simulink model "SIM_EXO_DAL_MN"  (R2021b)
(part 9 of 24)

t1621 = ct{452};
t1622 = ct{453};
t1623 = ct{454};
t1625 = ct{455};
t163 = ct{456};
t1631 = ct{457};
t1632 = ct{458};
t1633 = ct{459};
t1635 = ct{460};
t1636 = ct{461};
t1637 = ct{462};
t1638 = ct{463};
t1639 = ct{464};
t1641 = ct{465};
t1643 = ct{466};
t1644 = ct{467};
t1645 = ct{468};
t165 = ct{469};
t1650 = ct{470};
t1651 = ct{471};
t1652 = ct{472};
t1653 = ct{473};
t1657 = ct{474};
t1658 = ct{475};
t1659 = ct{476};
t166 = ct{477};
t1660 = ct{478};
t1661 = ct{479};
t1662 = ct{480};
t1663 = ct{481};
t1666 = ct{482};
t1669 = ct{483};
t1672 = ct{484};
t1676 = ct{485};
t168 = ct{486};
t1681 = ct{487};
t1682 = ct{488};
t1683 = ct{489};
t1687 = ct{490};
t1689 = ct{491};
t169 = ct{492};
t1692 = ct{493};
t1695 = ct{494};
t1696 = ct{495};
t1698 = ct{496};
t17 = ct{497};
t170 = ct{498};
t1702 = ct{499};
t1703 = ct{500};
t1704 = ct{501};
t1709 = ct{502};
t171 = ct{503};
t1711 = ct{504};
t1712 = ct{505};
t1713 = ct{506};
t1716 = ct{507};
t1720 = ct{508};
t1722 = ct{509};
t1726 = ct{510};
t1728 = ct{511};
t1729 = ct{512};
t173 = ct{513};
t1731 = ct{514};
t1733 = ct{515};
t1734 = ct{516};
t1735 = ct{517};
t1736 = ct{518};
t1737 = ct{519};
t1738 = ct{520};
t1740 = ct{521};
t1744 = ct{522};
t1745 = ct{523};
t1746 = ct{524};
t1749 = ct{525};
t175 = ct{526};
t1752 = ct{527};
t1755 = ct{528};
t1756 = ct{529};
t1757 = ct{530};
t1758 = ct{531};
t176 = ct{532};
t1760 = ct{533};
t1761 = ct{534};
t1764 = ct{535};
t1767 = ct{536};
t1769 = ct{537};
t177 = ct{538};
t1771 = ct{539};
t1772 = ct{540};
t1774 = ct{541};
t1776 = ct{542};
t1779 = ct{543};
t1784 = ct{544};
t1785 = ct{545};
t1786 = ct{546};
t1787 = ct{547};
t1788 = ct{548};
t1789 = ct{549};
t179 = ct{550};
t1793 = ct{551};
t1795 = ct{552};
t1797 = ct{553};
t1798 = ct{554};
t1799 = ct{555};
t18 = ct{556};
t180 = ct{557};
t1800 = ct{558};
t1801 = ct{559};
t1803 = ct{560};
t1804 = ct{561};
t1807 = ct{562};
t1808 = ct{563};
t1809 = ct{564};
t181 = ct{565};
t1810 = ct{566};
t1811 = ct{567};
t1812 = ct{568};
t1814 = ct{569};
t1816 = ct{570};
t1817 = ct{571};
t182 = ct{572};
t1820 = ct{573};
t1826 = ct{574};
t1827 = ct{575};
t1829 = ct{576};
t183 = ct{577};
t1830 = ct{578};
t1831 = ct{579};
t1832 = ct{580};
t1833 = ct{581};
t1834 = ct{582};
t1835 = ct{583};
t1836 = ct{584};
t1838 = ct{585};
t1847 = ct{586};
t1849 = ct{587};
t185 = ct{588};
t1850 = ct{589};
t1851 = ct{590};
t1855 = ct{591};
t1857 = ct{592};
t1858 = ct{593};
t1859 = ct{594};
t186 = ct{595};
t1866 = ct{596};
t1867 = ct{597};
t1871 = ct{598};
t1872 = ct{599};
t1873 = ct{600};
t1881 = ct{601};
t1882 = ct{602};
t1888 = ct{603};
t1889 = ct{604};
t1896 = ct{605};
t19 = ct{606};
t190 = ct{607};
t1903 = ct{608};
t1907 = ct{609};
t1908 = ct{610};
t191 = ct{611};
t1910 = ct{612};
t1911 = ct{613};
t1912 = ct{614};
t1913 = ct{615};
t1914 = ct{616};
t1915 = ct{617};
t1916 = ct{618};
t1920 = ct{619};
t1925 = ct{620};
t1926 = ct{621};
t193 = ct{622};
t1930 = ct{623};
t1935 = ct{624};
t1936 = ct{625};
t1937 = ct{626};
t1938 = ct{627};
t1939 = ct{628};
t194 = ct{629};
t1943 = ct{630};
t1944 = ct{631};
t1946 = ct{632};
t195 = ct{633};
t1950 = ct{634};
t1955 = ct{635};
t196 = ct{636};
t1961 = ct{637};
t1964 = ct{638};
t1965 = ct{639};
t1966 = ct{640};
t1967 = ct{641};
t1968 = ct{642};
t1969 = ct{643};
t197 = ct{644};
t1970 = ct{645};
t1972 = ct{646};
t1976 = ct{647};
t1977 = ct{648};
t1978 = ct{649};
t1979 = ct{650};
t198 = ct{651};
t1981 = ct{652};
t1984 = ct{653};
t1988 = ct{654};
t1992 = ct{655};
t1994 = ct{656};
t1995 = ct{657};
t1996 = ct{658};
t1997 = ct{659};
t1998 = ct{660};
t1999 = ct{661};
t2 = ct{662};
t20 = ct{663};
t2000 = ct{664};
t2001 = ct{665};
t2002 = ct{666};
t2003 = ct{667};
t2004 = ct{668};
t2005 = ct{669};
t2006 = ct{670};
t2014 = ct{671};
t2017 = ct{672};
t2019 = ct{673};
t2020 = ct{674};
t2023 = ct{675};
t2024 = ct{676};
t2028 = ct{677};
t2029 = ct{678};
t2033 = ct{679};
t2036 = ct{680};
t2037 = ct{681};
t2038 = ct{682};
t2042 = ct{683};
t2052 = ct{684};
t2053 = ct{685};
t2056 = ct{686};
t2058 = ct{687};
t2059 = ct{688};
t206 = ct{689};
t2060 = ct{690};
t2062 = ct{691};
t2065 = ct{692};
t2066 = ct{693};
t2067 = ct{694};
t2068 = ct{695};
t2069 = ct{696};
t207 = ct{697};
t2070 = ct{698};
t2072 = ct{699};
t2073 = ct{700};
t2074 = ct{701};
t2079 = ct{702};
t2081 = ct{703};
t2082 = ct{704};
t2083 = ct{705};
t2084 = ct{706};
t2085 = ct{707};
t2086 = ct{708};
t2087 = ct{709};
t2093 = ct{710};
t2094 = ct{711};
t2096 = ct{712};
t2097 = ct{713};
t2098 = ct{714};
t21 = ct{715};
t2100 = ct{716};
t2103 = ct{717};
t2104 = ct{718};
t2105 = ct{719};
t2106 = ct{720};
t2108 = ct{721};
t2109 = ct{722};
t2110 = ct{723};
t2111 = ct{724};
t2113 = ct{725};
t2114 = ct{726};
t2115 = ct{727};
t2116 = ct{728};
t2117 = ct{729};
t2118 = ct{730};
t2121 = ct{731};
t2122 = ct{732};
t2126 = ct{733};
t2128 = ct{734};
t2129 = ct{735};
t2130 = ct{736};
t2131 = ct{737};
t2132 = ct{738};
t2133 = ct{739};
t2136 = ct{740};
t2142 = ct{741};
t2144 = ct{742};
t2148 = ct{743};
t2149 = ct{744};
t215 = ct{745};
t2154 = ct{746};
t2156 = ct{747};
t2157 = ct{748};
t2158 = ct{749};
t216 = ct{750};
t2171 = ct{751};
t2172 = ct{752};
t2175 = ct{753};
t2176 = ct{754};
t2179 = ct{755};
t2180 = ct{756};
t2182 = ct{757};
t2189 = ct{758};
t219 = ct{759};
t2194 = ct{760};
t2196 = ct{761};
t22 = ct{762};
t220 = ct{763};
t2204 = ct{764};
t2208 = ct{765};
t221 = ct{766};
t2212 = ct{767};
t2214 = ct{768};
t2217 = ct{769};
t2218 = ct{770};
t2219 = ct{771};
t222 = ct{772};
t2220 = ct{773};
t2221 = ct{774};
t2223 = ct{775};
t2225 = ct{776};
t2227 = ct{777};
t2228 = ct{778};
t2229 = ct{779};
t223 = ct{780};
t2236 = ct{781};
t2239 = ct{782};
t224 = ct{783};
t2244 = ct{784};
t225 = ct{785};
t2251 = ct{786};
t2254 = ct{787};
t2256 = ct{788};
t2257 = ct{789};
t226 = ct{790};
t2264 = ct{791};
t2265 = ct{792};
t2266 = ct{793};
t2267 = ct{794};
t2269 = ct{795};
t227 = ct{796};
t2270 = ct{797};
t2274 = ct{798};
t2276 = ct{799};
t2277 = ct{800};
t2279 = ct{801};
t228 = ct{802};
t2280 = ct{803};
t2281 = ct{804};
t2282 = ct{805};
t2285 = ct{806};
t2291 = ct{807};
t2294 = ct{808};
t23 = ct{809};
t230 = ct{810};
t2302 = ct{811};
t2304 = ct{812};
t2305 = ct{813};
t2306 = ct{814};
t231 = ct{815};
t2316 = ct{816};
t2317 = ct{817};
t2318 = ct{818};
t2321 = ct{819};
t2322 = ct{820};
t2323 = ct{821};
t2324 = ct{822};
t233 = ct{823};
t2333 = ct{824};
t2336 = ct{825};
t2339 = ct{826};
t234 = ct{827};
t2340 = ct{828};
t2344 = ct{829};
t2348 = ct{830};
t235 = ct{831};
t2350 = ct{832};
t2357 = ct{833};
t2358 = ct{834};
t2359 = ct{835};
t236 = ct{836};
t2361 = ct{837};
t2362 = ct{838};
t2363 = ct{839};
t2364 = ct{840};
t2365 = ct{841};
t2366 = ct{842};
t2369 = ct{843};
t237 = ct{844};
t2371 = ct{845};
t2372 = ct{846};
t2373 = ct{847};
t2375 = ct{848};
t2376 = ct{849};
t2377 = ct{850};
t2378 = ct{851};
t2379 = ct{852};
t238 = ct{853};
t2384 = ct{854};
t2385 = ct{855};
t2387 = ct{856};
t2388 = ct{857};
t2389 = ct{858};
t239 = ct{859};
t2391 = ct{860};
t2394 = ct{861};
t24 = ct{862};
t240 = ct{863};
t2400 = ct{864};
t2401 = ct{865};
t2402 = ct{866};
t2403 = ct{867};
t2405 = ct{868};
t2406 = ct{869};
t2407 = ct{870};
t241 = ct{871};
t2410 = ct{872};
t2417 = ct{873};
t2418 = ct{874};
t2419 = ct{875};
t242 = ct{876};
t2421 = ct{877};
t2422 = ct{878};
t2428 = ct{879};
t2429 = ct{880};
t243 = ct{881};
t2430 = ct{882};
t2431 = ct{883};
t2434 = ct{884};
t2435 = ct{885};
t2437 = ct{886};
t2438 = ct{887};
t2439 = ct{888};
t244 = ct{889};
t2440 = ct{890};
t2441 = ct{891};
t2442 = ct{892};
t2443 = ct{893};
t2444 = ct{894};
t2447 = ct{895};
t2449 = ct{896};
t245 = ct{897};
t2450 = ct{898};
t2452 = ct{899};
t2453 = ct{900};
t2454 = ct{901};
t2455 = ct{902};
t2456 = ct{903};
t2457 = ct{904};
t2458 = ct{905};
t246 = ct{906};
t2460 = ct{907};
t2466 = ct{908};
t2467 = ct{909};
t2468 = ct{910};
t247 = ct{911};
t2470 = ct{912};
t2472 = ct{913};
t2474 = ct{914};
t2477 = ct{915};
t248 = ct{916};
t2481 = ct{917};
t2483 = ct{918};
t2484 = ct{919};
t2485 = ct{920};
t2486 = ct{921};
t2487 = ct{922};
t2489 = ct{923};
t249 = ct{924};
t2492 = ct{925};
t2495 = ct{926};
t2497 = ct{927};
t2498 = ct{928};
t2499 = ct{929};
t25 = ct{930};
t2500 = ct{931};
t2501 = ct{932};
t2502 = ct{933};
t2503 = ct{934};
t2504 = ct{935};
t2505 = ct{936};
t2506 = ct{937};
t2513 = ct{938};
t2518 = ct{939};
t2521 = ct{940};
t2527 = ct{941};
t253 = ct{942};
t2533 = ct{943};
t2535 = ct{944};
t2536 = ct{945};
t2537 = ct{946};
t2538 = ct{947};
t254 = ct{948};
t2540 = ct{949};
t2543 = ct{950};
t2544 = ct{951};
t2545 = ct{952};
t2546 = ct{953};
t2549 = ct{954};
t2551 = ct{955};
t2552 = ct{956};
t2553 = ct{957};
t2554 = ct{958};
t2555 = ct{959};
t2557 = ct{960};
t2558 = ct{961};
t2559 = ct{962};
t256 = ct{963};
t2560 = ct{964};
t2561 = ct{965};
t2562 = ct{966};
t2565 = ct{967};
t257 = ct{968};
t2572 = ct{969};
t2573 = ct{970};
t2574 = ct{971};
t2575 = ct{972};
t2576 = ct{973};
t2577 = ct{974};
t2578 = ct{975};
t2579 = ct{976};
t258 = ct{977};
t2583 = ct{978};
t2584 = ct{979};
t259 = ct{980};
t2590 = ct{981};
t2591 = ct{982};
t2592 = ct{983};
t2593 = ct{984};
t2595 = ct{985};
t2596 = ct{986};
t2597 = ct{987};
t26 = ct{988};
t260 = ct{989};
t2602 = ct{990};
t2603 = ct{991};
t2604 = ct{992};
t2605 = ct{993};
t2609 = ct{994};
t261 = ct{995};
t2610 = ct{996};
t2611 = ct{997};
t2615 = ct{998};
t2617 = ct{999};
t2627 = ct{1000};
t263 = ct{1001};
t264 = ct{1002};
t2652 = ct{1003};
t2655 = ct{1004};
t2656 = ct{1005};
t266 = ct{1006};
t2673 = ct{1007};
t2675 = ct{1008};
t2676 = ct{1009};
t2685 = ct{1010};
t2687 = ct{1011};
t269 = ct{1012};
t270 = ct{1013};
t2705 = ct{1014};
t2706 = ct{1015};
t2707 = ct{1016};
t2708 = ct{1017};
t2716 = ct{1018};
t2719 = ct{1019};
t272 = ct{1020};
t273 = ct{1021};
t274 = ct{1022};
t2749 = ct{1023};
t275 = ct{1024};
t2751 = ct{1025};
t2752 = ct{1026};
t276 = ct{1027};
t2764 = ct{1028};
t277 = ct{1029};
t278 = ct{1030};
t279 = ct{1031};
t280 = ct{1032};
t2804 = ct{1033};
t281 = ct{1034};
t284 = ct{1035};
t285 = ct{1036};
t2854 = ct{1037};
t286 = ct{1038};
t287 = ct{1039};
t288 = ct{1040};
t2886 = ct{1041};
t289 = ct{1042};
t29 = ct{1043};
t290 = ct{1044};
t291 = ct{1045};
t292 = ct{1046};
t293 = ct{1047};
t2939 = ct{1048};
t294 = ct{1049};
t296 = ct{1050};
t297 = ct{1051};
t299 = ct{1052};
t2997 = ct{1053};
t3 = ct{1054};
t30 = ct{1055};
t300 = ct{1056};
t302 = ct{1057};
t303 = ct{1058};
t304 = ct{1059};
t305 = ct{1060};
t3058 = ct{1061};
t306 = ct{1062};
t307 = ct{1063};
t308 = ct{1064};
t309 = ct{1065};
t31 = ct{1066};
t310 = ct{1067};
t311 = ct{1068};
t312 = ct{1069};
t313 = ct{1070};
t314 = ct{1071};
t3142 = ct{1072};
t315 = ct{1073};
t3158 = ct{1074};
t316 = ct{1075};
t318 = ct{1076};
t319 = ct{1077};
t3191 = ct{1078};
t32 = ct{1079};
t320 = ct{1080};
t3208 = ct{1081};
t321 = ct{1082};
t3211 = ct{1083};
t3212 = ct{1084};
t3218 = ct{1085};
t3219 = ct{1086};
t322 = ct{1087};
t3225 = ct{1088};
t3228 = ct{1089};
t3230 = ct{1090};
t3231 = ct{1091};
t324 = ct{1092};
t3243 = ct{1093};
t3244 = ct{1094};
t325 = ct{1095};
t3251 = ct{1096};
t3252 = ct{1097};
t3255 = ct{1098};
t3257 = ct{1099};
t3258 = ct{1100};
t3259 = ct{1101};
t3261 = ct{1102};
t3273 = ct{1103};
t3274 = ct{1104};
t3275 = ct{1105};
t3279 = ct{1106};
t328 = ct{1107};
t3282 = ct{1108};
t3286 = ct{1109};
t3288 = ct{1110};
t3289 = ct{1111};
t329 = ct{1112};
t3290 = ct{1113};
t3294 = ct{1114};
t3295 = ct{1115};
t33 = ct{1116};
t3309 = ct{1117};
t3314 = ct{1118};
t3317 = ct{1119};
t3319 = ct{1120};
t332 = ct{1121};
t3320 = ct{1122};
t3321 = ct{1123};
t3326 = ct{1124};
t3327 = ct{1125};
t3328 = ct{1126};
t3329 = ct{1127};
t333 = ct{1128};
t3330 = ct{1129};
t3331 = ct{1130};
t3333 = ct{1131};
t3334 = ct{1132};
t3335 = ct{1133};
t334 = ct{1134};
t3343 = ct{1135};
t336 = ct{1136};
t3363 = ct{1137};
t3364 = ct{1138};
t3365 = ct{1139};
t3367 = ct{1140};
t3368 = ct{1141};
t3369 = ct{1142};
t337 = ct{1143};
t3370 = ct{1144};
t3371 = ct{1145};
t3372 = ct{1146};
t3373 = ct{1147};
t3374 = ct{1148};
t3375 = ct{1149};
t3376 = ct{1150};
t3378 = ct{1151};
t3379 = ct{1152};
t3380 = ct{1153};
t3381 = ct{1154};
t3382 = ct{1155};
t3389 = ct{1156};
t3390 = ct{1157};
t3391 = ct{1158};
t3392 = ct{1159};
t3393 = ct{1160};
t3394 = ct{1161};
t3395 = ct{1162};
t3397 = ct{1163};
t34 = ct{1164};
t340 = ct{1165};
t3400 = ct{1166};
t3401 = ct{1167};
t3402 = ct{1168};
t3403 = ct{1169};
t3409 = ct{1170};
t341 = ct{1171};
t3416 = ct{1172};
t3417 = ct{1173};
t3418 = ct{1174};
t3419 = ct{1175};
t3420 = ct{1176};
t3426 = ct{1177};
t3430 = ct{1178};
t344 = ct{1179};
t345 = ct{1180};
t346 = ct{1181};
t347 = ct{1182};
t348 = ct{1183};
t349 = ct{1184};
t350 = ct{1185};
t352 = ct{1186};
t353 = ct{1187};
t354 = ct{1188};
t355 = ct{1189};
t356 = ct{1190};
t357 = ct{1191};
t358 = ct{1192};
t359 = ct{1193};
t360 = ct{1194};
t361 = ct{1195};
t362 = ct{1196};
t365 = ct{1197};
t366 = ct{1198};
t367 = ct{1199};
t368 = ct{1200};
t369 = ct{1201};
t371 = ct{1202};
t372 = ct{1203};
t373 = ct{1204};
t374 = ct{1205};
t375 = ct{1206};
t376 = ct{1207};
t377 = ct{1208};
t378 = ct{1209};
t379 = ct{1210};
t380 = ct{1211};
t382 = ct{1212};
t384 = ct{1213};
t386 = ct{1214};
t387 = ct{1215};
t388 = ct{1216};
t389 = ct{1217};
t391 = ct{1218};
t392 = ct{1219};
t395 = ct{1220};
t396 = ct{1221};
t398 = ct{1222};
t4 = ct{1223};
t400 = ct{1224};
t401 = ct{1225};
t402 = ct{1226};
t403 = ct{1227};
t404 = ct{1228};
t406 = ct{1229};
t409 = ct{1230};
t410 = ct{1231};
t411 = ct{1232};
t412 = ct{1233};
t413 = ct{1234};
t414 = ct{1235};
t415 = ct{1236};
t416 = ct{1237};
t417 = ct{1238};
t418 = ct{1239};
t419 = ct{1240};
t420 = ct{1241};
t421 = ct{1242};
t422 = ct{1243};
t423 = ct{1244};
t424 = ct{1245};
t425 = ct{1246};
t426 = ct{1247};
t427 = ct{1248};
t428 = ct{1249};
t429 = ct{1250};
t431 = ct{1251};
t432 = ct{1252};
t433 = ct{1253};
t434 = ct{1254};
t435 = ct{1255};
t436 = ct{1256};
t437 = ct{1257};
t438 = ct{1258};
t439 = ct{1259};
t44 = ct{1260};
t440 = ct{1261};
t441 = ct{1262};
t442 = ct{1263};
t443 = ct{1264};
t444 = ct{1265};
t445 = ct{1266};
t448 = ct{1267};
t449 = ct{1268};
t45 = ct{1269};
t450 = ct{1270};
t452 = ct{1271};
t453 = ct{1272};
t454 = ct{1273};
t457 = ct{1274};
t458 = ct{1275};
t459 = ct{1276};
t46 = ct{1277};
t460 = ct{1278};
t461 = ct{1279};
t462 = ct{1280};
t463 = ct{1281};
t464 = ct{1282};
t465 = ct{1283};
t466 = ct{1284};
t468 = ct{1285};
t469 = ct{1286};
t47 = ct{1287};
t470 = ct{1288};
t471 = ct{1289};
t472 = ct{1290};
t475 = ct{1291};
t4763 = ct{1292};
t477 = ct{1293};
t479 = ct{1294};
t480 = ct{1295};
t481 = ct{1296};
t482 = ct{1297};
t483 = ct{1298};
t484 = ct{1299};
t485 = ct{1300};
t486 = ct{1301};
t488 = ct{1302};
t489 = ct{1303};
t491 = ct{1304};
t492 = ct{1305};
t493 = ct{1306};
t494 = ct{1307};
t496 = ct{1308};
t497 = ct{1309};
t498 = ct{1310};
t499 = ct{1311};
t5 = ct{1312};
t50 = ct{1313};
t500 = ct{1314};
t501 = ct{1315};
t502 = ct{1316};
t503 = ct{1317};
t504 = ct{1318};
t505 = ct{1319};
t506 = ct{1320};
t507 = ct{1321};
t508 = ct{1322};
t509 = ct{1323};
t510 = ct{1324};
t511 = ct{1325};
t512 = ct{1326};
t513 = ct{1327};
t514 = ct{1328};
t516 = ct{1329};
t517 = ct{1330};
t518 = ct{1331};
t520 = ct{1332};
t521 = ct{1333};
t522 = ct{1334};
t523 = ct{1335};
t524 = ct{1336};
t525 = ct{1337};
t526 = ct{1338};
t527 = ct{1339};
t528 = ct{1340};
t529 = ct{1341};
t53 = ct{1342};
t530 = ct{1343};
t531 = ct{1344};
t532 = ct{1345};
t533 = ct{1346};
t534 = ct{1347};
t535 = ct{1348};
t536 = ct{1349};
t5361 = ct{1350};
t537 = ct{1351};
t538 = ct{1352};
t539 = ct{1353};
t540 = ct{1354};
t543 = ct{1355};
t544 = ct{1356};
t545 = ct{1357};
t546 = ct{1358};
t547 = ct{1359};
t548 = ct{1360};
t549 = ct{1361};
t551 = ct{1362};
t552 = ct{1363};
t553 = ct{1364};
t554 = ct{1365};
t555 = ct{1366};
t556 = ct{1367};
t557 = ct{1368};
t558 = ct{1369};
t559 = ct{1370};
t560 = ct{1371};
t561 = ct{1372};
t562 = ct{1373};
t563 = ct{1374};
t564 = ct{1375};
t567 = ct{1376};
t568 = ct{1377};
t569 = ct{1378};
t57 = ct{1379};
t570 = ct{1380};
t571 = ct{1381};
t572 = ct{1382};
t573 = ct{1383};
t574 = ct{1384};
t576 = ct{1385};
t577 = ct{1386};
t5777 = ct{1387};
t578 = ct{1388};
t579 = ct{1389};
t58 = ct{1390};
t580 = ct{1391};
t581 = ct{1392};
t582 = ct{1393};
t583 = ct{1394};
t584 = ct{1395};
t586 = ct{1396};
t587 = ct{1397};
t589 = ct{1398};
t59 = ct{1399};
t590 = ct{1400};
t591 = ct{1401};
t592 = ct{1402};
t593 = ct{1403};
t594 = ct{1404};
t595 = ct{1405};
t596 = ct{1406};
t597 = ct{1407};
t6 = ct{1408};
t60 = ct{1409};
t600 = ct{1410};
t602 = ct{1411};
t603 = ct{1412};
t604 = ct{1413};
t605 = ct{1414};
t609 = ct{1415};
t610 = ct{1416};
t611 = ct{1417};
t612 = ct{1418};
t613 = ct{1419};
t614 = ct{1420};
t615 = ct{1421};
t617 = ct{1422};
t618 = ct{1423};
t623 = ct{1424};
t625 = ct{1425};
t626 = ct{1426};
t629 = ct{1427};
t63 = ct{1428};
t633 = ct{1429};
t634 = ct{1430};
t638 = ct{1431};
t640 = ct{1432};
t643 = ct{1433};
t644 = ct{1434};
t655 = ct{1435};
t656 = ct{1436};
t660 = ct{1437};
t662 = ct{1438};
t663 = ct{1439};
t664 = ct{1440};
t665 = ct{1441};
t667 = ct{1442};
t668 = ct{1443};
t673 = ct{1444};
t674 = ct{1445};
t675 = ct{1446};
t676 = ct{1447};
t681 = ct{1448};
t682 = ct{1449};
t683 = ct{1450};
t685 = ct{1451};
t686 = ct{1452};
t687 = ct{1453};
t688 = ct{1454};
t689 = ct{1455};
t693 = ct{1456};
t694 = ct{1457};
t695 = ct{1458};
t696 = ct{1459};
t697 = ct{1460};
t698 = ct{1461};
t7 = ct{1462};
t700 = ct{1463};
t702 = ct{1464};
t703 = ct{1465};
t704 = ct{1466};
t705 = ct{1467};
t706 = ct{1468};
t71 = ct{1469};
t711 = ct{1470};
t713 = ct{1471};
t715 = ct{1472};
t716 = ct{1473};
t72 = ct{1474};
t724 = ct{1475};
t725 = ct{1476};
t727 = ct{1477};
t728 = ct{1478};
t73 = ct{1479};
t731 = ct{1480};
t733 = ct{1481};
t734 = ct{1482};
t735 = ct{1483};
t736 = ct{1484};
t74 = ct{1485};
t744 = ct{1486};
t746 = ct{1487};
t747 = ct{1488};
t748 = ct{1489};
t749 = ct{1490};
t75 = ct{1491};
t750 = ct{1492};
t751 = ct{1493};
t752 = ct{1494};
t755 = ct{1495};
t756 = ct{1496};
t757 = ct{1497};
t758 = ct{1498};
t759 = ct{1499};
t76 = ct{1500};
t762 = ct{1501};
t763 = ct{1502};
t764 = ct{1503};
t765 = ct{1504};
t766 = ct{1505};
t768 = ct{1506};
t769 = ct{1507};
t77 = ct{1508};
t772 = ct{1509};
t774 = ct{1510};
t775 = ct{1511};
t776 = ct{1512};
t780 = ct{1513};
t782 = ct{1514};
t785 = ct{1515};
t786 = ct{1516};
t788 = ct{1517};
t791 = ct{1518};
t793 = ct{1519};
t795 = ct{1520};
t8 = ct{1521};
t80 = ct{1522};
t804 = ct{1523};
t805 = ct{1524};
t806 = ct{1525};
t808 = ct{1526};
t81 = ct{1527};
t814 = ct{1528};
t815 = ct{1529};
t816 = ct{1530};
t818 = ct{1531};
t819 = ct{1532};
t82 = ct{1533};
t820 = ct{1534};
t821 = ct{1535};
t822 = ct{1536};
t825 = ct{1537};
t827 = ct{1538};
t83 = ct{1539};
t833 = ct{1540};
t834 = ct{1541};
t835 = ct{1542};
t836 = ct{1543};
t837 = ct{1544};
t838 = ct{1545};
t84 = ct{1546};
t840 = ct{1547};
t841 = ct{1548};
t842 = ct{1549};
t843 = ct{1550};
t846 = ct{1551};
t851 = ct{1552};
t855 = ct{1553};
t857 = ct{1554};
t86 = ct{1555};
t862 = ct{1556};
t864 = ct{1557};
t874 = ct{1558};
t880 = ct{1559};
t882 = ct{1560};
t884 = ct{1561};
t885 = ct{1562};
t888 = ct{1563};
t891 = ct{1564};
t892 = ct{1565};
t895 = ct{1566};
t897 = ct{1567};
t899 = ct{1568};
t9 = ct{1569};
t90 = ct{1570};
t900 = ct{1571};
t903 = ct{1572};
t904 = ct{1573};
t906 = ct{1574};
t91 = ct{1575};
t911 = ct{1576};
t921 = ct{1577};
t922 = ct{1578};
t923 = ct{1579};
t926 = ct{1580};
t927 = ct{1581};
t934 = ct{1582};
t935 = ct{1583};
t936 = ct{1584};
t937 = ct{1585};
t940 = ct{1586};
t941 = ct{1587};
t942 = ct{1588};
t946 = ct{1589};
t949 = ct{1590};
t95 = ct{1591};
t950 = ct{1592};
t956 = ct{1593};
t957 = ct{1594};
t958 = ct{1595};
t961 = ct{1596};
t962 = ct{1597};
t964 = ct{1598};
t965 = ct{1599};
t966 = ct{1600};
t968 = ct{1601};
t969 = ct{1602};
t97 = ct{1603};
t970 = ct{1604};
t971 = ct{1605};
t972 = ct{1606};
t977 = ct{1607};
t979 = ct{1608};
t982 = ct{1609};
t983 = ct{1610};
t984 = ct{1611};
t986 = ct{1612};
t987 = ct{1613};
t988 = ct{1614};
t989 = ct{1615};
t99 = ct{1616};
t993 = ct{1617};
t994 = ct{1618};
t995 = ct{1619};
t997 = ct{1620};
t999 = ct{1621};
t3432 = t3.*t5.*t8.*t9.*t34.*t191.*4.649924393989671e-23;
t3434 = t4.*t5.*t7.*t9.*t34.*t191.*9.299848787979342e-23;
t3435 = t5.*t7.*t8.*t9.*t34.*t191.*1.414846738462756e-22;
t3437 = t4.*t19.*t34.*t191.*7.821166634427942e-23;
t3438 = t4.*t24.*t34.*t191.*7.821166634427942e-23;
t3439 = t4.*t9.*t34.*t191.*2.079476307604284e-23;
t3440 = t4.*t9.*t34.*t191.*4.158952615208568e-23;
t3442 = t8.*t9.*t34.*t191.*4.158952615208568e-23;
t3443 = t101+t124+t139+t180;
t3444 = t108+t122+t141+t182;
t3445 = t3.*t4.*t5.*t8.*t34.*t191.*9.098517085411002e-23;
t3446 = t3.*t5.*t34.*t191.*(-2.472625392454631e-23);
t3447 = t4.*t5.*t7.*t34.*t191.*(-2.47393392290267e-21);
t3449 = t7.*t9.*t34.*t191.*(-2.472625392454631e-23);
t3450 = t3.*t4.*t19.*t34.*t191.*4.649924393989671e-23;
t3452 = t3.*t8.*t19.*t34.*t191.*1.414846738462756e-22;
t3453 = t4.*t7.*t19.*t34.*t191.*1.414846738462756e-22;
t3454 = t4.*t7.*t9.*t34.*t191.*(-2.47393392290267e-21);
t3455 = t5.*t7.*t8.*t34.*t191.*(-2.47393392290267e-21);
t3456 = t3.*t4.*t24.*t34.*t191.*4.649924393989671e-23;
t3459 = t7.*t8.*t24.*t34.*t191.*4.649924393989671e-23;
t3462 = t17.*t34.*t191.*3.230367166673482e-25;
t3463 = t18.*t19.*t34.*t191.*1.189885164369265e-22;
t3466 = t18.*t24.*t34.*t191.*1.189885164369265e-22;
t3468 = t9.*t18.*t34.*t191.*(-7.651846806710377e-23);
t3469 = t4.*t8.*t19.*t34.*t191.*1.564233326885588e-22;
t3470 = t5.*t9.*t18.*t34.*t191.*1.564233326885588e-22;
t3472 = t4.*t34.*t191.*3.002769355787804e-29;
t3473 = t8.*t34.*t191.*3.002769355787804e-29;
t3475 = t3.*t4.*t9.*t34.*t191.*1.236312696227316e-23;
t3477 = t3.*t5.*t8.*t34.*t191.*1.236312696227316e-23;
t3479 = t4.*t5.*t7.*t34.*t191.*1.236312696227316e-23;
t3481 = t5.*t8.*t34.*t191.*(-4.158952615208568e-23);
t3483 = t7.*t8.*t9.*t34.*t191.*1.236312696227316e-23;
t3486 = t4.*t17.*t34.*t191.*3.356793907564468e-24;
t3489 = t3.*t8.*t19.*t34.*t191.*(-7.074233692313782e-23);
t3492 = t3.*t9.*t34.*t191.*1.785238843466173e-29;
t3500 = t3.*t4.*t8.*t9.*t34.*t191.*4.945250784909262e-23;
t3501 = t4.*t8.*t9.*t34.*t191.*8.317905230417136e-23;
t3506 = t3.*t4.*t8.*t19.*t34.*t191.*9.299848787979342e-23;
t3507 = t4.*t7.*t8.*t19.*t34.*t191.*7.074233692313782e-23;
t3509 = t4.*t7.*t8.*t24.*t34.*t191.*7.074233692313782e-23;
t3514 = t102+t129+t150+t179;
t3515 = t117+t123+t153+t181;
t3516 = t3.*t8.*t34.*t191.*7.059909452387201e-23;
t3517 = t4.*t7.*t34.*t191.*7.059909452387201e-23;
t3519 = t3.*t9.*t34.*t191.*8.926194217330866e-30;
t3520 = t5.*t7.*t34.*t191.*8.926194217330866e-30;
t3521 = t7.*t18.*t19.*t34.*t191.*(-4.649924393989671e-23);
t3522 = t4.*t5.*t7.*t8.*t9.*t34.*t191.*(-9.299848787979342e-23);
t3523 = t130+t134+t152+t176;
t3524 = t8.*t9.*t34.*t191.*1.501384677893902e-29;
t3530 = t5.*t7.*t9.*t18.*t34.*t191.*(-7.074233692313782e-23);
t3532 = t4.*t17.*t34.*t191.*(-1.678396953782234e-24);
t3533 = t5.*t18.*t34.*t191.*(-4.158952615208568e-23);
t3534 = t3.*t4.*t5.*t34.*t191.*1.785238843466173e-29;
t3535 = t3.*t8.*t34.*t191.*3.5299547261936e-23;
t3538 = t4.*t7.*t9.*t34.*t191.*1.785238843466173e-29;
t3539 = t5.*t7.*t8.*t34.*t191.*1.785238843466173e-29;
t3541 = t4.*t34.*t191.*3.937746659416635e-29;
t3544 = t8.*t34.*t191.*3.937746659416635e-29;
t3546 = t8.*t9.*t34.*t191.*(-3.002769355787804e-29);
t3548 = t4.*t8.*t34.*t191.*5.632647031707275e-23;
t3549 = t4.*t5.*t7.*t8.*t34.*t191.*(-2.472625392454631e-23);
t3553 = t3.*t4.*t5.*t34.*t191.*8.926194217330866e-30;
t3556 = t4.*t7.*t9.*t34.*t191.*8.926194217330866e-30;
t3560 = t7.*t34.*t191.*1.323536528500358e-22;
t3568 = t3.*t9.*t18.*t34.*t191.*3.570477686932346e-29;
t3569 = t5.*t7.*t18.*t34.*t191.*1.785238843466173e-29;
t3572 = t2.*t4.*t190.*2.976937004352228e-6;
t3573 = t2.*t8.*t190.*2.976937004352228e-6;
t3574 = t9.*t18.*t34.*t191.*3.002769355787804e-29;
t3575 = t6.*t8.*t190.*2.976937004352228e-6;
t3576 = t9.*t23.*t34.*t191.*3.002769355787804e-29;
t3578 = t4.*t7.*t8.*t9.*t34.*t191.*3.570477686932346e-29;
t3579 = t5.*t8.*t34.*t191.*1.968873329708317e-29;
t3581 = t3.*t5.*t34.*t191.*1.170555820174774e-29;
t3582 = t3.*t5.*t34.*t191.*2.341111640349547e-29;
t3583 = t3.*t8.*t9.*t34.*t191.*(-8.926194217330866e-30);
t3584 = t5.*t7.*t8.*t34.*t191.*(-8.926194217330866e-30);
t3585 = t7.*t9.*t34.*t191.*1.170555820174774e-29;
t3590 = t6.*t8.*t190.*1.22799597575967e-5;
t3596 = t4.*t9.*t190.*3.508720606545093e-7;
t3597 = t5.*t8.*t190.*3.508720606545093e-7;
t3601 = t3.*t4.*t8.*t34.*t191.*3.34878210114812e-23;
t3602 = t4.*t190.*6.800564119502148e-6;
t3604 = t8.*t190.*6.800564119502148e-6;
t3607 = t7.*t18.*t34.*t191.*1.67439105057406e-23;
t3609 = t5.*t8.*t34.*t191.*(-3.937746659416635e-29);
t3613 = t7.*t23.*t34.*t191.*1.67439105057406e-23;
t3616 = t2.*t8.*t190.*1.22799597575967e-5;
t3617 = t4.*t6.*t190.*1.22799597575967e-5;
t3618 = t4.*t5.*t8.*t34.*t191.*(-3.002769355787804e-29);
t3622 = t2.*t8.*t190.*1.618032907912407e-6;
t3629 = t6.*t8.*t190.*1.618032907912407e-6;
t3630 = t4.*t190.*3.147703918772038e-6;
t3637 = t5.*t18.*t34.*t191.*3.937746659416635e-29;
t3638 = t4.*t190.*3.698217217635989e-4;
t3639 = t8.*t190.*3.147703918772038e-6;
t3641 = t5.*t23.*t34.*t191.*3.937746659416635e-29;
t3643 = t8.*t190.*3.698217217635989e-4;
t3646 = t4.*t5.*t34.*t191.*8.031026374039477e-30;
t3647 = t2.*t8.*t9.*t190.*1.488468502176114e-6;
t3649 = t4.*t6.*t9.*t190.*1.488468502176114e-6;
t3650 = t4.*t6.*t9.*t190.*2.976937004352228e-6;
t3652 = t4.*t9.*t34.*t191.*8.031026374039477e-30;
t3653 = t5.*t8.*t34.*t191.*8.031026374039477e-30;
t3654 = t8.*t9.*t34.*t191.*8.031026374039477e-30;
t3659 = t3.*t4.*t9.*t34.*t191.*1.170555820174774e-29;
t3660 = t3.*t4.*t9.*t34.*t191.*2.341111640349547e-29;
t3662 = t4.*t5.*t7.*t34.*t191.*1.170555820174774e-29;
t3663 = t4.*t5.*t7.*t34.*t191.*2.341111640349547e-29;
t3668 = t7.*t8.*t9.*t34.*t191.*2.341111640349547e-29;
t3676 = t2.*t4.*t190.*1.618032907912407e-6;
t3680 = t8.*t190.*3.696261130697717e-6;
t3682 = t3.*t5.*t18.*t34.*t191.*4.682223280699094e-29;
t3686 = t4.*t5.*t190.*1.907069379620846e-7;
t3691 = t4.*t190.*6.903101118415674e-6;
t3695 = t8.*t9.*t190.*1.907069379620846e-7;
t3697 = t8.*t190.*6.903101118415674e-6;
t3701 = t2.*t4.*t9.*t190.*(-2.976937004352228e-6);
t3709 = t5.*t6.*t8.*t190.*(-2.976937004352228e-6);
t3714 = t8.*t9.*t190.*3.400282059751074e-6;
t3716 = t2.*t8.*t190.*6.674437170347525e-6;
t3717 = t4.*t6.*t190.*6.674437170347525e-6;
t3722 = t6.*t8.*t190.*6.674437170347525e-6;
t3726 = t4.*t5.*t7.*t8.*t34.*t191.*4.682223280699094e-29;
t3729 = t3.*t4.*t5.*t34.*t191.*4.774692471202153e-30;
t3730 = t4.*t8.*t9.*t34.*t191.*(-3.937746659416635e-29);
t3736 = t3.*t4.*t9.*t34.*t191.*4.774692471202153e-30;
t3737 = t4.*t5.*t7.*t34.*t191.*4.774692471202153e-30;
t3738 = t3.*t5.*t8.*t34.*t191.*(-1.170555820174774e-29);
t3743 = t2.*t4.*t9.*t190.*6.139979878798348e-6;
t3744 = t2.*t4.*t9.*t190.*1.22799597575967e-5;
t3747 = t4.*t7.*t9.*t34.*t191.*4.774692471202153e-30;
t3748 = t5.*t7.*t8.*t34.*t191.*4.774692471202153e-30;
t3750 = t7.*t8.*t9.*t34.*t191.*4.774692471202153e-30;
t3751 = t6.*t8.*t9.*t190.*6.139979878798348e-6;
t3756 = t4.*t190.*3.696261130697717e-6;
t3774 = t7.*t9.*t18.*t34.*t191.*2.341111640349547e-29;
t3789 = t4.*t9.*t190.*(-6.800564119502148e-6);
t3798 = t8.*t190.*2.768890910755245e-7;
t3815 = t4.*t6.*t9.*t190.*(-1.22799597575967e-5);
t3822 = t2.*t5.*t8.*t190.*8.090164539562037e-7;
t3824 = t4.*t5.*t6.*t190.*8.090164539562037e-7;
t3825 = t4.*t5.*t6.*t190.*1.618032907912407e-6;
t3834 = t4.*t9.*t190.*(-3.698217217635989e-4);
t3835 = t5.*t8.*t190.*(-3.698217217635989e-4);
t3839 = t8.*t9.*t190.*(-3.698217217635989e-4);
t3846 = t2.*t4.*t5.*t190.*3.337218585173762e-6;
t3847 = t2.*t4.*t5.*t190.*6.674437170347525e-6;
t3852 = t5.*t6.*t8.*t190.*3.337218585173762e-6;
t3889 = t2.*t4.*t190.*2.349236299369594e-6;
t3892 = t2.*t5.*t8.*t190.*(-1.618032907912407e-6);
t3898 = t6.*t8.*t190.*2.349236299369594e-6;
t3899 = t6.*t8.*t9.*t190.*(-1.618032907912407e-6);
t3915 = t5.*t6.*t8.*t190.*(-6.674437170347525e-6);
t3950 = t5.*t8.*t190.*(-3.696261130697717e-6);
t3951 = t5.*t8.*t190.*1.848130565348858e-6;
t3958 = t2.*t8.*t190.*9.690674399615435e-6;
t3959 = t4.*t6.*t190.*9.690674399615435e-6;
t4001 = t3.*t18.*t34.*t191.*8.273795699471084e-23;
t4002 = t18.*t34.*t191.*6.958256670626673e-23;
t4004 = t23.*t34.*t191.*6.958256670626673e-23;
t4007 = t4.*t7.*t8.*t34.*t191.*8.273795699471084e-23;
t4028 = t2.*t4.*t5.*t190.*3.124456121473909e-13;
t4029 = t2.*t4.*t9.*t190.*3.124456121473909e-13;
t4030 = t2.*t5.*t8.*t190.*3.124456121473909e-13;
t4031 = t4.*t5.*t6.*t190.*3.124456121473909e-13;
t4032 = t2.*t8.*t9.*t190.*3.124456121473909e-13;
t4033 = t4.*t6.*t9.*t190.*3.124456121473909e-13;
t4039 = t2.*t4.*t5.*t190.*1.288848080425708e-12;
t4040 = t2.*t4.*t9.*t190.*1.288848080425708e-12;
t4041 = t4.*t5.*t6.*t190.*1.288848080425708e-12;
t4042 = t4.*t6.*t9.*t190.*1.288848080425708e-12;
t4043 = t5.*t6.*t8.*t190.*1.288848080425708e-12;
t4044 = t6.*t8.*t9.*t190.*1.288848080425708e-12;
t4045 = t4.*t5.*t190.*7.137559230037459e-13;
t4051 = t4.*t9.*t190.*7.137559230037459e-13;
t4052 = t5.*t8.*t190.*7.137559230037459e-13;
t4058 = t8.*t9.*t190.*7.137559230037459e-13;
t4105 = t4.*t190.*3.561623743745041e-7;
t4113 = t2.*t8.*t190.*3.021822113324163e-6;
t4114 = t4.*t6.*t190.*3.021822113324163e-6;
t4117 = t2.*t4.*t190.*1.246511225866906e-5;
t4118 = t6.*t8.*t190.*1.246511225866906e-5;
t4123 = (t498.*t1471)./2.0;
t4143 = t2.*t8.*t34.*t191.*2.473154649626116e-18;
t4144 = t4.*t34.*t191.*5.649715377798866e-18;
t4145 = t8.*t34.*t191.*5.649715377798866e-18;
t4150 = t3.*t34.*t191.*9.728063971071188e-18;
t4152 = t6.*t8.*t34.*t191.*1.020184153286453e-17;
t4153 = t9.*t34.*t191.*3.910360575273795e-23;
t4155 = t4.*t6.*t7.*t34.*t191.*6.065308926991484e-18;
t4160 = t2.*t4.*t7.*t34.*t191.*1.470366592725919e-18;
t4164 = t3.*t9.*t34.*t191.*4.531926220025415e-23;
t4165 = t5.*t7.*t34.*t191.*4.531926220025415e-23;
t4170 = t4.*t7.*t34.*t191.*9.728063971071188e-18;
t4174 = t7.*t8.*t34.*t191.*9.728063971071188e-18;
t4177 = t7.*t34.*t191.*6.343941833557992e-26;
t4178 = t3.*t7.*t34.*t191.*1.261825515365316e-22;
t4179 = t5.*t9.*t34.*t191.*7.993777824483687e-23;
t4180 = t4.*t9.*t34.*t191.*(-5.649715377798866e-18);
t4181 = t4.*t8.*t34.*t191.*1.628350277673685e-22;
t4182 = t2.*t3.*t4.*t34.*t191.*3.84506501891928e-22;
t4183 = t2.*t3.*t5.*t34.*t191.*1.92253250945964e-22;
t4184 = t2.*t3.*t5.*t34.*t191.*3.84506501891928e-22;
t4185 = t19.*t34.*t191.*6.080728160647903e-23;
t4186 = t2.*t3.*t8.*t34.*t191.*3.84506501891928e-22;
t4187 = t2.*t4.*t7.*t34.*t191.*3.84506501891928e-22;
t4188 = t3.*t4.*t6.*t34.*t191.*3.84506501891928e-22;
t4189 = t2.*t5.*t7.*t34.*t191.*3.84506501891928e-22;
t4190 = t24.*t34.*t191.*6.080728160647903e-23;
t4191 = t2.*t7.*t9.*t34.*t191.*3.84506501891928e-22;
t4192 = t3.*t6.*t9.*t34.*t191.*3.84506501891928e-22;
t4193 = t5.*t6.*t7.*t34.*t191.*1.92253250945964e-22;
t4194 = t5.*t6.*t7.*t34.*t191.*3.84506501891928e-22;
t4196 = t3.*t7.*t34.*t191.*1.458099973297124e-22;
t4197 = t2.*t3.*t34.*t191.*5.382450561195517e-25;
t4200 = t6.*t7.*t34.*t191.*5.382450561195517e-25;
t4203 = t2.*t3.*t4.*t34.*t191.*1.586101540900623e-21;
t4204 = t3.*t4.*t6.*t34.*t191.*1.586101540900623e-21;
t4205 = t2.*t3.*t9.*t34.*t191.*1.586101540900623e-21;
t4206 = t2.*t5.*t7.*t34.*t191.*7.930507704503114e-22;
t4207 = t2.*t5.*t7.*t34.*t191.*1.586101540900623e-21;
t4208 = t3.*t5.*t6.*t34.*t191.*7.930507704503114e-22;
t4209 = t3.*t5.*t6.*t34.*t191.*1.586101540900623e-21;
t4211 = t3.*t6.*t8.*t34.*t191.*1.586101540900623e-21;
t4212 = t4.*t6.*t7.*t34.*t191.*1.586101540900623e-21;
t4213 = t5.*t6.*t7.*t34.*t191.*1.586101540900623e-21;
t4214 = t6.*t7.*t9.*t34.*t191.*1.586101540900623e-21;
t4216 = t3.*t5.*t34.*t191.*2.463204881229188e-23;
t4221 = t18.*t34.*t191.*7.111824474586663e-23;
t4228 = t23.*t34.*t191.*7.111824474586663e-23;
t4229 = t7.*t9.*t34.*t191.*2.463204881229188e-23;
t4230 = t5.*t34.*t191.*2.125369829239315e-23;
t4231 = t3.*t4.*t34.*t191.*1.313343246602064e-21;
t4232 = t3.*t5.*t34.*t191.*6.566716233010318e-22;
t4233 = t3.*t5.*t34.*t191.*1.313343246602064e-21;
t4235 = t3.*t8.*t34.*t191.*1.313343246602064e-21;
t4236 = t4.*t7.*t34.*t191.*1.313343246602064e-21;
t4237 = t5.*t7.*t34.*t191.*1.313343246602064e-21;
t4239 = t7.*t9.*t34.*t191.*6.566716233010318e-22;
t4240 = t7.*t9.*t34.*t191.*1.313343246602064e-21;
t4242 = t3.*t4.*t5.*t34.*t191.*4.531926220025415e-23;
t4243 = t7.*t8.*t34.*t191.*5.099405807101157e-25;
t4246 = t2.*t3.*t4.*t34.*t191.*2.089880210625419e-22;
t4249 = t2.*t3.*t4.*t9.*t34.*t191.*1.92253250945964e-22;
t4255 = t9.*t18.*t34.*t191.*7.82072115054759e-23;
t4256 = t2.*t3.*t8.*t34.*t191.*2.089880210625419e-22;
t4257 = t2.*t4.*t7.*t34.*t191.*2.089880210625419e-22;
t4258 = t3.*t4.*t6.*t34.*t191.*2.089880210625419e-22;
t4259 = t2.*t3.*t9.*t34.*t191.*1.044940105312709e-22;
t4260 = t2.*t3.*t9.*t34.*t191.*2.089880210625419e-22;
t4261 = t2.*t5.*t7.*t34.*t191.*2.089880210625419e-22;
t4262 = t3.*t5.*t6.*t34.*t191.*2.089880210625419e-22;
t4265 = t2.*t7.*t9.*t34.*t191.*2.089880210625419e-22;
t4266 = t2.*t7.*t8.*t9.*t34.*t191.*1.92253250945964e-22;
t4268 = t3.*t6.*t8.*t9.*t34.*t191.*1.92253250945964e-22;
t4271 = t6.*t7.*t9.*t34.*t191.*1.044940105312709e-22;
t4272 = t6.*t7.*t9.*t34.*t191.*2.089880210625419e-22;
t4275 = t7.*t8.*t9.*t34.*t191.*(-9.728063971071188e-18);
t4277 = t4.*t7.*t9.*t34.*t191.*2.324829770052718e-23;
t4278 = t3.*t5.*t7.*t34.*t191.*7.82072115054759e-23;
t4279 = t4.*t5.*t8.*t34.*t191.*1.564144230109518e-22;
t4283 = t3.*t4.*t34.*t191.*7.142096628897415e-20;
t4284 = t3.*t5.*t34.*t191.*7.142096628897415e-20;
t4287 = t3.*t8.*t34.*t191.*7.142096628897415e-20;
t4288 = t4.*t7.*t34.*t191.*7.142096628897415e-20;
t4289 = t3.*t9.*t34.*t191.*7.142096628897415e-20;
t4290 = t5.*t7.*t34.*t191.*7.142096628897415e-20;
t4292 = t2.*t7.*t34.*t191.*2.220277963292577e-24;
t4293 = t3.*t6.*t34.*t191.*2.220277963292577e-24;
t4294 = t7.*t9.*t34.*t191.*7.142096628897415e-20;
t4295 = t3.*t8.*t34.*t191.*7.138318981153782e-22;
t4296 = t4.*t7.*t34.*t191.*7.138318981153782e-22;
t4297 = t3.*t9.*t34.*t191.*7.138318981153782e-22;
t4298 = t5.*t7.*t34.*t191.*7.138318981153782e-22;
t4299 = t3.*t4.*t34.*t191.*6.078930528964336e-22;
t4300 = t4.*t5.*t7.*t34.*t191.*1.263597807995354e-23;
t4301 = t2.*t3.*t8.*t9.*t34.*t191.*7.930507704503114e-22;
t4304 = t3.*t4.*t6.*t9.*t34.*t191.*7.930507704503114e-22;
t4308 = t3.*t4.*t34.*t191.*1.442682849549919e-24;
t4309 = t7.*t9.*t34.*t191.*7.138318981153782e-22;
t4310 = t3.*t8.*t34.*t191.*6.078930528964336e-22;
t4311 = t4.*t7.*t34.*t191.*6.078930528964336e-22;
t4313 = t6.*t7.*t8.*t9.*t34.*t191.*7.930507704503114e-22;
t4315 = t2.*t3.*t4.*t9.*t34.*t191.*(-3.84506501891928e-22);
t4316 = t2.*t4.*t5.*t7.*t34.*t191.*(-3.84506501891928e-22);
t4317 = t9.*t17.*t34.*t191.*(-3.910360575273795e-23);
t4319 = t2.*t3.*t4.*t34.*t191.*8.620822290548326e-22;
t4320 = t2.*t3.*t5.*t34.*t191.*8.620822290548326e-22;
t4321 = t3.*t4.*t9.*t34.*t191.*2.463204881229188e-23;
t4323 = t2.*t3.*t8.*t9.*t34.*t191.*(-3.84506501891928e-22);
t4325 = t3.*t4.*t6.*t34.*t191.*8.620822290548326e-22;
t4326 = t2.*t7.*t8.*t9.*t34.*t191.*(-3.84506501891928e-22);
t4328 = t3.*t6.*t8.*t9.*t34.*t191.*(-3.84506501891928e-22);
t4330 = t5.*t6.*t7.*t8.*t34.*t191.*(-3.84506501891928e-22);
t4333 = t3.*t6.*t8.*t34.*t191.*8.620822290548326e-22;
t4334 = t4.*t6.*t7.*t34.*t191.*8.620822290548326e-22;
t4335 = t2.*t7.*t9.*t34.*t191.*4.310411145274163e-22;
t4336 = t2.*t7.*t9.*t34.*t191.*8.620822290548326e-22;
t4337 = t3.*t6.*t9.*t34.*t191.*4.310411145274163e-22;
t4338 = t3.*t6.*t9.*t34.*t191.*8.620822290548326e-22;
t4339 = t5.*t6.*t7.*t34.*t191.*8.620822290548326e-22;
t4341 = t6.*t7.*t9.*t34.*t191.*8.620822290548326e-22;
t4342 = t7.*t18.*t34.*t191.*4.426946542131316e-23;
t4343 = t3.*t4.*t34.*t191.*1.333145467812469e-21;
t4344 = t7.*t23.*t34.*t191.*4.426946542131316e-23;
t4345 = t3.*t4.*t34.*t191.*4.663711344199015e-25;
t4346 = t3.*t8.*t34.*t191.*1.333145467812469e-21;
t4347 = t3.*t4.*t9.*t34.*t191.*6.566716233010318e-22;
t4351 = t4.*t5.*t7.*t34.*t191.*6.566716233010318e-22;
t4353 = t4.*t5.*t7.*t9.*t34.*t191.*4.752547061531711e-23;
t4355 = t7.*t8.*t34.*t191.*1.333145467812469e-21;
t4361 = t3.*t4.*t5.*t34.*t191.*2.126195753400915e-23;
t4365 = t3.*t4.*t34.*t191.*7.138318981153782e-22;
t4367 = t2.*t3.*t4.*t5.*t34.*t191.*1.044940105312709e-22;
t4369 = t3.*t9.*t34.*t191.*3.569159490576891e-22;
t4370 = t5.*t7.*t34.*t191.*3.569159490576891e-22;
t4371 = t3.*t4.*t6.*t9.*t34.*t191.*(-1.586101540900623e-21);
t4372 = t4.*t5.*t6.*t7.*t34.*t191.*(-1.586101540900623e-21);
t4375 = t3.*t4.*t34.*t191.*3.576348967607797e-23;
t4377 = t3.*t6.*t8.*t9.*t34.*t191.*(-1.586101540900623e-21);
t4379 = t3.*t5.*t8.*t9.*t34.*t191.*1.344552364866272e-22;
t4382 = t2.*t5.*t7.*t8.*t34.*t191.*1.044940105312709e-22;
t4385 = t3.*t5.*t6.*t8.*t34.*t191.*1.044940105312709e-22;
t4387 = t6.*t7.*t8.*t9.*t34.*t191.*(-1.586101540900623e-21);
t4390 = t3.*t8.*t19.*t34.*t191.*2.045555332665541e-22;
t4391 = t7.*t8.*t34.*t191.*3.576348967607797e-23;
t4392 = t7.*t34.*t191.*3.464776426798696e-24;
t4394 = t3.*t7.*t19.*t34.*t191.*1.598755564896737e-22;
t4395 = t4.*t8.*t19.*t34.*t191.*1.598755564896737e-22;
t4396 = t5.*t9.*t17.*t34.*t191.*1.598755564896737e-22;
t4397 = t5.*t9.*t18.*t34.*t191.*1.598755564896737e-22;
t4401 = t3.*t5.*t8.*t34.*t191.*(-2.463204881229188e-23);
t4402 = t3.*t7.*t18.*t34.*t191.*8.141751388368425e-23;
t4403 = t4.*t8.*t17.*t34.*t191.*8.141751388368425e-23;
t4404 = t4.*t7.*t19.*t34.*t191.*7.230360259287513e-23;
t4405 = t3.*t7.*t9.*t34.*t191.*4.25073965847863e-23;
t4406 = t4.*t8.*t9.*t34.*t191.*8.501479316957259e-23;
t4407 = t17.*t34.*t191.*8.254151403776931e-26;
t4408 = t3.*t4.*t5.*t8.*t34.*t191.*4.649659540105436e-23;
t4410 = t22.*t34.*t191.*8.254151403776931e-26;
t4411 = t3.*t8.*t9.*t34.*t191.*6.577221276854549e-23;
t4412 = t3.*t4.*t5.*t9.*t34.*t191.*1.32251930673679e-22;
t4413 = t3.*t7.*t8.*t34.*t191.*8.577193772324431e-25;
t4417 = t3.*t5.*t7.*t8.*t34.*t191.*3.910360575273795e-23;
t4419 = t17.*t19.*t34.*t191.*1.216145632129581e-22;
t4420 = t18.*t19.*t34.*t191.*1.216145632129581e-22;
t4421 = t3.*t4.*t9.*t34.*t191.*(-1.313343246602064e-21);
t4422 = t4.*t5.*t7.*t34.*t191.*(-1.313343246602064e-21);
t4425 = t3.*t5.*t7.*t9.*t34.*t191.*2.432291264259161e-22;
t4426 = t4.*t5.*t8.*t9.*t34.*t191.*2.432291264259161e-22;
t4428 = t17.*t24.*t34.*t191.*1.216145632129581e-22;
t4429 = t18.*t24.*t34.*t191.*1.216145632129581e-22;
t4431 = t4.*t7.*t8.*t34.*t191.*7.733880651525396e-23;
t4432 = t3.*t8.*t9.*t34.*t191.*(-1.313343246602064e-21);
t4435 = t7.*t8.*t9.*t34.*t191.*(-1.313343246602064e-21);
t4436 = t7.*t8.*t9.*t34.*t191.*(-6.566716233010318e-22);
t4440 = t5.*t18.*t34.*t191.*4.25073965847863e-23;
t4442 = t2.*t3.*t4.*t5.*t34.*t191.*(-1.586101540900623e-21);
t4443 = t3.*t34.*t191.*5.751467996178103e-23;
t4444 = t4.*t17.*t34.*t191.*8.577193772324431e-25;
t4445 = t2.*t34.*t191.*4.965121091065431e-29;
t4446 = t4.*t22.*t34.*t191.*8.577193772324431e-25;
t4448 = t6.*t34.*t191.*2.048128230484517e-28;
t4449 = t7.*t34.*t191.*1.298466651472986e-21;
t4450 = t7.*t34.*t191.*1.298466651472986e-21;
t4452 = t3.*t4.*t9.*t34.*t191.*1.155635706310448e-23;
t4453 = t6.*t7.*t34.*t191.*2.01292161617043e-21;
t4455 = t2.*t4.*t7.*t9.*t34.*t191.*(-2.089880210625419e-22);
t4457 = t2.*t3.*t5.*t8.*t34.*t191.*4.310411145274163e-22;
t4459 = t3.*t4.*t5.*t6.*t34.*t191.*4.310411145274163e-22;
t4462 = t5.*t7.*t18.*t34.*t191.*4.252391506801831e-23;
t4464 = t6.*t7.*t8.*t9.*t34.*t191.*(-2.089880210625419e-22);
t4469 = t5.*t7.*t23.*t34.*t191.*4.252391506801831e-23;
t4473 = t5.*t6.*t7.*t8.*t34.*t191.*4.310411145274163e-22;
t4478 = t3.*t4.*t19.*t34.*t191.*4.346488293565505e-23;
t4479 = t2.*t3.*t8.*t34.*t191.*3.034315574254804e-22;
t4480 = t2.*t4.*t7.*t34.*t191.*3.034315574254804e-22;
t4481 = t3.*t4.*t6.*t34.*t191.*3.034315574254804e-22;
t4483 = t2.*t7.*t34.*t191.*4.879772380631159e-22;
t4484 = t3.*t6.*t34.*t191.*4.879772380631159e-22;
t4485 = t3.*t4.*t24.*t34.*t191.*4.346488293565505e-23;
t4486 = t8.*t17.*t34.*t191.*1.231254336368264e-25;
t4488 = t8.*t22.*t34.*t191.*1.231254336368264e-25;
t4491 = t6.*t7.*t8.*t34.*t191.*3.034315574254804e-22;
t4492 = t3.*t9.*t34.*t191.*9.123193089563036e-30;
t4493 = t3.*t4.*t7.*t9.*t34.*t191.*(-3.910360575273795e-23);
t4495 = t17.*t18.*t34.*t191.*3.555912237293331e-23;
t4498 = t3.*t4.*t7.*t8.*t34.*t191.*7.111824474586663e-23;
t4501 = t17.*t23.*t34.*t191.*3.555912237293331e-23;
t4502 = t3.*t8.*t34.*t191.*6.694747686175631e-26;
t4504 = t3.*t8.*t9.*t34.*t191.*(-7.142096628897415e-20);
t4506 = t4.*t7.*t8.*t9.*t34.*t191.*4.252391506801831e-23;
t4508 = t7.*t8.*t9.*t34.*t191.*(-7.142096628897415e-20);
t4509 = t3.*t4.*t7.*t34.*t191.*1.231254336368264e-25;
t4513 = t3.*t4.*t8.*t9.*t34.*t191.*2.527195615990709e-23;
t4516 = t3.*t4.*t8.*t19.*t34.*t191.*4.752547061531711e-23;
t4517 = t2.*t3.*t34.*t191.*2.01292161617043e-21;
t4519 = t4.*t7.*t8.*t24.*t34.*t191.*6.612596533683948e-23;
t4520 = t5.*t7.*t9.*t23.*t34.*t191.*6.612596533683948e-23;
t4522 = t3.*t7.*t8.*t19.*t34.*t191.*7.993777824483687e-23;
t4524 = t2.*t3.*t4.*t9.*t34.*t191.*(-8.620822290548326e-22);
t4525 = t2.*t3.*t5.*t8.*t34.*t191.*(-8.620822290548326e-22);
t4530 = t3.*t7.*t8.*t24.*t34.*t191.*7.993777824483687e-23;
t4532 = t4.*t6.*t7.*t9.*t34.*t191.*(-8.620822290548326e-22);
t4533 = t3.*t5.*t8.*t34.*t191.*3.57486922061625e-23;
t4540 = t4.*t7.*t34.*t191.*3.607859943485489e-23;
t4542 = t4.*t7.*t34.*t191.*6.914158210327463e-23;
t4543 = t8.*t19.*t22.*t34.*t191.*1.216145632129581e-22;
t4547 = t3.*t4.*t5.*t8.*t9.*t34.*t191.*7.230360259287513e-23;
t4548 = t3.*t4.*t5.*t34.*t191.*3.569159490576891e-22;
t4549 = t4.*t5.*t7.*t8.*t9.*t34.*t191.*8.69297658713101e-23;
t4551 = t4.*t5.*t8.*t17.*t34.*t191.*7.82072115054759e-23;
t4554 = t4.*t7.*t9.*t34.*t191.*(-7.138318981153782e-22);
t4555 = t4.*t7.*t9.*t34.*t191.*3.569159490576891e-22;
t4557 = t4.*t7.*t8.*t19.*t34.*t191.*6.612596533683948e-23;
t4558 = t5.*t7.*t9.*t18.*t34.*t191.*6.612596533683948e-23;
t4559 = t3.*t4.*t7.*t19.*t34.*t191.*1.216145632129581e-22;
t4561 = t4.*t7.*t34.*t191.*7.324723241820617e-22;
t4562 = t34.*t191.*1.614743896654871e-25;
t4563 = t2.*t3.*t4.*t34.*t191.*1.251664818208198e-21;
t4566 = t5.*t8.*t9.*t17.*t34.*t191.*(-7.993777824483687e-23);
t4567 = t3.*t8.*t34.*t191.*1.020706698179709e-22;
t4568 = t4.*t5.*t8.*t34.*t191.*3.069039723904487e-29;
t4569 = t2.*t7.*t8.*t34.*t191.*1.251664818208198e-21;
t4570 = t3.*t6.*t8.*t34.*t191.*1.251664818208198e-21;
t4571 = t4.*t6.*t7.*t34.*t191.*1.251664818208198e-21;
t4572 = t3.*t7.*t8.*t9.*t34.*t191.*2.125369829239315e-23;
t4574 = t5.*t7.*t8.*t34.*t191.*9.123193089563036e-30;
t4575 = t7.*t9.*t18.*t34.*t191.*2.311271412620895e-23;
t4577 = t3.*t5.*t7.*t8.*t9.*t34.*t191.*(-2.432291264259161e-22);
t4579 = t3.*t5.*t34.*t191.*1.196389694146674e-29;
t4581 = t7.*t9.*t23.*t34.*t191.*2.311271412620895e-23;
t4582 = t3.*t8.*t34.*t191.*1.036418850630278e-21;
t4583 = t4.*t7.*t34.*t191.*1.036418850630278e-21;
t4584 = t3.*t4.*t5.*t7.*t9.*t34.*t191.*(-7.993777824483687e-23);
t4588 = t9.*t18.*t34.*t191.*3.069039723904487e-29;
t4589 = t7.*t18.*t19.*t34.*t191.*4.346488293565505e-23;
t4590 = t9.*t23.*t34.*t191.*3.069039723904487e-29;
t4591 = t7.*t19.*t23.*t34.*t191.*4.346488293565505e-23;
t4595 = t5.*t7.*t34.*t191.*8.343705270104849e-30;
t4596 = t4.*t5.*t7.*t8.*t34.*t191.*2.311271412620895e-23;
t4600 = t8.*t17.*t34.*t191.*6.068415617284221e-23;
t4601 = t8.*t22.*t34.*t191.*6.068415617284221e-23;
t4605 = t4.*t8.*t34.*t191.*5.756958141897304e-23;
t4606 = t3.*t7.*t18.*t19.*t34.*t191.*7.993777824483687e-23;
t4607 = t4.*t8.*t17.*t19.*t34.*t191.*7.993777824483687e-23;
t4611 = t3.*t4.*t5.*t34.*t191.*2.581060362977273e-29;
t4614 = t4.*t8.*t9.*t17.*t34.*t191.*4.25073965847863e-23;
t4616 = t3.*t4.*t7.*t34.*t191.*6.068415617284221e-23;
t4617 = t5.*t8.*t22.*t34.*t191.*(-2.125369829239315e-23);
t4621 = t3.*t5.*t7.*t9.*t18.*t34.*t191.*1.216145632129581e-22;
t4622 = t4.*t5.*t8.*t9.*t17.*t34.*t191.*1.216145632129581e-22;
t4625 = t3.*t4.*t7.*t9.*t34.*t191.*1.534519861952243e-29;
t4626 = t3.*t5.*t7.*t8.*t34.*t191.*1.534519861952243e-29;
t4628 = t7.*t9.*t34.*t191.*1.094169869929701e-29;
t4629 = t3.*t34.*t191.*4.303986245035329e-23;
t4630 = t3.*t4.*t8.*t34.*t191.*1.711344441975548e-23;
t4632 = t7.*t8.*t9.*t34.*t191.*1.196389694146674e-29;
t4633 = t4.*t5.*t17.*t34.*t191.*1.534519861952243e-29;
t4634 = t3.*t7.*t34.*t191.*1.933613622435097e-22;
t4636 = t4.*t5.*t22.*t34.*t191.*1.534519861952243e-29;
t4637 = t2.*t3.*t5.*t34.*t191.*4.035603346078089e-29;
t4638 = t2.*t190.*4.797002992829487e-5;
t4639 = t2.*t3.*t9.*t34.*t191.*4.035603346078089e-29;
t4640 = t2.*t5.*t7.*t34.*t191.*4.035603346078089e-29;
t4641 = t2.*t7.*t9.*t34.*t191.*4.035603346078089e-29;
t4642 = t5.*t6.*t7.*t34.*t191.*4.035603346078089e-29;
t4643 = t3.*t9.*t18.*t34.*t191.*1.824638617912607e-29;
t4644 = t17.*t18.*t19.*t34.*t191.*(-6.080728160647903e-23);
t4645 = t3.*t8.*t9.*t34.*t191.*8.343705270104849e-30;
t4646 = t6.*t7.*t9.*t34.*t191.*4.035603346078089e-29;
t4647 = t3.*t4.*t8.*t34.*t191.*1.150475340336206e-23;
t4649 = t2.*t5.*t7.*t34.*t191.*1.664699206432988e-28;
t4650 = t3.*t5.*t6.*t34.*t191.*1.664699206432988e-28;
t4651 = t2.*t7.*t9.*t34.*t191.*1.664699206432988e-28;
t4652 = t3.*t6.*t9.*t34.*t191.*1.664699206432988e-28;
t4653 = t5.*t6.*t7.*t34.*t191.*1.664699206432988e-28;
t4656 = t5.*t7.*t18.*t34.*t191.*1.66874105402097e-29;
t4657 = t3.*t5.*t34.*t191.*1.378424649377201e-28;
t4658 = t6.*t7.*t9.*t34.*t191.*1.664699206432988e-28;
t4660 = t4.*t8.*t9.*t34.*t191.*4.024651742608185e-29;
t4661 = t3.*t9.*t34.*t191.*1.378424649377201e-28;
t4662 = t5.*t7.*t34.*t191.*1.378424649377201e-28;
t4663 = t7.*t9.*t34.*t191.*1.378424649377201e-28;
t4666 = t5.*t18.*t34.*t191.*4.024651742608185e-29;
t4667 = t5.*t23.*t34.*t191.*4.024651742608185e-29;
t4669 = t4.*t7.*t8.*t9.*t34.*t191.*3.337482108041939e-29;
t4672 = t6.*t190.*1.978778980640035e-4;
t4673 = t5.*t17.*t18.*t34.*t191.*(-2.125369829239315e-23);
t4674 = t3.*t4.*t7.*t8.*t9.*t34.*t191.*3.069039723904487e-29;
t4675 = t9.*t17.*t23.*t34.*t191.*1.534519861952243e-29;
t4688 = t3.*t5.*t6.*t8.*t34.*t191.*4.035603346078089e-29;
t4691 = t3.*t6.*t8.*t9.*t34.*t191.*4.035603346078089e-29;
t4692 = t3.*t5.*t18.*t34.*t191.*2.392779388293348e-29;
t4693 = t3.*t4.*t9.*t34.*t191.*3.384729434006076e-29;
t4694 = t7.*t18.*t34.*t191.*1.565126759819563e-23;
C_dq = ft_5({dq1,dq2,dq3,dq4,dq5,dq6,t1003,t1004,t1006,t1008,t101,t1012,t1013,t1015,t1016,t102,t1023,t1024,t1025,t1026,t1027,t1028,t1030,t1032,t1033,t1034,t1038,t1039,t104,t1040,t1041,t1042,t1043,t1044,t1045,t1047,t1048,t1049,t1050,t1051,t1054,t1055,t1056,t1057,t1058,t1059,t106,t1061,t1062,t1063,t1064,t1065,t1066,t1068,t1069,t107,t1070,t1071,t1073,t1078,t1080,t1081,t1083,t1084,t1085,t109,t1091,t1092,t1093,t1094,t1095,t1097,t1098,t1099,t110,t1100,t1101,t1102,t1105,t1106,t1108,t1109,t111,t1111,t1113,t1115,t1116,t1119,t112,t1123,t1125,t1126,t1127,t1128,t1129,t113,t1130,t1131,t1132,t1133,t1134,t1138,t1139,t114,t1140,t1141,t1144,t115,t1150,t1151,t1152,t1153,t1155,t1158,t1159,t116,t1161,t1162,t1163,t1166,t1167,t1169,t1170,t1171,t1173,t1174,t1175,t1176,t1177,t1178,t1179,t118,t1180,t1181,t1182,t1183,t1185,t1186,t1187,t1188,t1189,t1190,t1191,t1192,t1193,t1195,t1196,t1197,t1198,t1199,t120,t1203,t1204,t1205,t1206,t1207,t1208,t121,t1210,t1214,t1215,t1216,t1219,t1221,t1222,t1223,t1224,t1225,t1226,t1229,t1230,t1232,t1233,t1236,t124,t1240,t1242,t1244,t1245,t125,t1250,t1251,t1253,t1254,t1256,t1257,t1258,t1259,t126,t1260,t1261,t1262,t1263,t1264,t1266,t1272,t1273,t1274,t1276,t1278,t1279,t128,t1280,t1282,t1284,t1285,t1286,t1287,t1288,t129,t1290,t1293,t1294,t1295,t1296,t1297,t1298,t1299,t130,t1300,t1301,t1302,t1304,t1306,t1307,t1308,t1309,t131,t1312,t1313,t1315,t1316,t1319,t132,t1320,t1321,t1322,t1323,t1324,t1325,t1326,t1328,t1329,t133,t1330,t1331,t1332,t1333,t1335,t1337,t1338,t1339,t134,t1340,t1341,t1342,t1343,t1344,t1345,t1346,t1347,t1348,t135,t1351,t1352,t1353,t1354,t1355,t1356,t1358,t136,t1360,t1362,t1364,t1365,t1366,t1367,t1368,t1369,t1370,t1371,t1372,t1373,t1374,t1375,t1377,t1378,t1379,t1380,t1382,t1383,t1384,t1385,t1386,t1387,t1388,t1389,t139,t1391,t1392,t1393,t1394,t1397,t1398,t1399,t140,t1401,t1402,t1403,t1404,t1405,t1406,t1407,t1408,t1409,t141,t1410,t1411,t1413,t1414,t1415,t1416,t1417,t1418,t1419,t142,t1421,t1423,t1424,t1426,t1427,t1428,t1429,t143,t1431,t1433,t1434,t1435,t1436,t144,t1440,t1443,t1444,t1445,t1447,t1448,t1449,t145,t1451,t1453,t1454,t1456,t1457,t1460,t1461,t1463,t1464,t1469,t147,t1470,t1471,t1472,t1473,t1475,t1476,t1478,t1479,t148,t1481,t1482,t1483,t1485,t1486,t1487,t1488,t1489,t1494,t1496,t1497,t15,t150,t1501,t1503,t1505,t151,t1513,t1514,t1515,t1517,t1518,t1519,t152,t1520,t1521,t1522,t1523,t1527,t1528,t1529,t153,t1531,t1532,t1533,t1535,t154,t1541,t1542,t1545,t1548,t1549,t155,t1550,t1555,t1556,t1558,t156,t1560,t1561,t1562,t1566,t1567,t1568,t1569,t157,t1570,t1571,t158,t1580,t1587,t1589,t1591,t1593,t1595,t1596,t1597,t1598,t1599,t16,t1605,t1606,t161,t1610,t1611,t1612,t1619,t162,t1620,t1621,t1622,t1623,t1625,t163,t1631,t1632,t1633,t1635,t1636,t1637,t1638,t1639,t1641,t1643,t1644,t1645,t165,t1650,t1651,t1652,t1653,t1657,t1658,t1659,t166,t1660,t1661,t1662,t1663,t1666,t1669,t1672,t1676,t168,t1681,t1682,t1683,t1687,t1689,t169,t1692,t1695,t1696,t1698,t17,t170,t1702,t1703,t1704,t1709,t171,t1711,t1712,t1713,t1716,t1720,t1722,t1726,t1728,t1729,t173,t1731,t1733,t1734,t1735,t1736,t1737,t1738,t1740,t1744,t1745,t1746,t1749,t175,t1752,t1755,t1756,t1757,t1758,t1760,t1761,t1764,t1767,t1769,t177,t1771,t1772,t1774,t1776,t1779,t1784,t1785,t1786,t1787,t1788,t1789,t179,t1793,t1795,t1797,t1798,t1799,t18,t180,t1800,t1801,t1803,t1804,t1807,t1808,t1809,t181,t1810,t1811,t1812,t1814,t1816,t1817,t182,t1820,t1826,t1827,t1829,t183,t1830,t1831,t1832,t1833,t1834,t1835,t1836,t1838,t1847,t1849,t185,t1850,t1851,t1855,t1857,t1858,t1859,t186,t1866,t1867,t1871,t1872,t1873,t1881,t1882,t1888,t1889,t1896,t19,t190,t1903,t1907,t1908,t191,t1910,t1911,t1912,t1913,t1914,t1915,t1916,t1920,t1925,t1926,t193,t1930,t1935,t1936,t1937,t1938,t1939,t194,t1943,t1944,t1946,t195,t1950,t1955,t196,t1961,t1964,t1965,t1966,t1967,t1968,t1969,t197,t1970,t1972,t1976,t1977,t1978,t1979,t198,t1981,t1984,t1988,t1992,t1994,t1995,t1996,t1997,t1998,t1999,t2,t20,t2000,t2001,t2002,t2003,t2004,t2005,t2006,t2014,t2017,t2019,t2020,t2023,t2024,t2028,t2029,t2033,t2036,t2037,t2038,t2042,t2052,t2053,t2056,t2058,t2059,t206,t2060,t2062,t2065,t2066,t2067,t2068,t2069,t207,t2070,t2072,t2073,t2074,t2079,t2081,t2082,t2083,t2084,t2085,t2086,t2087,t2093,t2094,t2096,t2097,t2098,t21,t2100,t2103,t2104,t2105,t2106,t2108,t2109,t2110,t2111,t2113,t2114,t2115,t2116,t2117,t2118,t2121,t2122,t2126,t2128,t2129,t2130,t2131,t2132,t2133,t2136,t2142,t2144,t2148,t2149,t215,t2154,t2156,t2157,t2158,t216,t2171,t2172,t2175,t2176,t2179,t2180,t2182,t2189,t219,t2194,t2196,t22,t220,t2204,t2208,t221,t2212,t2214,t2217,t2218,t2219,t222,t2220,t2221,t2223,t2225,t2227,t2228,t2229,t223,t2236,t2239,t224,t2244,t225,t2251,t2254,t2256,t2257,t226,t2264,t2265,t2266,t2267,t2269,t227,t2270,t2274,t2276,t2277,t2279,t228,t2280,t2281,t2282,t2285,t2291,t2294,t23,t230,t2302,t2304,t2305,t2306,t231,t2316,t2317,t2318,t2321,t2322,t2323,t2324,t233,t2333,t2336,t2339,t234,t2340,t2344,t2348,t235,t2350,t2357,t2358,t2359,t236,t2361,t2362,t2363,t2364,t2365,t2366,t2369,t237,t2371,t2372,t2373,t2375,t2376,t2377,t2378,t2379,t238,t2384,t2385,t2387,t2388,t2389,t239,t2391,t2394,t24,t240,t2400,t2401,t2402,t2403,t2405,t2406,t2407,t241,t2410,t2417,t2418,t2419,t242,t2421,t2422,t2428,t2429,t243,t2430,t2431,t2434,t2435,t2437,t2438,t2439,t244,t2440,t2441,t2442,t2443,t2444,t2447,t2449,t245,t2450,t2452,t2453,t2454,t2455,t2456,t2457,t2458,t246,t2460,t2466,t2467,t2468,t247,t2470,t2472,t2474,t2477,t248,t2481,t2483,t2484,t2485,t2486,t2487,t2489,t249,t2492,t2495,t2497,t2498,t2499,t25,t2500,t2501,t2502,t2503,t2504,t2505,t2506,t2513,t2518,t2521,t2527,t253,t2533,t2535,t2536,t2537,t2538,t254,t2540,t2543,t2544,t2545,t2546,t2549,t2551,t2552,t2553,t2554,t2555,t2557,t2558,t2559,t256,t2560,t2561,t2562,t2565,t257,t2572,t2573,t2574,t2575,t2576,t2577,t2578,t2579,t258,t2583,t2584,t259,t2590,t2591,t2592,t2593,t2595,t2596,t2597,t26,t260,t2602,t2603,t2604,t2605,t2609,t261,t2610,t2611,t2615,t2617,t2627,t263,t264,t2652,t2655,t2656,t266,t2673,t2675,t2676,t2685,t2687,t269,t270,t2705,t2706,t2707,t2708,t2716,t2719,t272,t273,t274,t2749,t275,t2751,t2752,t276,t2764,t277,t278,t279,t280,t2804,t281,t284,t285,t2854,t286,t287,t288,t2886,t289,t29,t290,t291,t292,t293,t2939,t294,t296,t297,t299,t2997,t3,t30,t300,t302,t303,t304,t305,t3058,t306,t307,t308,t309,t31,t310,t311,t312,t313,t314,t3142,t315,t3158,t316,t318,t319,t3191,t32,t320,t3208,t321,t3211,t3212,t3218,t3219,t322,t3225,t3228,t3230,t3231,t324,t3243,t3244,t325,t3251,t3252,t3255,t3257,t3258,t3259,t3261,t3273,t3274,t3275,t3279,t328,t3282,t3286,t3288,t3289,t329,t3290,t3294,t3295,t33,t3309,t3314,t3317,t3319,t332,t3320,t3321,t3326,t3327,t3328,t3329,t333,t3330,t3331,t3333,t3334,t3335,t334,t3343,t336,t3363,t3364,t3365,t3367,t3368,t3369,t337,t3370,t3371,t3372,t3373,t3374,t3375,t3376,t3378,t3379,t3380,t3381,t3382,t3389,t3390,t3391,t3392,t3393,t3394,t3395,t3397,t34,t340,t3400,t3401,t3402,t3403,t3409,t341,t3416,t3417,t3418,t3419,t3420,t3426,t3430,t3432,t3434,t3435,t3437,t3438,t3439,t344,t3440,t3442,t3443,t3444,t3445,t3446,t3447,t3449,t345,t3450,t3452,t3453,t3454,t3455,t3456,t3459,t346,t3462,t3463,t3466,t3468,t3469,t347,t3470,t3472,t3473,t3475,t3477,t3479,t348,t3481,t3483,t3486,t3489,t349,t3492,t350,t3500,t3501,t3506,t3507,t3509,t3514,t3515,t3516,t3517,t3519,t352,t3520,t3521,t3522,t3523,t3524,t353,t3530,t3532,t3533,t3534,t3535,t3538,t3539,t354,t3541,t3544,t3546,t3548,t3549,t355,t3553,t3556,t356,t3560,t3568,t3569,t357,t3572,t3573,t3574,t3575,t3576,t3578,t3579,t358,t3581,t3582,t3583,t3584,t3585,t359,t3590,t3596,t3597,t360,t3601,t3602,t3604,t3607,t3609,t361,t3613,t3616,t3617,t3618,t362,t3622,t3629,t3630,t3637,t3638,t3639,t3641,t3643,t3646,t3647,t3649,t365,t3650,t3652,t3653,t3654,t3659,t366,t3660,t3662,t3663,t3668,t367,t3676,t368,t3680,t3682,t3686,t369,t3691,t3695,t3697,t3701,t3709,t371,t3714,t3716,t3717,t372,t3722,t3726,t3729,t373,t3730,t3736,t3737,t3738,t374,t3743,t3744,t3747,t3748,t375,t3750,t3751,t3756,t376,t377,t3774,t378,t3789,t379,t3798,t380,t3815,t382,t3822,t3824,t3825,t3834,t3835,t3839,t384,t3846,t3847,t3852,t386,t387,t388,t3889,t389,t3892,t3898,t3899,t391,t3915,t392,t395,t3950,t3951,t3958,t3959,t396,t398,t4,t400,t4001,t4002,t4004,t4007,t401,t402,t4028,t4029,t403,t4030,t4031,t4032,t4033,t4039,t404,t4040,t4041,t4042,t4043,t4044,t4045,t4051,t4052,t4058,t406,t409,t410,t4105,t411,t4113,t4114,t4117,t4118,t412,t4123,t413,t414,t4143,t4144,t4145,t415,t4150,t4152,t4153,t4155,t416,t4160,t4164,t4165,t417,t4170,t4174,t4177,t4178,t4179,t418,t4180,t4181,t4182,t4183,t4184,t4185,t4186,t4187,t4188,t4189,t419,t4190,t4191,t4192,t4193,t4194,t4196,t4197,t420,t4200,t4203,t4204,t4205,t4206,t4207,t4208,t4209,t421,t4211,t4212,t4213,t4214,t4216,t422,t4221,t4228,t4229,t423,t4230,t4231,t4232,t4233,t4235,t4236,t4237,t4239,t424,t4240,t4242,t4243,t4246,t4249,t425,t4255,t4256,t4257,t4258,t4259,t426,t4260,t4261,t4262,t4265,t4266,t4268,t427,t4271,t4272,t4275,t4277,t4278,t4279,t428,t4283,t4284,t4287,t4288,t4289,t429,t4290,t4292,t4293,t4294,t4295,t4296,t4297,t4298,t4299,t4300,t4301,t4304,t4308,t4309,t431,t4310,t4311,t4313,t4315,t4316,t4317,t4319,t432,t4320,t4321,t4323,t4325,t4326,t4328,t433,t4330,t4333,t4334,t4335,t4336,t4337,t4338,t4339,t434,t4341,t4342,t4343,t4344,t4345,t4346,t4347,t435,t4351,t4353,t4355,t436,t4361,t4365,t4367,t4369,t437,t4370,t4371,t4372,t4375,t4377,t4379,t438,t4382,t4385,t4387,t439,t4390,t4391,t4392,t4394,t4395,t4396,t4397,t44,t440,t4401,t4402,t4403,t4404,t4405,t4406,t4407,t4408,t441,t4410,t4411,t4412,t4413,t4417,t4419,t442,t4420,t4421,t4422,t4425,t4426,t4428,t4429,t443,t4431,t4432,t4435,t4436,t444,t4440,t4442,t4443,t4444,t4445,t4446,t4448,t4449,t445,t4450,t4452,t4453,t4455,t4457,t4459,t4462,t4464,t4469,t4473,t4478,t4479,t448,t4480,t4481,t4483,t4484,t4485,t4486,t4488,t449,t4491,t4492,t4493,t4495,t4498,t45,t450,t4501,t4502,t4504,t4506,t4508,t4509,t4513,t4516,t4517,t4519,t452,t4520,t4522,t4524,t4525,t453,t4530,t4532,t4533,t454,t4540,t4542,t4543,t4547,t4548,t4549,t4551,t4554,t4555,t4557,t4558,t4559,t4561,t4562,t4563,t4566,t4567,t4568,t4569,t457,t4570,t4571,t4572,t4574,t4575,t4577,t4579,t458,t4581,t4582,t4583,t4584,t4588,t4589,t459,t4590,t4591,t4595,t4596,t46,t460,t4600,t4601,t4605,t4606,t4607,t461,t4611,t4614,t4616,t4617,t462,t4621,t4622,t4625,t4626,t4628,t4629,t463,t4630,t4632,t4633,t4634,t4636,t4637,t4638,t4639,t464,t4640,t4641,t4642,t4643,t4644,t4645,t4646,t4647,t4649,t465,t4650,t4651,t4652,t4653,t4656,t4657,t4658,t466,t4660,t4661,t4662,t4663,t4666,t4667,t4669,t4672,t4673,t4674,t4675,t468,t4688,t469,t4691,t4692,t4693,t4694,t47,t470,t471,t472,t475,t4763,t477,t479,t480,t481,t482,t483,t484,t485,t486,t488,t489,t491,t492,t493,t494,t496,t497,t498,t499,t5,t50,t500,t501,t502,t503,t504,t505,t506,t507,t508,t509,t510,t511,t512,t513,t514,t516,t517,t518,t520,t521,t522,t523,t524,t525,t526,t527,t528,t529,t53,t530,t531,t532,t533,t534,t535,t536,t5361,t537,t538,t539,t540,t543,t544,t545,t546,t547,t548,t549,t551,t552,t553,t554,t555,t556,t557,t558,t559,t560,t561,t562,t563,t564,t567,t568,t569,t57,t570,t571,t572,t573,t574,t576,t577,t5777,t578,t579,t58,t580,t581,t582,t583,t584,t586,t587,t589,t59,t590,t591,t592,t593,t594,t595,t596,t597,t6,t60,t600,t602,t603,t604,t605,t609,t610,t611,t612,t613,t614,t615,t617,t618,t623,t625,t626,t629,t63,t633,t634,t638,t640,t643,t644,t655,t656,t660,t662,t663,t664,t665,t667,t668,t673,t674,t675,t676,t681,t682,t683,t685,t686,t687,t688,t689,t693,t694,t695,t696,t697,t698,t7,t700,t702,t703,t704,t705,t706,t71,t711,t713,t715,t716,t72,t724,t725,t727,t728,t73,t731,t733,t734,t735,t736,t74,t744,t746,t747,t748,t749,t75,t750,t751,t752,t755,t756,t757,t758,t759,t76,t762,t763,t764,t765,t766,t768,t769,t77,t772,t774,t775,t776,t780,t782,t785,t786,t788,t791,t793,t795,t8,t80,t804,t805,t806,t808,t81,t814,t815,t816,t818,t819,t82,t820,t821,t822,t825,t827,t83,t833,t834,t835,t836,t837,t838,t84,t840,t841,t842,t843,t846,t851,t855,t857,t86,t862,t864,t874,t880,t882,t884,t885,t888,t891,t892,t895,t897,t899,t9,t90,t900,t903,t904,t906,t91,t911,t921,t922,t923,t926,t927,t934,t935,t936,t937,t940,t941,t942,t946,t949,t95,t950,t956,t957,t958,t961,t962,t964,t965,t966,t968,t969,t97,t970,t971,t972,t977,t979,t982,t983,t984,t986,t987,t988,t989,t99,t993,t994,t995,t997,t999});
end
function C_dq = ft_5(ct)
dq1 = ct{1};
dq2 = ct{2};
dq3 = ct{3};
dq4 = ct{4};
dq5 = ct{5};
dq6 = ct{6};
t1003 = ct{7};
t1004 = ct{8};
t1006 = ct{9};
t1008 = ct{10};
t101 = ct{11};
t1012 = ct{12};
t1013 = ct{13};
t1015 = ct{14};
t1016 = ct{15};
t102 = ct{16};
t1023 = ct{17};
t1024 = ct{18};
t1025 = ct{19};
t1026 = ct{20};
t1027 = ct{21};
t1028 = ct{22};
t1030 = ct{23};
t1032 = ct{24};
t1033 = ct{25};
t1034 = ct{26};
t1038 = ct{27};
t1039 = ct{28};
t104 = ct{29};
t1040 = ct{30};
t1041 = ct{31};
t1042 = ct{32};
t1043 = ct{33};
t1044 = ct{34};
t1045 = ct{35};
t1047 = ct{36};
t1048 = ct{37};
t1049 = ct{38};
t1050 = ct{39};
t1051 = ct{40};
t1054 = ct{41};
t1055 = ct{42};
t1056 = ct{43};
t1057 = ct{44};
t1058 = ct{45};
t1059 = ct{46};
t106 = ct{47};
t1061 = ct{48};
t1062 = ct{49};
t1063 = ct{50};
t1064 = ct{51};
t1065 = ct{52};
t1066 = ct{53};
t1068 = ct{54};
t1069 = ct{55};
t107 = ct{56};
t1070 = ct{57};
t1071 = ct{58};
t1073 = ct{59};
t1078 = ct{60};
t1080 = ct{61};
t1081 = ct{62};
t1083 = ct{63};
t1084 = ct{64};
t1085 = ct{65};
t109 = ct{66};
t1091 = ct{67};
t1092 = ct{68};
t1093 = ct{69};
t1094 = ct{70};
t1095 = ct{71};
t1097 = ct{72};
t1098 = ct{73};
t1099 = ct{74};
t110 = ct{75};
t1100 = ct{76};
t1101 = ct{77};
t1102 = ct{78};
t1105 = ct{79};
t1106 = ct{80};
t1108 = ct{81};
t1109 = ct{82};
t111 = ct{83};
t1111 = ct{84};
t1113 = ct{85};
t1115 = ct{86};
t1116 = ct{87};
t1119 = ct{88};
t112 = ct{89};
t1123 = ct{90};
t1125 = ct{91};
t1126 = ct{92};
t1127 = ct{93};
t1128 = ct{94};
t1129 = ct{95};
t113 = ct{96};
t1130 = ct{97};
t1131 = ct{98};
t1132 = ct{99};
t1133 = ct{100};
t1134 = ct{101};
t1138 = ct{102};
t1139 = ct{103};
t114 = ct{104};
t1140 = ct{105};
t1141 = ct{106};
t1144 = ct{107};
t115 = ct{108};
t1150 = ct{109};
t1151 = ct{110};
t1152 = ct{111};
t1153 = ct{112};
t1155 = ct{113};
t1158 = ct{114};
t1159 = ct{115};
t116 = ct{116};
t1161 = ct{117};
t1162 = ct{118};
t1163 = ct{119};
t1166 = ct{120};
t1167 = ct{121};
t1169 = ct{122};
t1170 = ct{123};
t1171 = ct{124};
t1173 = ct{125};
t1174 = ct{126};
t1175 = ct{127};
t1176 = ct{128};
t1177 = ct{129};
t1178 = ct{130};
t1179 = ct{131};
t118 = ct{132};
t1180 = ct{133};
t1181 = ct{134};
t1182 = ct{135};
t1183 = ct{136};
t1185 = ct{137};
t1186 = ct{138};
t1187 = ct{139};
t1188 = ct{140};
t1189 = ct{141};
t1190 = ct{142};
t1191 = ct{143};
t1192 = ct{144};
t1193 = ct{145};
t1195 = ct{146};
t1196 = ct{147};
t1197 = ct{148};
t1198 = ct{149};
t1199 = ct{150};
t120 = ct{151};
t1203 = ct{152};
t1204 = ct{153};
t1205 = ct{154};
t1206 = ct{155};
t1207 = ct{156};
t1208 = ct{157};
t121 = ct{158};
t1210 = ct{159};
t1214 = ct{160};
t1215 = ct{161};
t1216 = ct{162};
t1219 = ct{163};
t1221 = ct{164};
t1222 = ct{165};
t1223 = ct{166};
t1224 = ct{167};
t1225 = ct{168};
t1226 = ct{169};
t1229 = ct{170};
t1230 = ct{171};
t1232 = ct{172};
t1233 = ct{173};
t1236 = ct{174};
t124 = ct{175};
t1240 = ct{176};
t1242 = ct{177};
t1244 = ct{178};
t1245 = ct{179};
t125 = ct{180};
t1250 = ct{181};
t1251 = ct{182};
t1253 = ct{183};
t1254 = ct{184};
t1256 = ct{185};
t1257 = ct{186};
t1258 = ct{187};
t1259 = ct{188};
t126 = ct{189};
t1260 = ct{190};
t1261 = ct{191};
t1262 = ct{192};
t1263 = ct{193};
t1264 = ct{194};
t1266 = ct{195};
t1272 = ct{196};
t1273 = ct{197};
t1274 = ct{198};
t1276 = ct{199};
t1278 = ct{200};
t1279 = ct{201};
t128 = ct{202};
t1280 = ct{203};
t1282 = ct{204};
t1284 = ct{205};
t1285 = ct{206};
t1286 = ct{207};
t1287 = ct{208};
t1288 = ct{209};
t129 = ct{210};
t1290 = ct{211};
t1293 = ct{212};
t1294 = ct{213};
t1295 = ct{214};
t1296 = ct{215};
t1297 = ct{216};
t1298 = ct{217};
t1299 = ct{218};
t130 = ct{219};
t1300 = ct{220};
t1301 = ct{221};
t1302 = ct{222};
t1304 = ct{223};
t1306 = ct{224};
t1307 = ct{225};
t1308 = ct{226};
t1309 = ct{227};
t131 = ct{228};
t1312 = ct{229};
t1313 = ct{230};
t1315 = ct{231};
t1316 = ct{232};
t1319 = ct{233};
t132 = ct{234};
t1320 = ct{235};
t1321 = ct{236};
t1322 = ct{237};
t1323 = ct{238};
t1324 = ct{239};
t1325 = ct{240};
t1326 = ct{241};
t1328 = ct{242};
t1329 = ct{243};
t133 = ct{244};
t1330 = ct{245};
t1331 = ct{246};
t1332 = ct{247};
t1333 = ct{248};
t1335 = ct{249};
t1337 = ct{250};
t1338 = ct{251};
t1339 = ct{252};
t134 = ct{253};
t1340 = ct{254};
t1341 = ct{255};
t1342 = ct{256};
t1343 = ct{257};
t1344 = ct{258};
t1345 = ct{259};
t1346 = ct{260};
t1347 = ct{261};
t1348 = ct{262};
t135 = ct{263};
t1351 = ct{264};
t1352 = ct{265};
t1353 = ct{266};
t1354 = ct{267};
t1355 = ct{268};
t1356 = ct{269};
t1358 = ct{270};
t136 = ct{271};
t1360 = ct{272};
t1362 = ct{273};
t1364 = ct{274};
t1365 = ct{275};
t1366 = ct{276};
t1367 = ct{277};
t1368 = ct{278};
t1369 = ct{279};
t1370 = ct{280};
t1371 = ct{281};
t1372 = ct{282};
t1373 = ct{283};
t1374 = ct{284};
t1375 = ct{285};
t1377 = ct{286};
t1378 = ct{287};
t1379 = ct{288};
t1380 = ct{289};
t1382 = ct{290};
t1383 = ct{291};
t1384 = ct{292};
t1385 = ct{293};
t1386 = ct{294};
t1387 = ct{295};
t1388 = ct{296};
t1389 = ct{297};
t139 = ct{298};
t1391 = ct{299};
t1392 = ct{300};
t1393 = ct{301};
t1394 = ct{302};
t1397 = ct{303};
t1398 = ct{304};
t1399 = ct{305};
t140 = ct{306};
t1401 = ct{307};
t1402 = ct{308};
t1403 = ct{309};
t1404 = ct{310};
t1405 = ct{311};
t1406 = ct{312};
t1407 = ct{313};
t1408 = ct{314};
t1409 = ct{315};
t141 = ct{316};
t1410 = ct{317};
t1411 = ct{318};
t1413 = ct{319};
t1414 = ct{320};
t1415 = ct{321};
t1416 = ct{322};
t1417 = ct{323};
t1418 = ct{324};
t1419 = ct{325};
t142 = ct{326};
t1421 = ct{327};
t1423 = ct{328};
t1424 = ct{329};
t1426 = ct{330};
t1427 = ct{331};
t1428 = ct{332};
t1429 = ct{333};
t143 = ct{334};
t1431 = ct{335};
t1433 = ct{336};
t1434 = ct{337};
t1435 = ct{338};
t1436 = ct{339};
t144 = ct{340};
t1440 = ct{341};
t1443 = ct{342};
t1444 = ct{343};
t1445 = ct{344};
t1447 = ct{345};
t1448 = ct{346};
t1449 = ct{347};
t145 = ct{348};
t1451 = ct{349};
t1453 = ct{350};
t1454 = ct{351};
t1456 = ct{352};
t1457 = ct{353};
t1460 = ct{354};
t1461 = ct{355};
t1463 = ct{356};
t1464 = ct{357};
t1469 = ct{358};
t147 = ct{359};
t1470 = ct{360};
t1471 = ct{361};
t1472 = ct{362};
t1473 = ct{363};
t1475 = ct{364};
t1476 = ct{365};
t1478 = ct{366};
t1479 = ct{367};
t148 = ct{368};
t1481 = ct{369};
t1482 = ct{370};
t1483 = ct{371};
t1485 = ct{372};
t1486 = ct{373};
t1487 = ct{374};
t1488 = ct{375};
t1489 = ct{376};
t1494 = ct{377};
t1496 = ct{378};
t1497 = ct{379};
t15 = ct{380};
t150 = ct{381};
t1501 = ct{382};
t1503 = ct{383};
t1505 = ct{384};
t151 = ct{385};
t1513 = ct{386};
t1514 = ct{387};
t1515 = ct{388};
t1517 = ct{389};
t1518 = ct{390};
t1519 = ct{391};
t152 = ct{392};
t1520 = ct{393};
t1521 = ct{394};
t1522 = ct{395};
t1523 = ct{396};
t1527 = ct{397};
t1528 = ct{398};
t1529 = ct{399};
t153 = ct{400};
t1531 = ct{401};
t1532 = ct{402};
t1533 = ct{403};
t1535 = ct{404};
t154 = ct{405};
t1541 = ct{406};
t1542 = ct{407};
t1545 = ct{408};
t1548 = ct{409};
t1549 = ct{410};
t155 = ct{411};
t1550 = ct{412};
t1555 = ct{413};
t1556 = ct{414};
t1558 = ct{415};
t156 = ct{416};
t1560 = ct{417};
t1561 = ct{418};
t1562 = ct{419};
t1566 = ct{420};
t1567 = ct{421};
t1568 = ct{422};
t1569 = ct{423};
t157 = ct{424};
t1570 = ct{425};
t1571 = ct{426};
t158 = ct{427};
t1580 = ct{428};
t1587 = ct{429};
t1589 = ct{430};
t1591 = ct{431};
t1593 = ct{432};
t1595 = ct{433};
t1596 = ct{434};
t1597 = ct{435};
t1598 = ct{436};
t1599 = ct{437};
t16 = ct{438};
t1605 = ct{439};
t1606 = ct{440};
t161 = ct{441};
t1610 = ct{442};
t1611 = ct{443};
t1612 = ct{444};
t1619 = ct{445};
t162 = ct{446};
t1620 = ct{447};
t1621 = ct{448};
t1622 = ct{449};
t1623 = ct{450};
t1625 = ct{451};
t163 = ct{452};
t1631 = ct{453};
t1632 = ct{454};
t1633 = ct{455};
t1635 = ct{456};
t1636 = ct{457};
t1637 = ct{458};
t1638 = ct{459};
t1639 = ct{460};
t1641 = ct{461};
t1643 = ct{462};
t1644 = ct{463};
t1645 = ct{464};
t165 = ct{465};
t1650 = ct{466};
t1651 = ct{467};
t1652 = ct{468};
t1653 = ct{469};
t1657 = ct{470};
t1658 = ct{471};
t1659 = ct{472};
t166 = ct{473};
t1660 = ct{474};
t1661 = ct{475};
t1662 = ct{476};
t1663 = ct{477};
t1666 = ct{478};
t1669 = ct{479};
t1672 = ct{480};
t1676 = ct{481};
t168 = ct{482};
t1681 = ct{483};
t1682 = ct{484};
t1683 = ct{485};
t1687 = ct{486};
t1689 = ct{487};
t169 = ct{488};
t1692 = ct{489};
t1695 = ct{490};
t1696 = ct{491};
t1698 = ct{492};
t17 = ct{493};
t170 = ct{494};
t1702 = ct{495};
t1703 = ct{496};
t1704 = ct{497};
t1709 = ct{498};
t171 = ct{499};
t1711 = ct{500};
t1712 = ct{501};
t1713 = ct{502};
t1716 = ct{503};
t1720 = ct{504};
t1722 = ct{505};
t1726 = ct{506};
t1728 = ct{507};
t1729 = ct{508};
t173 = ct{509};
t1731 = ct{510};
t1733 = ct{511};
t1734 = ct{512};
t1735 = ct{513};
t1736 = ct{514};
t1737 = ct{515};
t1738 = ct{516};
t1740 = ct{517};
t1744 = ct{518};
t1745 = ct{519};
t1746 = ct{520};
t1749 = ct{521};
t175 = ct{522};
t1752 = ct{523};
t1755 = ct{524};
t1756 = ct{525};
t1757 = ct{526};
t1758 = ct{527};
t1760 = ct{528};
t1761 = ct{529};
t1764 = ct{530};
t1767 = ct{531};
t1769 = ct{532};
t177 = ct{533};
t1771 = ct{534};
t1772 = ct{535};
t1774 = ct{536};
t1776 = ct{537};
t1779 = ct{538};
t1784 = ct{539};
t1785 = ct{540};
t1786 = ct{541};
t1787 = ct{542};
t1788 = ct{543};
t1789 = ct{544};
t179 = ct{545};
t1793 = ct{546};
t1795 = ct{547};
t1797 = ct{548};
t1798 = ct{549};
t1799 = ct{550};
t18 = ct{551};
t180 = ct{552};
t1800 = ct{553};
t1801 = ct{554};
t1803 = ct{555};
t1804 = ct{556};
t1807 = ct{557};
t1808 = ct{558};
t1809 = ct{559};
t181 = ct{560};
t1810 = ct{561};
t1811 = ct{562};
t1812 = ct{563};
t1814 = ct{564};
t1816 = ct{565};
t1817 = ct{566};
t182 = ct{567};
t1820 = ct{568};
t1826 = ct{569};
t1827 = ct{570};
t1829 = ct{571};
t183 = ct{572};
t1830 = ct{573};
t1831 = ct{574};
t1832 = ct{575};
t1833 = ct{576};
t1834 = ct{577};
t1835 = ct{578};
t1836 = ct{579};
t1838 = ct{580};
t1847 = ct{581};
t1849 = ct{582};
t185 = ct{583};
t1850 = ct{584};
t1851 = ct{585};
t1855 = ct{586};
t1857 = ct{587};
t1858 = ct{588};
t1859 = ct{589};
t186 = ct{590};
t1866 = ct{591};
t1867 = ct{592};
t1871 = ct{593};
t1872 = ct{594};
t1873 = ct{595};
t1881 = ct{596};
t1882 = ct{597};
t1888 = ct{598};
t1889 = ct{599};
t1896 = ct{600};
t19 = ct{601};
t190 = ct{602};
t1903 = ct{603};
t1907 = ct{604};
t1908 = ct{605};
t191 = ct{606};
t1910 = ct{607};
t1911 = ct{608};
t1912 = ct{609};
t1913 = ct{610};
t1914 = ct{611};
t1915 = ct{612};
t1916 = ct{613};
t1920 = ct{614};
t1925 = ct{615};
t1926 = ct{616};
t193 = ct{617};
t1930 = ct{618};
t1935 = ct{619};
t1936 = ct{620};
t1937 = ct{621};
t1938 = ct{622};
t1939 = ct{623};
t194 = ct{624};
t1943 = ct{625};
t1944 = ct{626};
t1946 = ct{627};
t195 = ct{628};
t1950 = ct{629};
t1955 = ct{630};
t196 = ct{631};
t1961 = ct{632};
t1964 = ct{633};
t1965 = ct{634};
t1966 = ct{635};
t1967 = ct{636};
t1968 = ct{637};
t1969 = ct{638};
t197 = ct{639};
t1970 = ct{640};
t1972 = ct{641};
t1976 = ct{642};
t1977 = ct{643};
t1978 = ct{644};
t1979 = ct{645};
t198 = ct{646};
t1981 = ct{647};
t1984 = ct{648};
t1988 = ct{649};
t1992 = ct{650};
t1994 = ct{651};
t1995 = ct{652};
t1996 = ct{653};
t1997 = ct{654};
t1998 = ct{655};
t1999 = ct{656};
t2 = ct{657};
t20 = ct{658};
t2000 = ct{659};
t2001 = ct{660};
t2002 = ct{661};
t2003 = ct{662};
t2004 = ct{663};
t2005 = ct{664};
t2006 = ct{665};
t2014 = ct{666};
t2017 = ct{667};
t2019 = ct{668};
t2020 = ct{669};
t2023 = ct{670};
t2024 = ct{671};
t2028 = ct{672};
t2029 = ct{673};
t2033 = ct{674};
t2036 = ct{675};
t2037 = ct{676};
t2038 = ct{677};
t2042 = ct{678};
t2052 = ct{679};
t2053 = ct{680};
t2056 = ct{681};
t2058 = ct{682};
t2059 = ct{683};
t206 = ct{684};
t2060 = ct{685};
t2062 = ct{686};
t2065 = ct{687};
t2066 = ct{688};
t2067 = ct{689};
t2068 = ct{690};
t2069 = ct{691};
t207 = ct{692};
t2070 = ct{693};
t2072 = ct{694};
t2073 = ct{695};
t2074 = ct{696};
t2079 = ct{697};
t2081 = ct{698};
t2082 = ct{699};
t2083 = ct{700};
t2084 = ct{701};
t2085 = ct{702};
t2086 = ct{703};
t2087 = ct{704};
t2093 = ct{705};
t2094 = ct{706};
t2096 = ct{707};
t2097 = ct{708};
t2098 = ct{709};
t21 = ct{710};
t2100 = ct{711};
t2103 = ct{712};
t2104 = ct{713};
t2105 = ct{714};
t2106 = ct{715};
t2108 = ct{716};
t2109 = ct{717};
t2110 = ct{718};
t2111 = ct{719};
t2113 = ct{720};
t2114 = ct{721};
t2115 = ct{722};
t2116 = ct{723};
t2117 = ct{724};
t2118 = ct{725};
t2121 = ct{726};
t2122 = ct{727};
t2126 = ct{728};
t2128 = ct{729};
t2129 = ct{730};
t2130 = ct{731};
t2131 = ct{732};
t2132 = ct{733};
t2133 = ct{734};
t2136 = ct{735};
t2142 = ct{736};
t2144 = ct{737};
t2148 = ct{738};
t2149 = ct{739};
t215 = ct{740};
t2154 = ct{741};
t2156 = ct{742};
t2157 = ct{743};
t2158 = ct{744};
t216 = ct{745};
t2171 = ct{746};
t2172 = ct{747};
t2175 = ct{748};
t2176 = ct{749};
t2179 = ct{750};
t2180 = ct{751};
t2182 = ct{752};
t2189 = ct{753};
t219 = ct{754};
t2194 = ct{755};
t2196 = ct{756};
t22 = ct{757};
t220 = ct{758};
t2204 = ct{759};
t2208 = ct{760};
t221 = ct{761};
t2212 = ct{762};
t2214 = ct{763};
t2217 = ct{764};
t2218 = ct{765};
t2219 = ct{766};
t222 = ct{767};
t2220 = ct{768};
t2221 = ct{769};
t2223 = ct{770};
t2225 = ct{771};
t2227 = ct{772};
t2228 = ct{773};
t2229 = ct{774};
t223 = ct{775};
t2236 = ct{776};
t2239 = ct{777};
t224 = ct{778};
t2244 = ct{779};
t225 = ct{780};
t2251 = ct{781};
t2254 = ct{782};
t2256 = ct{783};
t2257 = ct{784};
t226 = ct{785};
t2264 = ct{786};
t2265 = ct{787};
t2266 = ct{788};
t2267 = ct{789};
t2269 = ct{790};
t227 = ct{791};
t2270 = ct{792};
t2274 = ct{793};
t2276 = ct{794};
t2277 = ct{795};
t2279 = ct{796};
t228 = ct{797};
t2280 = ct{798};
t2281 = ct{799};
t2282 = ct{800};
t2285 = ct{801};
t2291 = ct{802};
t2294 = ct{803};
t23 = ct{804};
t230 = ct{805};
t2302 = ct{806};
t2304 = ct{807};
t2305 = ct{808};
t2306 = ct{809};
t231 = ct{810};
t2316 = ct{811};
t2317 = ct{812};
t2318 = ct{813};
t2321 = ct{814};
t2322 = ct{815};
t2323 = ct{816};
t2324 = ct{817};
t233 = ct{818};
t2333 = ct{819};
t2336 = ct{820};
t2339 = ct{821};
t234 = ct{822};
t2340 = ct{823};
t2344 = ct{824};
t2348 = ct{825};
t235 = ct{826};
t2350 = ct{827};
t2357 = ct{828};
t2358 = ct{829};
t2359 = ct{830};
t236 = ct{831};
t2361 = ct{832};
t2362 = ct{833};
t2363 = ct{834};
t2364 = ct{835};
t2365 = ct{836};
t2366 = ct{837};
t2369 = ct{838};
t237 = ct{839};
t2371 = ct{840};
t2372 = ct{841};
t2373 = ct{842};
t2375 = ct{843};
t2376 = ct{844};
t2377 = ct{845};
t2378 = ct{846};
t2379 = ct{847};
t238 = ct{848};
t2384 = ct{849};
t2385 = ct{850};
t2387 = ct{851};
t2388 = ct{852};
t2389 = ct{853};
t239 = ct{854};
t2391 = ct{855};
t2394 = ct{856};
t24 = ct{857};
t240 = ct{858};
t2400 = ct{859};
t2401 = ct{860};
t2402 = ct{861};
t2403 = ct{862};
t2405 = ct{863};
t2406 = ct{864};
t2407 = ct{865};
t241 = ct{866};
t2410 = ct{867};
t2417 = ct{868};
t2418 = ct{869};
t2419 = ct{870};
t242 = ct{871};
t2421 = ct{872};
t2422 = ct{873};
t2428 = ct{874};
t2429 = ct{875};
t243 = ct{876};
t2430 = ct{877};
t2431 = ct{878};
t2434 = ct{879};
t2435 = ct{880};
t2437 = ct{881};
t2438 = ct{882};
t2439 = ct{883};
t244 = ct{884};
t2440 = ct{885};
t2441 = ct{886};
t2442 = ct{887};
t2443 = ct{888};
t2444 = ct{889};
t2447 = ct{890};
t2449 = ct{891};
t245 = ct{892};
t2450 = ct{893};
t2452 = ct{894};
t2453 = ct{895};
t2454 = ct{896};
t2455 = ct{897};
t2456 = ct{898};
t2457 = ct{899};
t2458 = ct{900};
t246 = ct{901};
t2460 = ct{902};
t2466 = ct{903};
t2467 = ct{904};
t2468 = ct{905};
t247 = ct{906};
t2470 = ct{907};
t2472 = ct{908};
t2474 = ct{909};
t2477 = ct{910};
t248 = ct{911};
t2481 = ct{912};
t2483 = ct{913};
t2484 = ct{914};
t2485 = ct{915};
t2486 = ct{916};
t2487 = ct{917};
t2489 = ct{918};
t249 = ct{919};
t2492 = ct{920};
t2495 = ct{921};
t2497 = ct{922};
t2498 = ct{923};
t2499 = ct{924};
t25 = ct{925};
t2500 = ct{926};
t2501 = ct{927};
t2502 = ct{928};
t2503 = ct{929};
t2504 = ct{930};
t2505 = ct{931};
t2506 = ct{932};
t2513 = ct{933};
t2518 = ct{934};
t2521 = ct{935};
t2527 = ct{936};
t253 = ct{937};
t2533 = ct{938};
t2535 = ct{939};
t2536 = ct{940};
t2537 = ct{941};
t2538 = ct{942};
t254 = ct{943};
t2540 = ct{944};
t2543 = ct{945};
t2544 = ct{946};
t2545 = ct{947};
t2546 = ct{948};
t2549 = ct{949};
t2551 = ct{950};
t2552 = ct{951};
t2553 = ct{952};
t2554 = ct{953};
t2555 = ct{954};
t2557 = ct{955};
t2558 = ct{956};
t2559 = ct{957};
t256 = ct{958};
t2560 = ct{959};
t2561 = ct{960};
t2562 = ct{961};
t2565 = ct{962};
t257 = ct{963};
t2572 = ct{964};
t2573 = ct{965};
t2574 = ct{966};
t2575 = ct{967};
t2576 = ct{968};
t2577 = ct{969};
t2578 = ct{970};
t2579 = ct{971};
t258 = ct{972};
t2583 = ct{973};
t2584 = ct{974};
t259 = ct{975};
t2590 = ct{976};
t2591 = ct{977};
t2592 = ct{978};
t2593 = ct{979};
t2595 = ct{980};
t2596 = ct{981};
t2597 = ct{982};
t26 = ct{983};
t260 = ct{984};
t2602 = ct{985};
t2603 = ct{986};
t2604 = ct{987};
t2605 = ct{988};
t2609 = ct{989};
t261 = ct{990};
t2610 = ct{991};
t2611 = ct{992};
t2615 = ct{993};
t2617 = ct{994};
t2627 = ct{995};
t263 = ct{996};
t264 = ct{997};
t2652 = ct{998};
t2655 = ct{999};
t2656 = ct{1000};
t266 = ct{1001};
t2673 = ct{1002};
t2675 = ct{1003};
t2676 = ct{1004};
t2685 = ct{1005};
t2687 = ct{1006};
t269 = ct{1007};
t270 = ct{1008};
t2705 = ct{1009};
t2706 = ct{1010};
t2707 = ct{1011};
t2708 = ct{1012};
t2716 = ct{1013};
t2719 = ct{1014};
t272 = ct{1015};
t273 = ct{1016};
t274 = ct{1017};
t2749 = ct{1018};
t275 = ct{1019};
t2751 = ct{1020};
t2752 = ct{1021};
t276 = ct{1022};
t2764 = ct{1023};
t277 = ct{1024};
t278 = ct{1025};
t279 = ct{1026};
t280 = ct{1027};
t2804 = ct{1028};
t281 = ct{1029};
t284 = ct{1030};
t285 = ct{1031};
t2854 = ct{1032};
t286 = ct{1033};
t287 = ct{1034};
t288 = ct{1035};
t2886 = ct{1036};
t289 = ct{1037};
t29 = ct{1038};
t290 = ct{1039};
t291 = ct{1040};
t292 = ct{1041};
t293 = ct{1042};
t2939 = ct{1043};
t294 = ct{1044};
t296 = ct{1045};
t297 = ct{1046};
t299 = ct{1047};
t2997 = ct{1048};
t3 = ct{1049};
t30 = ct{1050};
t300 = ct{1051};
t302 = ct{1052};
t303 = ct{1053};
t304 = ct{1054};
t305 = ct{1055};
t3058 = ct{1056};
t306 = ct{1057};
t307 = ct{1058};
t308 = ct{1059};
t309 = ct{1060};
t31 = ct{1061};
t310 = ct{1062};
t311 = ct{1063};
t312 = ct{1064};
t313 = ct{1065};
t314 = ct{1066};
t3142 = ct{1067};
t315 = ct{1068};
t3158 = ct{1069};
t316 = ct{1070};
t318 = ct{1071};
t319 = ct{1072};
t3191 = ct{1073};
t32 = ct{1074};
t320 = ct{1075};
t3208 = ct{1076};
t321 = ct{1077};
t3211 = ct{1078};
t3212 = ct{1079};
t3218 = ct{1080};
t3219 = ct{1081};
t322 = ct{1082};
t3225 = ct{1083};
t3228 = ct{1084};
t3230 = ct{1085};
t3231 = ct{1086};
t324 = ct{1087};
t3243 = ct{1088};
t3244 = ct{1089};
t325 = ct{1090};
t3251 = ct{1091};
t3252 = ct{1092};
t3255 = ct{1093};
t3257 = ct{1094};
t3258 = ct{1095};
t3259 = ct{1096};
t3261 = ct{1097};
t3273 = ct{1098};
t3274 = ct{1099};
t3275 = ct{1100};
t3279 = ct{1101};
t328 = ct{1102};
t3282 = ct{1103};
t3286 = ct{1104};
t3288 = ct{1105};
t3289 = ct{1106};
t329 = ct{1107};
t3290 = ct{1108};
t3294 = ct{1109};
t3295 = ct{1110};
t33 = ct{1111};
t3309 = ct{1112};
t3314 = ct{1113};
t3317 = ct{1114};
t3319 = ct{1115};
t332 = ct{1116};
t3320 = ct{1117};
t3321 = ct{1118};
t3326 = ct{1119};
t3327 = ct{1120};
t3328 = ct{1121};
t3329 = ct{1122};
t333 = ct{1123};
t3330 = ct{1124};
t3331 = ct{1125};
t3333 = ct{1126};
t3334 = ct{1127};
t3335 = ct{1128};
t334 = ct{1129};
t3343 = ct{1130};
t336 = ct{1131};
t3363 = ct{1132};
t3364 = ct{1133};
t3365 = ct{1134};
t3367 = ct{1135};
t3368 = ct{1136};
t3369 = ct{1137};
t337 = ct{1138};
t3370 = ct{1139};
t3371 = ct{1140};
t3372 = ct{1141};
t3373 = ct{1142};
t3374 = ct{1143};
t3375 = ct{1144};
t3376 = ct{1145};
t3378 = ct{1146};
t3379 = ct{1147};
t3380 = ct{1148};
t3381 = ct{1149};
t3382 = ct{1150};
t3389 = ct{1151};
t3390 = ct{1152};
t3391 = ct{1153};
t3392 = ct{1154};
t3393 = ct{1155};
t3394 = ct{1156};
t3395 = ct{1157};
t3397 = ct{1158};
t34 = ct{1159};
t340 = ct{1160};
t3400 = ct{1161};
t3401 = ct{1162};
t3402 = ct{1163};
t3403 = ct{1164};
t3409 = ct{1165};
t341 = ct{1166};
t3416 = ct{1167};
t3417 = ct{1168};
t3418 = ct{1169};
t3419 = ct{1170};
t3420 = ct{1171};
t3426 = ct{1172};
t3430 = ct{1173};
t3432 = ct{1174};
t3434 = ct{1175};
t3435 = ct{1176};
t3437 = ct{1177};
t3438 = ct{1178};
t3439 = ct{1179};
t344 = ct{1180};
t3440 = ct{1181};
t3442 = ct{1182};
t3443 = ct{1183};
t3444 = ct{1184};
t3445 = ct{1185};
t3446 = ct{1186};
t3447 = ct{1187};
t3449 = ct{1188};
t345 = ct{1189};
t3450 = ct{1190};
t3452 = ct{1191};
t3453 = ct{1192};
t3454 = ct{1193};
t3455 = ct{1194};
t3456 = ct{1195};
t3459 = ct{1196};
t346 = ct{1197};
t3462 = ct{1198};
t3463 = ct{1199};
t3466 = ct{1200};
t3468 = ct{1201};
t3469 = ct{1202};
t347 = ct{1203};
t3470 = ct{1204};
t3472 = ct{1205};
t3473 = ct{1206};
t3475 = ct{1207};
t3477 = ct{1208};
t3479 = ct{1209};
t348 = ct{1210};
t3481 = ct{1211};
t3483 = ct{1212};
t3486 = ct{1213};
t3489 = ct{1214};
t349 = ct{1215};
t3492 = ct{1216};
t350 = ct{1217};
t3500 = ct{1218};
t3501 = ct{1219};
t3506 = ct{1220};
t3507 = ct{1221};
t3509 = ct{1222};
t3514 = ct{1223};
t3515 = ct{1224};
t3516 = ct{1225};
t3517 = ct{1226};
t3519 = ct{1227};
t352 = ct{1228};
t3520 = ct{1229};
t3521 = ct{1230};
t3522 = ct{1231};
t3523 = ct{1232};
t3524 = ct{1233};
t353 = ct{1234};
t3530 = ct{1235};
t3532 = ct{1236};
t3533 = ct{1237};
t3534 = ct{1238};
t3535 = ct{1239};
t3538 = ct{1240};
t3539 = ct{1241};
t354 = ct{1242};
t3541 = ct{1243};
t3544 = ct{1244};
t3546 = ct{1245};
t3548 = ct{1246};
t3549 = ct{1247};
t355 = ct{1248};
t3553 = ct{1249};
t3556 = ct{1250};
t356 = ct{1251};
t3560 = ct{1252};
t3568 = ct{1253};
t3569 = ct{1254};
t357 = ct{1255};
t3572 = ct{1256};
t3573 = ct{1257};
t3574 = ct{1258};
t3575 = ct{1259};
t3576 = ct{1260};
t3578 = ct{1261};
t3579 = ct{1262};
t358 = ct{1263};
t3581 = ct{1264};
t3582 = ct{1265};
t3583 = ct{1266};
t3584 = ct{1267};
t3585 = ct{1268};
t359 = ct{1269};
t3590 = ct{1270};
t3596 = ct{1271};
t3597 = ct{1272};
t360 = ct{1273};
t3601 = ct{1274};
t3602 = ct{1275};
t3604 = ct{1276};
t3607 = ct{1277};
t3609 = ct{1278};
t361 = ct{1279};
t3613 = ct{1280};
t3616 = ct{1281};
t3617 = ct{1282};
t3618 = ct{1283};
t362 = ct{1284};
t3622 = ct{1285};
t3629 = ct{1286};
t3630 = ct{1287};
t3637 = ct{1288};
t3638 = ct{1289};
t3639 = ct{1290};
t3641 = ct{1291};
t3643 = ct{1292};
t3646 = ct{1293};
t3647 = ct{1294};
t3649 = ct{1295};
t365 = ct{1296};
t3650 = ct{1297};
t3652 = ct{1298};
t3653 = ct{1299};
t3654 = ct{1300};
t3659 = ct{1301};
t366 = ct{1302};
t3660 = ct{1303};
t3662 = ct{1304};
t3663 = ct{1305};
t3668 = ct{1306};
t367 = ct{1307};
t3676 = ct{1308};
t368 = ct{1309};
t3680 = ct{1310};
t3682 = ct{1311};
t3686 = ct{1312};
t369 = ct{1313};
t3691 = ct{1314};
t3695 = ct{1315};
t3697 = ct{1316};
t3701 = ct{1317};
t3709 = ct{1318};
t371 = ct{1319};
t3714 = ct{1320};
t3716 = ct{1321};
t3717 = ct{1322};
t372 = ct{1323};
t3722 = ct{1324};
t3726 = ct{1325};
t3729 = ct{1326};
t373 = ct{1327};
t3730 = ct{1328};
t3736 = ct{1329};
t3737 = ct{1330};
t3738 = ct{1331};
t374 = ct{1332};
t3743 = ct{1333};
t3744 = ct{1334};
t3747 = ct{1335};
t3748 = ct{1336};
t375 = ct{1337};
t3750 = ct{1338};
t3751 = ct{1339};
t3756 = ct{1340};
t376 = ct{1341};
t377 = ct{1342};
t3774 = ct{1343};
t378 = ct{1344};
t3789 = ct{1345};
t379 = ct{1346};
t3798 = ct{1347};
t380 = ct{1348};
t3815 = ct{1349};
t382 = ct{1350};
t3822 = ct{1351};
t3824 = ct{1352};
t3825 = ct{1353};
t3834 = ct{1354};
t3835 = ct{1355};
t3839 = ct{1356};
t384 = ct{1357};
t3846 = ct{1358};
t3847 = ct{1359};
t3852 = ct{1360};
t386 = ct{1361};
t387 = ct{1362};
t388 = ct{1363};
t3889 = ct{1364};
t389 = ct{1365};
t3892 = ct{1366};
t3898 = ct{1367};
t3899 = ct{1368};
t391 = ct{1369};
t3915 = ct{1370};
t392 = ct{1371};
t395 = ct{1372};
t3950 = ct{1373};
t3951 = ct{1374};
t3958 = ct{1375};
t3959 = ct{1376};
t396 = ct{1377};
t398 = ct{1378};
t4 = ct{1379};
t400 = ct{1380};
t4001 = ct{1381};
t4002 = ct{1382};
t4004 = ct{1383};
t4007 = ct{1384};
t401 = ct{1385};
t402 = ct{1386};
t4028 = ct{1387};
t4029 = ct{1388};
t403 = ct{1389};
t4030 = ct{1390};
t4031 = ct{1391};
t4032 = ct{1392};
t4033 = ct{1393};
t4039 = ct{1394};
t404 = ct{1395};
t4040 = ct{1396};
t4041 = ct{1397};
t4042 = ct{1398};
t4043 = ct{1399};
t4044 = ct{1400};
t4045 = ct{1401};
t4051 = ct{1402};
t4052 = ct{1403};
t4058 = ct{1404};
t406 = ct{1405};
t409 = ct{1406};
t410 = ct{1407};
t4105 = ct{1408};
t411 = ct{1409};
t4113 = ct{1410};
t4114 = ct{1411};
t4117 = ct{1412};
t4118 = ct{1413};
t412 = ct{1414};
t4123 = ct{1415};
t413 = ct{1416};
t414 = ct{1417};
t4143 = ct{1418};
t4144 = ct{1419};
t4145 = ct{1420};
t415 = ct{1421};
t4150 = ct{1422};
t4152 = ct{1423};
t4153 = ct{1424};
t4155 = ct{1425};
t416 = ct{1426};
t4160 = ct{1427};
t4164 = ct{1428};
t4165 = ct{1429};
t417 = ct{1430};
t4170 = ct{1431};
t4174 = ct{1432};
t4177 = ct{1433};
t4178 = ct{1434};
t4179 = ct{1435};
t418 = ct{1436};
t4180 = ct{1437};
t4181 = ct{1438};
t4182 = ct{1439};
t4183 = ct{1440};
t4184 = ct{1441};
t4185 = ct{1442};
t4186 = ct{1443};
t4187 = ct{1444};
t4188 = ct{1445};
t4189 = ct{1446};
t419 = ct{1447};
t4190 = ct{1448};
t4191 = ct{1449};
t4192 = ct{1450};
t4193 = ct{1451};
t4194 = ct{1452};
t4196 = ct{1453};
t4197 = ct{1454};
t420 = ct{1455};
t4200 = ct{1456};
t4203 = ct{1457};
t4204 = ct{1458};
t4205 = ct{1459};
t4206 = ct{1460};
t4207 = ct{1461};
t4208 = ct{1462};
t4209 = ct{1463};
t421 = ct{1464};
t4211 = ct{1465};
t4212 = ct{1466};
t4213 = ct{1467};
t4214 = ct{1468};
t4216 = ct{1469};
t422 = ct{1470};
t4221 = ct{1471};
t4228 = ct{1472};
t4229 = ct{1473};
t423 = ct{1474};
t4230 = ct{1475};
t4231 = ct{1476};
t4232 = ct{1477};
t4233 = ct{1478};
t4235 = ct{1479};
t4236 = ct{1480};
t4237 = ct{1481};
t4239 = ct{1482};
t424 = ct{1483};
t4240 = ct{1484};
t4242 = ct{1485};
t4243 = ct{1486};
t4246 = ct{1487};
t4249 = ct{1488};
t425 = ct{1489};
t4255 = ct{1490};
t4256 = ct{1491};
t4257 = ct{1492};
t4258 = ct{1493};
t4259 = ct{1494};
t426 = ct{1495};
t4260 = ct{1496};
t4261 = ct{1497};
t4262 = ct{1498};
t4265 = ct{1499};
t4266 = ct{1500};
t4268 = ct{1501};
t427 = ct{1502};
t4271 = ct{1503};
t4272 = ct{1504};
t4275 = ct{1505};
t4277 = ct{1506};
t4278 = ct{1507};
t4279 = ct{1508};
t428 = ct{1509};
t4283 = ct{1510};
t4284 = ct{1511};
t4287 = ct{1512};
t4288 = ct{1513};
t4289 = ct{1514};
t429 = ct{1515};
t4290 = ct{1516};
t4292 = ct{1517};
t4293 = ct{1518};
t4294 = ct{1519};
t4295 = ct{1520};
t4296 = ct{1521};
t4297 = ct{1522};
t4298 = ct{1523};
t4299 = ct{1524};
t4300 = ct{1525};
t4301 = ct{1526};
t4304 = ct{1527};
t4308 = ct{1528};
t4309 = ct{1529};
t431 = ct{1530};
t4310 = ct{1531};
t4311 = ct{1532};
t4313 = ct{1533};
t4315 = ct{1534};
t4316 = ct{1535};
t4317 = ct{1536};
t4319 = ct{1537};
t432 = ct{1538};
t4320 = ct{1539};
t4321 = ct{1540};
t4323 = ct{1541};
t4325 = ct{1542};
t4326 = ct{1543};
t4328 = ct{1544};
t433 = ct{1545};
t4330 = ct{1546};
t4333 = ct{1547};
t4334 = ct{1548};
t4335 = ct{1549};
t4336 = ct{1550};
t4337 = ct{1551};
t4338 = ct{1552};
t4339 = ct{1553};
t434 = ct{1554};
t4341 = ct{1555};
t4342 = ct{1556};
t4343 = ct{1557};
t4344 = ct{1558};
t4345 = ct{1559};
t4346 = ct{1560};
t4347 = ct{1561};
t435 = ct{1562};
t4351 = ct{1563};
t4353 = ct{1564};
t4355 = ct{1565};
t436 = ct{1566};
t4361 = ct{1567};
t4365 = ct{1568};
t4367 = ct{1569};
t4369 = ct{1570};
t437 = ct{1571};
t4370 = ct{1572};
t4371 = ct{1573};
t4372 = ct{1574};
t4375 = ct{1575};
t4377 = ct{1576};
t4379 = ct{1577};
t438 = ct{1578};
t4382 = ct{1579};
t4385 = ct{1580};
t4387 = ct{1581};
t439 = ct{1582};
t4390 = ct{1583};
t4391 = ct{1584};
t4392 = ct{1585};
t4394 = ct{1586};
t4395 = ct{1587};
t4396 = ct{1588};
t4397 = ct{1589};
t44 = ct{1590};
t440 = ct{1591};
t4401 = ct{1592};
t4402 = ct{1593};
t4403 = ct{1594};
t4404 = ct{1595};
t4405 = ct{1596};
t4406 = ct{1597};
t4407 = ct{1598};
t4408 = ct{1599};
t441 = ct{1600};
t4410 = ct{1601};
t4411 = ct{1602};
t4412 = ct{1603};
t4413 = ct{1604};
t4417 = ct{1605};
t4419 = ct{1606};
t442 = ct{1607};
t4420 = ct{1608};
t4421 = ct{1609};
t4422 = ct{1610};
t4425 = ct{1611};
t4426 = ct{1612};
t4428 = ct{1613};
t4429 = ct{1614};
t443 = ct{1615};
t4431 = ct{1616};
t4432 = ct{1617};
t4435 = ct{1618};
t4436 = ct{1619};
t444 = ct{1620};
t4440 = ct{1621};
t4442 = ct{1622};
t4443 = ct{1623};
t4444 = ct{1624};
t4445 = ct{1625};
t4446 = ct{1626};
t4448 = ct{1627};
t4449 = ct{1628};
t445 = ct{1629};
t4450 = ct{1630};
t4452 = ct{1631};
t4453 = ct{1632};
t4455 = ct{1633};
t4457 = ct{1634};
t4459 = ct{1635};
t4462 = ct{1636};
t4464 = ct{1637};
t4469 = ct{1638};
t4473 = ct{1639};
t4478 = ct{1640};
t4479 = ct{1641};
t448 = ct{1642};
t4480 = ct{1643};
t4481 = ct{1644};
t4483 = ct{1645};
t4484 = ct{1646};
t4485 = ct{1647};
t4486 = ct{1648};
t4488 = ct{1649};
t449 = ct{1650};
t4491 = ct{1651};
t4492 = ct{1652};
t4493 = ct{1653};
t4495 = ct{1654};
t4498 = ct{1655};
t45 = ct{1656};
t450 = ct{1657};
t4501 = ct{1658};
t4502 = ct{1659};
t4504 = ct{1660};
t4506 = ct{1661};
t4508 = ct{1662};
t4509 = ct{1663};
t4513 = ct{1664};
t4516 = ct{1665};
t4517 = ct{1666};
t4519 = ct{1667};
t452 = ct{1668};
t4520 = ct{1669};
t4522 = ct{1670};
t4524 = ct{1671};
t4525 = ct{1672};
t453 = ct{1673};
t4530 = ct{1674};
t4532 = ct{1675};
t4533 = ct{1676};
t454 = ct{1677};
t4540 = ct{1678};
t4542 = ct{1679};
t4543 = ct{1680};
t4547 = ct{1681};
t4548 = ct{1682};
t4549 = ct{1683};
t4551 = ct{1684};
t4554 = ct{1685};
t4555 = ct{1686};
t4557 = ct{1687};
t4558 = ct{1688};
t4559 = ct{1689};
t4561 = ct{1690};
t4562 = ct{1691};
t4563 = ct{1692};
t4566 = ct{1693};
t4567 = ct{1694};
t4568 = ct{1695};
t4569 = ct{1696};
t457 = ct{1697};
t4570 = ct{1698};
t4571 = ct{1699};
t4572 = ct{1700};
t4574 = ct{1701};
t4575 = ct{1702};
t4577 = ct{1703};
t4579 = ct{1704};
t458 = ct{1705};
t4581 = ct{1706};
t4582 = ct{1707};
t4583 = ct{1708};
t4584 = ct{1709};
t4588 = ct{1710};
t4589 = ct{1711};
t459 = ct{1712};
t4590 = ct{1713};
t4591 = ct{1714};
t4595 = ct{1715};
t4596 = ct{1716};
t46 = ct{1717};
t460 = ct{1718};
t4600 = ct{1719};
t4601 = ct{1720};
t4605 = ct{1721};
t4606 = ct{1722};
t4607 = ct{1723};
t461 = ct{1724};
t4611 = ct{1725};
t4614 = ct{1726};
t4616 = ct{1727};
t4617 = ct{1728};
t462 = ct{1729};
t4621 = ct{1730};
t4622 = ct{1731};
t4625 = ct{1732};
t4626 = ct{1733};
t4628 = ct{1734};
t4629 = ct{1735};
t463 = ct{1736};
t4630 = ct{1737};
t4632 = ct{1738};
t4633 = ct{1739};
t4634 = ct{1740};
t4636 = ct{1741};
t4637 = ct{1742};
t4638 = ct{1743};
t4639 = ct{1744};
t464 = ct{1745};
t4640 = ct{1746};
t4641 = ct{1747};
t4642 = ct{1748};
t4643 = ct{1749};
t4644 = ct{1750};
t4645 = ct{1751};
t4646 = ct{1752};
t4647 = ct{1753};
t4649 = ct{1754};
t465 = ct{1755};
t4650 = ct{1756};
t4651 = ct{1757};
t4652 = ct{1758};
t4653 = ct{1759};
t4656 = ct{1760};
t4657 = ct{1761};
t4658 = ct{1762};
t466 = ct{1763};
t4660 = ct{1764};
t4661 = ct{1765};
t4662 = ct{1766};
t4663 = ct{1767};
t4666 = ct{1768};
t4667 = ct{1769};
t4669 = ct{1770};
t4672 = ct{1771};
t4673 = ct{1772};
t4674 = ct{1773};
t4675 = ct{1774};
t468 = ct{1775};
t4688 = ct{1776};
t469 = ct{1777};
t4691 = ct{1778};
t4692 = ct{1779};
t4693 = ct{1780};
t4694 = ct{1781};
t47 = ct{1782};
t470 = ct{1783};
t471 = ct{1784};
t472 = ct{1785};
t475 = ct{1786};
t4763 = ct{1787};
t477 = ct{1788};
t479 = ct{1789};
t480 = ct{1790};
t481 = ct{1791};
t482 = ct{1792};
t483 = ct{1793};
t484 = ct{1794};
t485 = ct{1795};
t486 = ct{1796};
t488 = ct{1797};
t489 = ct{1798};
t491 = ct{1799};
t492 = ct{1800};
t493 = ct{1801};
t494 = ct{1802};
t496 = ct{1803};
t497 = ct{1804};
t498 = ct{1805};
t499 = ct{1806};
t5 = ct{1807};
t50 = ct{1808};
t500 = ct{1809};
t501 = ct{1810};
t502 = ct{1811};
t503 = ct{1812};
t504 = ct{1813};
t505 = ct{1814};
t506 = ct{1815};
t507 = ct{1816};
t508 = ct{1817};
t509 = ct{1818};
t510 = ct{1819};
t511 = ct{1820};
t512 = ct{1821};
t513 = ct{1822};
t514 = ct{1823};
t516 = ct{1824};
t517 = ct{1825};
t518 = ct{1826};
t520 = ct{1827};
t521 = ct{1828};
t522 = ct{1829};
t523 = ct{1830};
t524 = ct{1831};
t525 = ct{1832};
t526 = ct{1833};
t527 = ct{1834};
t528 = ct{1835};
t529 = ct{1836};
t53 = ct{1837};
t530 = ct{1838};
t531 = ct{1839};
t532 = ct{1840};
t533 = ct{1841};
t534 = ct{1842};
t535 = ct{1843};
t536 = ct{1844};
t5361 = ct{1845};
t537 = ct{1846};
t538 = ct{1847};
t539 = ct{1848};
t540 = ct{1849};
t543 = ct{1850};
t544 = ct{1851};
t545 = ct{1852};
t546 = ct{1853};
t547 = ct{1854};
t548 = ct{1855};
t549 = ct{1856};
t551 = ct{1857};
t552 = ct{1858};
t553 = ct{1859};
t554 = ct{1860};
t555 = ct{1861};
t556 = ct{1862};
t557 = ct{1863};
t558 = ct{1864};
t559 = ct{1865};
t560 = ct{1866};
t561 = ct{1867};
t562 = ct{1868};
t563 = ct{1869};
t564 = ct{1870};
t567 = ct{1871};
t568 = ct{1872};
t569 = ct{1873};
t57 = ct{1874};
t570 = ct{1875};
t571 = ct{1876};
t572 = ct{1877};
t573 = ct{1878};
t574 = ct{1879};
t576 = ct{1880};
t577 = ct{1881};
t5777 = ct{1882};
t578 = ct{1883};
t579 = ct{1884};
t58 = ct{1885};
t580 = ct{1886};
t581 = ct{1887};
t582 = ct{1888};
t583 = ct{1889};
t584 = ct{1890};
t586 = ct{1891};
t587 = ct{1892};
t589 = ct{1893};
t59 = ct{1894};
t590 = ct{1895};
t591 = ct{1896};
t592 = ct{1897};
t593 = ct{1898};
t594 = ct{1899};
t595 = ct{1900};
t596 = ct{1901};
t597 = ct{1902};
t6 = ct{1903};
t60 = ct{1904};
t600 = ct{1905};
t602 = ct{1906};
t603 = ct{1907};
t604 = ct{1908};
t605 = ct{1909};
t609 = ct{1910};
t610 = ct{1911};
t611 = ct{1912};
t612 = ct{1913};
t613 = ct{1914};
t614 = ct{1915};
t615 = ct{1916};
t617 = ct{1917};
t618 = ct{1918};
t623 = ct{1919};
t625 = ct{1920};
t626 = ct{1921};
t629 = ct{1922};
t63 = ct{1923};
t633 = ct{1924};
t634 = ct{1925};
t638 = ct{1926};
t640 = ct{1927};
t643 = ct{1928};
t644 = ct{1929};
t655 = ct{1930};
t656 = ct{1931};
t660 = ct{1932};
t662 = ct{1933};
t663 = ct{1934};
t664 = ct{1935};
t665 = ct{1936};
t667 = ct{1937};
t668 = ct{1938};
t673 = ct{1939};
t674 = ct{1940};
t675 = ct{1941};
t676 = ct{1942};
t681 = ct{1943};
t682 = ct{1944};
t683 = ct{1945};
t685 = ct{1946};
t686 = ct{1947};
t687 = ct{1948};
t688 = ct{1949};
t689 = ct{1950};
t693 = ct{1951};
t694 = ct{1952};
t695 = ct{1953};
t696 = ct{1954};
t697 = ct{1955};
t698 = ct{1956};
t7 = ct{1957};
t700 = ct{1958};
t702 = ct{1959};
t703 = ct{1960};
t704 = ct{1961};
t705 = ct{1962};
t706 = ct{1963};
t71 = ct{1964};
t711 = ct{1965};
t713 = ct{1966};
t715 = ct{1967};
t716 = ct{1968};
t72 = ct{1969};
t724 = ct{1970};
t725 = ct{1971};
t727 = ct{1972};
t728 = ct{1973};
t73 = ct{1974};
t731 = ct{1975};
t733 = ct{1976};
t734 = ct{1977};
t735 = ct{1978};
t736 = ct{1979};
t74 = ct{1980};
t744 = ct{1981};
t746 = ct{1982};
t747 = ct{1983};
t748 = ct{1984};
t749 = ct{1985};
t75 = ct{1986};
t750 = ct{1987};
t751 = ct{1988};
t752 = ct{1989};
t755 = ct{1990};
t756 = ct{1991};
t757 = ct{1992};
t758 = ct{1993};
t759 = ct{1994};
t76 = ct{1995};
t762 = ct{1996};
t763 = ct{1997};
t764 = ct{1998};
t765 = ct{1999};
t766 = ct{2000};
t768 = ct{2001};
t769 = ct{2002};
t77 = ct{2003};
t772 = ct{2004};
t774 = ct{2005};
t775 = ct{2006};
t776 = ct{2007};
t780 = ct{2008};
t782 = ct{2009};
t785 = ct{2010};
t786 = ct{2011};
t788 = ct{2012};
t791 = ct{2013};
t793 = ct{2014};
t795 = ct{2015};
t8 = ct{2016};
t80 = ct{2017};
t804 = ct{2018};
t805 = ct{2019};
t806 = ct{2020};
t808 = ct{2021};
t81 = ct{2022};
t814 = ct{2023};
t815 = ct{2024};
t816 = ct{2025};
t818 = ct{2026};
t819 = ct{2027};
t82 = ct{2028};
t820 = ct{2029};
t821 = ct{2030};
t822 = ct{2031};
t825 = ct{2032};
t827 = ct{2033};
t83 = ct{2034};
t833 = ct{2035};
t834 = ct{2036};
t835 = ct{2037};
t836 = ct{2038};
t837 = ct{2039};
t838 = ct{2040};
t84 = ct{2041};
t840 = ct{2042};
t841 = ct{2043};
t842 = ct{2044};
t843 = ct{2045};
t846 = ct{2046};
t851 = ct{2047};
t855 = ct{2048};
t857 = ct{2049};
t86 = ct{2050};
t862 = ct{2051};
t864 = ct{2052};
t874 = ct{2053};
t880 = ct{2054};
t882 = ct{2055};
t884 = ct{2056};
t885 = ct{2057};
t888 = ct{2058};
t891 = ct{2059};
t892 = ct{2060};
t895 = ct{2061};
t897 = ct{2062};
t899 = ct{2063};
t9 = ct{2064};
t90 = ct{2065};
t900 = ct{2066};
t903 = ct{2067};
t904 = ct{2068};
t906 = ct{2069};
t91 = ct{2070};
t911 = ct{2071};
t921 = ct{2072};
t922 = ct{2073};
t923 = ct{2074};
t926 = ct{2075};
t927 = ct{2076};
t934 = ct{2077};
t935 = ct{2078};
t936 = ct{2079};
t937 = ct{2080};
t940 = ct{2081};
t941 = ct{2082};
t942 = ct{2083};
t946 = ct{2084};
t949 = ct{2085};
t95 = ct{2086};
t950 = ct{2087};
t956 = ct{2088};
t957 = ct{2089};
t958 = ct{2090};
t961 = ct{2091};
t962 = ct{2092};
t964 = ct{2093};
t965 = ct{2094};
t966 = ct{2095};
t968 = ct{2096};
t969 = ct{2097};
t97 = ct{2098};
t970 = ct{2099};
t971 = ct{2100};
t972 = ct{2101};
t977 = ct{2102};
t979 = ct{2103};
t982 = ct{2104};
t983 = ct{2105};
t984 = ct{2106};
t986 = ct{2107};
t987 = ct{2108};
t988 = ct{2109};
t989 = ct{2110};
t99 = ct{2111};
t993 = ct{2112};
t994 = ct{2113};
t995 = ct{2114};
t997 = ct{2115};
t999 = ct{2116};
t4695 = t7.*t23.*t34.*t191.*1.565126759819563e-23;
t4696 = t3.*t5.*t8.*t34.*t191.*1.094169869929701e-29;
t4697 = t9.*t17.*t18.*t34.*t191.*1.534519861952243e-29;
t4707 = t3.*t7.*t18.*t34.*t191.*2.878479070948652e-23;
t4708 = t4.*t8.*t17.*t34.*t191.*2.878479070948652e-23;
t4709 = t2.*t3.*t8.*t9.*t34.*t191.*(-4.035603346078089e-29);
t4711 = t2.*t7.*t8.*t9.*t34.*t191.*(-4.035603346078089e-29);
t4713 = t2.*t3.*t5.*t8.*t34.*t191.*1.664699206432988e-28;
t4716 = t2.*t3.*t8.*t9.*t34.*t191.*1.664699206432988e-28;
t4722 = t3.*t5.*t8.*t34.*t191.*(-1.378424649377201e-28);
t4723 = t6.*t7.*t8.*t9.*t34.*t191.*(-1.664699206432988e-28);
t4724 = t3.*t7.*t8.*t9.*t34.*t191.*2.012325871304092e-29;
t4725 = t3.*t8.*t9.*t34.*t191.*(-1.378424649377201e-28);
t4726 = t7.*t8.*t9.*t34.*t191.*(-1.378424649377201e-28);
t4727 = t7.*t9.*t18.*t34.*t191.*2.188339739859402e-29;
t4728 = t4.*t9.*t17.*t34.*t191.*2.012325871304092e-29;
t4731 = t4.*t9.*t22.*t34.*t191.*2.012325871304092e-29;
t4732 = t4.*t5.*t7.*t8.*t34.*t191.*4.376679479718804e-29;
t4733 = t3.*t4.*t5.*t7.*t34.*t191.*2.012325871304092e-29;
t4734 = t3.*t6.*t8.*t9.*t34.*t191.*(-1.664699206432988e-28);
t4737 = t3.*t4.*t5.*t7.*t8.*t34.*t191.*4.024651742608185e-29;
t4740 = t3.*t8.*t34.*t191.*4.600256857167288e-23;
t4741 = t4.*t7.*t34.*t191.*4.600256857167288e-23;
t4742 = t80+t118+t135+t155+t168;
t4745 = t5.*t17.*t18.*t34.*t191.*2.012325871304092e-29;
t4747 = t5.*t17.*t23.*t34.*t191.*2.012325871304092e-29;
t4748 = t4.*t8.*t9.*t17.*t34.*t191.*(-2.012325871304092e-29);
t4749 = t2.*t3.*t4.*t34.*t191.*3.903039427556764e-22;
t4752 = t2.*t7.*t8.*t34.*t191.*3.903039427556764e-22;
t4753 = t3.*t6.*t8.*t34.*t191.*3.903039427556764e-22;
t4754 = t4.*t6.*t7.*t34.*t191.*3.903039427556764e-22;
t4755 = t18.*t34.*t191.*7.111823653759751e-23;
t4756 = t23.*t34.*t191.*7.111823653759751e-23;
t4758 = t2.*t3.*t8.*t34.*t191.*1.610016168721029e-21;
t4759 = t2.*t4.*t7.*t34.*t191.*1.610016168721029e-21;
t4760 = t3.*t4.*t6.*t34.*t191.*1.610016168721029e-21;
t4761 = t6.*t7.*t8.*t34.*t191.*1.610016168721029e-21;
t4766 = t3.*t4.*t34.*t191.*1.333145329970004e-21;
t4769 = t7.*t8.*t34.*t191.*1.333145329970004e-21;
t4770 = t3.*t18.*t34.*t191.*4.228198149851719e-23;
t4777 = t7.*t8.*t34.*t191.*6.665726649850018e-22;
t4778 = t3.*t18.*t34.*t191.*4.22819770354027e-23;
t4782 = t4.*t7.*t8.*t34.*t191.*7.733879758902498e-23;
t4783 = t3.*t4.*t7.*t8.*t34.*t191.*7.111823653759751e-23;
t4785 = t17.*t18.*t34.*t191.*3.555911826879876e-23;
t4786 = t17.*t23.*t34.*t191.*3.555911826879876e-23;
t4788 = t4.*t9.*t34.*t190.*t191.*4.549258542705501e-23;
t4789 = t5.*t8.*t34.*t190.*t191.*4.549258542705501e-23;
t4790 = t8.*t34.*t190.*t191.*9.978586703210931e-25;
t4794 = t4.*t19.*t34.*t190.*t191.*1.414846738462756e-22;
t4795 = t8.*t19.*t34.*t190.*t191.*9.299848787979342e-23;
t4796 = t8.*t24.*t34.*t190.*t191.*9.299848787979342e-23;
t4797 = t3.*t9.*t34.*t191.*2.31597234870096e-23;
t4798 = t5.*t17.*t34.*t190.*t191.*9.098517085411002e-23;
t4799 = t5.*t22.*t34.*t190.*t191.*9.098517085411002e-23;
t4800 = t4.*t5.*t9.*t34.*t190.*t191.*9.299848787979342e-23;
t4801 = t5.*t8.*t9.*t34.*t190.*t191.*2.829693476925513e-22;
t4803 = t2.*t3.*t5.*t34.*t191.*1.964962320751208e-22;
t4804 = t2.*t4.*t7.*t34.*t191.*1.964962320751208e-22;
t4805 = t4.*t5.*t34.*t191.*3.895462404363107e-23;
t4807 = t2.*t7.*t9.*t34.*t191.*1.964962320751208e-22;
t4808 = t3.*t6.*t9.*t34.*t191.*1.964962320751208e-22;
t4811 = t2.*t8.*t34.*t191.*3.305064005090484e-22;
t4813 = t4.*t5.*t34.*t190.*t191.*2.472625392454631e-23;
t4814 = t8.*t9.*t34.*t190.*t191.*2.472625392454631e-23;
t4815 = t3.*t5.*t34.*t191.*1.258783598220194e-23;
t4818 = t7.*t34.*t191.*3.241975520997159e-26;
t4820 = t5.*t9.*t22.*t34.*t190.*t191.*2.829693476925513e-22;
t4824 = t2.*t3.*t5.*t34.*t191.*9.824811603756039e-23;
t4825 = t6.*t8.*t34.*t191.*1.363349406435421e-21;
t4827 = t4.*t34.*t190.*t191.*7.059909452387201e-23;
t4828 = t9.*t17.*t34.*t190.*t191.*4.945250784909262e-23;
t4830 = t2.*t7.*t9.*t34.*t191.*9.824811603756039e-23;
t4832 = t3.*t6.*t9.*t34.*t191.*9.824811603756039e-23;
t4833 = t9.*t22.*t34.*t190.*t191.*4.945250784909262e-23;
t4834 = t5.*t7.*t8.*t34.*t191.*2.31597234870096e-23;
t4835 = t4.*t9.*t17.*t34.*t190.*t191.*9.098517085411002e-23;
t4837 = t8.*t34.*t191.*4.105845905084658e-20;
t4839 = t17.*t19.*t34.*t190.*t191.*1.859969757595868e-22;
t4841 = t19.*t22.*t34.*t190.*t191.*1.859969757595868e-22;
t4842 = t3.*t5.*t34.*t191.*2.114674168334142e-23;
t4845 = t8.*t17.*t34.*t190.*t191.*1.995717340642186e-24;
t4846 = t8.*t34.*t191.*7.550142865910989e-22;
t4849 = t7.*t34.*t191.*2.623052646664375e-22;
t4852 = t5.*t9.*t17.*t34.*t190.*t191.*2.829693476925513e-22;
t4861 = t5.*t6.*t7.*t8.*t34.*t191.*1.964962320751208e-22;
t4862 = t2.*t8.*t34.*t191.*1.79637738896555e-22;
t4864 = t2.*t3.*t9.*t34.*t191.*4.052766012304177e-22;
t4865 = t2.*t3.*t9.*t34.*t191.*8.105532024608353e-22;
t4866 = t3.*t5.*t6.*t34.*t191.*4.052766012304177e-22;
t4867 = t3.*t5.*t6.*t34.*t191.*8.105532024608353e-22;
t4871 = t4.*t6.*t7.*t34.*t191.*8.105532024608353e-22;
t4872 = t4.*t9.*t34.*t190.*t191.*1.785238843466173e-29;
t4873 = t5.*t8.*t34.*t190.*t191.*1.785238843466173e-29;
t4876 = t5.*t8.*t17.*t34.*t190.*t191.*(-9.098517085411002e-23);
t4877 = t8.*t34.*t191.*3.49465336532355e-22;
t4878 = t6.*t7.*t9.*t34.*t191.*4.052766012304177e-22;
t4879 = t6.*t7.*t9.*t34.*t191.*8.105532024608353e-22;
t4882 = t2.*t4.*t9.*t34.*t191.*1.652532002545242e-22;
t4883 = t2.*t4.*t9.*t34.*t191.*3.305064005090484e-22;
t4884 = t2.*t5.*t8.*t34.*t191.*1.652532002545242e-22;
t4886 = t4.*t5.*t6.*t34.*t191.*1.652532002545242e-22;
t4887 = t4.*t5.*t6.*t34.*t191.*3.305064005090484e-22;
t4895 = t2.*t3.*t34.*t191.*2.750619948951613e-25;
t4897 = t7.*t9.*t34.*t191.*6.711642016684175e-22;
t4899 = t5.*t8.*t9.*t17.*t34.*t190.*t191.*5.659386953851025e-22;
t4900 = t6.*t7.*t34.*t191.*2.750619948951613e-25;
t4908 = t7.*t8.*t9.*t34.*t191.*1.258783598220194e-23;
t4909 = t4.*t6.*t9.*t34.*t191.*6.816747032177104e-22;
t4910 = t4.*t6.*t9.*t34.*t191.*1.363349406435421e-21;
t4911 = t5.*t6.*t8.*t34.*t191.*6.816747032177104e-22;
t4913 = t4.*t5.*t17.*t34.*t190.*t191.*4.945250784909262e-23;
t4915 = t2.*t4.*t5.*t7.*t34.*t191.*9.824811603756039e-23;
t4916 = t4.*t9.*t34.*t191.*7.513901495500154e-22;
t4919 = t4.*t34.*t191.*7.627193995348953e-22;
t4920 = t2.*t7.*t8.*t9.*t34.*t191.*(-1.964962320751208e-22);
t4923 = t5.*t6.*t7.*t8.*t34.*t191.*9.824811603756039e-23;
t4924 = t4.*t5.*t34.*t191.*4.105845905084658e-20;
t4925 = t8.*t34.*t191.*4.10367421232762e-22;
t4927 = t4.*t9.*t34.*t191.*4.105845905084658e-20;
t4928 = t4.*t17.*t19.*t34.*t190.*t191.*2.829693476925513e-22;
t4930 = t5.*t8.*t34.*t191.*1.128897292845565e-21;
t4933 = t4.*t9.*t34.*t191.*2.117272334812676e-23;
t4934 = t3.*t9.*t34.*t191.*1.149373463017392e-23;
t4937 = t4.*t34.*t191.*7.663981802980751e-22;
t4938 = t3.*t5.*t34.*t191.*7.06972457001642e-20;
t4941 = t2.*t4.*t7.*t34.*t191.*1.068001671898062e-22;
t4942 = t2.*t3.*t9.*t34.*t191.*1.068001671898062e-22;
t4943 = t2.*t5.*t7.*t34.*t191.*1.068001671898062e-22;
t4944 = t3.*t5.*t6.*t34.*t191.*1.068001671898062e-22;
t4945 = t4.*t7.*t34.*t191.*7.06972457001642e-20;
t4946 = t3.*t9.*t34.*t191.*7.06972457001642e-20;
t4948 = t8.*t17.*t24.*t34.*t190.*t191.*1.859969757595868e-22;
t4951 = t2.*t5.*t8.*t34.*t191.*(-3.305064005090484e-22);
t4955 = t4.*t9.*t34.*t191.*3.775071432955494e-22;
t4956 = t4.*t9.*t34.*t191.*7.550142865910989e-22;
t4957 = t5.*t8.*t34.*t191.*3.775071432955494e-22;
t4962 = t7.*t8.*t9.*t34.*t191.*2.114674168334142e-23;
t4964 = t6.*t8.*t34.*t191.*7.4101138229338e-22;
t4969 = t2.*t7.*t34.*t191.*1.134639471113644e-24;
t4970 = t3.*t6.*t34.*t191.*1.134639471113644e-24;
t4973 = t3.*t5.*t34.*t191.*6.50017459985076e-22;
t4974 = t3.*t5.*t34.*t191.*1.300034919970152e-21;
t4976 = t4.*t5.*t9.*t17.*t34.*t190.*t191.*1.859969757595868e-22;
t4980 = t4.*t7.*t34.*t191.*1.300034919970152e-21;
t4981 = t2.*t4.*t5.*t34.*t191.*6.816747032177104e-22;
t4982 = t2.*t4.*t5.*t34.*t191.*1.363349406435421e-21;
t4983 = t7.*t8.*t34.*t191.*2.146558632488979e-23;
t4986 = t7.*t9.*t34.*t191.*6.50017459985076e-22;
t4987 = t2.*t4.*t5.*t34.*t191.*8.981886944827752e-23;
t4988 = t2.*t4.*t5.*t34.*t191.*1.79637738896555e-22;
t4991 = t5.*t6.*t8.*t34.*t191.*(-1.363349406435421e-21);
t4993 = t6.*t7.*t34.*t191.*2.138348551163959e-24;
t4996 = t2.*t8.*t9.*t34.*t191.*8.981886944827752e-23;
t4998 = t4.*t6.*t9.*t34.*t191.*8.981886944827752e-23;
t4999 = t4.*t6.*t9.*t34.*t191.*1.79637738896555e-22;
t5000 = t2.*t5.*t7.*t8.*t34.*t191.*4.052766012304177e-22;
t5001 = t2.*t5.*t7.*t8.*t34.*t191.*8.105532024608353e-22;
t5004 = t4.*t5.*t6.*t7.*t34.*t191.*4.052766012304177e-22;
t5006 = t8.*t9.*t17.*t34.*t190.*t191.*(-4.945250784909262e-23);
t5008 = t2.*t7.*t8.*t9.*t34.*t191.*(-9.824811603756039e-23);
t5019 = t8.*t17.*t19.*t34.*t190.*t191.*(-1.859969757595868e-22);
t5021 = t2.*t3.*t9.*t34.*t191.*5.340008359490312e-23;
t5022 = t2.*t5.*t7.*t34.*t191.*5.340008359490312e-23;
t5023 = t3.*t5.*t6.*t34.*t191.*5.340008359490312e-23;
t5026 = t2.*t7.*t34.*t191.*5.183835334822626e-25;
t5027 = t3.*t6.*t34.*t191.*5.183835334822626e-25;
t5029 = t5.*t7.*t34.*t191.*3.647929947206127e-22;
t5034 = t3.*t34.*t191.*2.939200727657104e-23;
t5035 = t3.*t5.*t8.*t34.*t191.*6.711642016684175e-22;
t5036 = t4.*t5.*t7.*t34.*t191.*6.711642016684175e-22;
t5038 = t4.*t7.*t34.*t191.*6.017331709873085e-22;
t5045 = t5.*t18.*t22.*t34.*t190.*t191.*(-9.098517085411002e-23);
t5046 = t3.*t34.*t191.*6.380337905361116e-25;
t5051 = t4.*t34.*t191.*3.074086441795793e-23;
t5052 = t2.*t3.*t5.*t34.*t191.*2.202770420197048e-22;
t5053 = t2.*t3.*t5.*t34.*t191.*4.405540840394095e-22;
t5060 = t2.*t3.*t34.*t191.*2.138348551163959e-24;
t5062 = t4.*t6.*t7.*t34.*t191.*4.405540840394095e-22;
t5063 = t3.*t6.*t9.*t34.*t191.*2.202770420197048e-22;
t5064 = t3.*t6.*t9.*t34.*t191.*4.405540840394095e-22;
t5065 = t5.*t6.*t7.*t34.*t191.*2.202770420197048e-22;
t5066 = t5.*t6.*t7.*t34.*t191.*4.405540840394095e-22;
t5069 = t7.*t8.*t34.*t191.*1.31963648196326e-21;
t5071 = t2.*t8.*t34.*t191.*2.608176229845321e-22;
t5072 = t4.*t6.*t34.*t191.*2.608176229845321e-22;
t5073 = t2.*t8.*t9.*t34.*t191.*(-1.79637738896555e-22);
t5078 = t5.*t9.*t17.*t18.*t34.*t190.*t191.*1.414846738462756e-22;
t5080 = t5.*t7.*t8.*t34.*t191.*1.149373463017392e-23;
t5082 = t5.*t9.*t18.*t22.*t34.*t190.*t191.*1.414846738462756e-22;
t5083 = t6.*t7.*t8.*t9.*t34.*t191.*(-8.105532024608353e-22);
t5084 = t6.*t7.*t8.*t9.*t34.*t191.*(-4.052766012304177e-22);
t5085 = t246+t253+t725;
t5091 = t5.*t7.*t8.*t34.*t191.*7.06972457001642e-20;
t5093 = t7.*t8.*t9.*t34.*t191.*7.06972457001642e-20;
t5095 = t4.*t17.*t34.*t190.*t191.*1.41198189047744e-22;
t5096 = t6.*t7.*t8.*t9.*t34.*t191.*1.068001671898062e-22;
t5097 = t2.*t4.*t9.*t34.*t191.*3.7050569114669e-22;
t5098 = t2.*t4.*t9.*t34.*t191.*7.4101138229338e-22;
t5099 = t4.*t5.*t6.*t34.*t191.*3.7050569114669e-22;
t5100 = t4.*t5.*t6.*t34.*t191.*7.4101138229338e-22;
t5102 = t7.*t34.*t191.*2.657349319345957e-22;
t5107 = t6.*t8.*t9.*t34.*t191.*3.7050569114669e-22;
t5111 = t4.*t7.*t34.*t191.*7.065985201808775e-22;
t5112 = t3.*t9.*t34.*t191.*3.532992600904388e-22;
t5113 = t3.*t9.*t34.*t191.*7.065985201808775e-22;
t5114 = t5.*t7.*t34.*t191.*3.532992600904388e-22;
t5116 = t8.*t9.*t34.*t191.*6.135813310146999e-22;
t5119 = t7.*t8.*t34.*t191.*1.827639047097822e-23;
t5120 = t17.*t18.*t19.*t34.*t190.*t191.*9.299848787979342e-23;
t5122 = t4.*t5.*t7.*t34.*t191.*6.50017459985076e-22;
t5127 = t18.*t19.*t22.*t34.*t190.*t191.*9.299848787979342e-23;
t5130 = t7.*t8.*t9.*t34.*t191.*1.300034919970152e-21;
t5139 = t4.*t5.*t34.*t191.*4.10367421232762e-22;
t5142 = t22.*t34.*t190.*t191.*2.249538916123785e-22;
t5147 = t2.*t8.*t34.*t191.*1.30408811492266e-22;
t5149 = t4.*t6.*t34.*t191.*1.30408811492266e-22;
t5150 = t8.*t9.*t34.*t191.*2.05183710616381e-22;
t5151 = t4.*t5.*t34.*t191.*4.083976203983189e-22;
t5154 = t4.*t5.*t34.*t190.*t191.*2.341111640349547e-29;
t5158 = t8.*t9.*t34.*t190.*t191.*2.341111640349547e-29;
t5165 = t2.*t4.*t7.*t9.*t34.*t191.*5.340008359490312e-23;
t5171 = t3.*t8.*t9.*t34.*t191.*3.647929947206127e-22;
t5172 = t4.*t7.*t9.*t34.*t191.*3.647929947206127e-22;
t5176 = t6.*t7.*t8.*t9.*t34.*t191.*5.340008359490312e-23;
t5179 = t4.*t9.*t17.*t34.*t190.*t191.*3.570477686932346e-29;
t5180 = t5.*t8.*t17.*t34.*t190.*t191.*3.570477686932346e-29;
t5181 = t9.*t18.*t22.*t34.*t190.*t191.*(-4.945250784909262e-23);
t5183 = t6.*t8.*t9.*t34.*t191.*(-7.4101138229338e-22);
t5184 = t2.*t3.*t8.*t34.*t191.*7.753205398793312e-23;
t5185 = t2.*t3.*t8.*t34.*t191.*1.550641079758662e-22;
t5186 = t2.*t4.*t7.*t34.*t191.*7.753205398793312e-23;
t5187 = t2.*t4.*t7.*t34.*t191.*1.550641079758662e-22;
t5192 = t6.*t7.*t8.*t34.*t191.*7.753205398793312e-23;
t5193 = t6.*t7.*t8.*t34.*t191.*1.550641079758662e-22;
t5199 = t2.*t7.*t34.*t191.*2.49373386785477e-22;
t5200 = t3.*t6.*t34.*t191.*2.49373386785477e-22;
t5203 = t7.*t8.*t9.*t34.*t191.*(-6.50017459985076e-22);
t5204 = t2.*t7.*t8.*t9.*t34.*t191.*2.202770420197048e-22;
t5205 = t2.*t7.*t8.*t9.*t34.*t191.*4.405540840394095e-22;
t5208 = t4.*t6.*t7.*t9.*t34.*t191.*2.202770420197048e-22;
t5215 = t4.*t5.*t34.*t191.*2.05183710616381e-22;
t5216 = t17.*t34.*t190.*t191.*2.249538916123785e-22;
t5217 = t8.*t34.*t191.*2.979080454187173e-22;
t5222 = t2.*t7.*t8.*t34.*t191.*6.396443737329302e-22;
t5223 = t3.*t6.*t8.*t34.*t191.*6.396443737329302e-22;
t5224 = t4.*t6.*t7.*t34.*t191.*6.396443737329302e-22;
t5227 = t7.*t34.*t191.*6.635617427383666e-22;
t5236 = t2.*t4.*t34.*t191.*5.379404921299311e-22;
t5237 = t2.*t4.*t34.*t191.*1.075880984259862e-21;
t5238 = t8.*t34.*t191.*4.709632483796753e-22;
t5239 = t3.*t8.*t34.*t191.*5.29646177628791e-22;
t5240 = t4.*t7.*t34.*t191.*5.29646177628791e-22;
t5244 = t6.*t8.*t34.*t191.*5.379404921299311e-22;
t5245 = t6.*t8.*t34.*t191.*1.075880984259862e-21;
t5250 = t4.*t7.*t9.*t34.*t191.*3.532992600904388e-22;
t5252 = t5.*t7.*t8.*t34.*t191.*7.065985201808775e-22;
t5258 = t3.*t8.*t34.*t191.*5.227462873124012e-22;
t5267 = t2.*t3.*t34.*t191.*1.028673146211772e-21;
t5270 = t6.*t7.*t34.*t191.*1.028673146211772e-21;
t5271 = t8.*t34.*t191.*8.908641649909366e-22;
t5279 = t2.*t7.*t8.*t34.*t191.*3.198221868664651e-22;
t5280 = t3.*t6.*t8.*t34.*t191.*3.198221868664651e-22;
t5281 = t4.*t6.*t7.*t34.*t191.*3.198221868664651e-22;
t5285 = t3.*t34.*t191.*4.111372393705095e-23;
t5293 = t4.*t8.*t9.*t22.*t34.*t190.*t191.*3.570477686932346e-29;
t5294 = t221+t341+t821;
t5305 = t4.*t7.*t34.*t191.*2.21879701818747e-22;
t5318 = t3.*t8.*t34.*t191.*5.129583225941468e-22;
t5319 = t4.*t7.*t34.*t191.*5.129583225941468e-22;
t5321 = t216+t375+t819;
t5324 = t3.*t34.*t191.*2.199486848951818e-23;
t5325 = t4.*t5.*t17.*t34.*t190.*t191.*4.682223280699094e-29;
t5327 = t4.*t8.*t9.*t17.*t34.*t190.*t191.*(-3.570477686932346e-29);
t5328 = t17.*t18.*t34.*t190.*t191.*3.34878210114812e-23;
t5331 = t18.*t22.*t34.*t190.*t191.*3.34878210114812e-23;
t5332 = t8.*t9.*t17.*t34.*t190.*t191.*4.682223280699094e-29;
t5353 = t2.*t3.*t5.*t34.*t191.*2.062334050925814e-29;
t5355 = t3.*t34.*t191.*2.199487072107542e-23;
t5356 = t2.*t3.*t9.*t34.*t191.*2.062334050925814e-29;
t5358 = t281+t345+t816;
t5362 = t3.*t5.*t6.*t34.*t191.*8.507193506300311e-29;
t5364 = t3.*t6.*t9.*t34.*t191.*8.507193506300311e-29;
t5368 = t4.*t5.*t8.*t22.*t34.*t190.*t191.*4.682223280699094e-29;
t5372 = t2.*t4.*t5.*t34.*t191.*3.468843125491349e-29;
t5373 = t2.*t4.*t9.*t34.*t191.*3.468843125491349e-29;
t5376 = t3.*t5.*t34.*t191.*1.364456842013169e-28;
t5378 = t3.*t9.*t34.*t191.*1.364456842013169e-28;
t5387 = t4.*t5.*t8.*t17.*t34.*t190.*t191.*(-4.682223280699094e-29);
t5389 = t4.*t5.*t6.*t34.*t191.*1.430908814132556e-28;
t5390 = t4.*t6.*t9.*t34.*t191.*1.430908814132556e-28;
t5391 = t4.*t5.*t34.*t191.*7.924282596813391e-29;
t5392 = t4.*t9.*t34.*t191.*7.924282596813391e-29;
t5393 = t2.*t5.*t7.*t8.*t34.*t191.*2.062334050925814e-29;
t5394 = t2.*t7.*t8.*t9.*t34.*t191.*2.062334050925814e-29;
t5402 = t5.*t6.*t7.*t8.*t34.*t191.*8.507193506300311e-29;
t5404 = t6.*t7.*t8.*t9.*t34.*t191.*8.507193506300311e-29;
t5409 = t7.*t8.*t9.*t34.*t191.*1.364456842013169e-28;
t5416 = t5.*t7.*t8.*t34.*t191.*1.364456842013169e-28;
t5420 = t8.*t34.*t191.*3.954196685357393e-23;
t5424 = t4.*t7.*t34.*t191.*2.350891687301493e-23;
t5429 = t6.*t8.*t34.*t191.*1.677448243266967e-22;
t5430 = t6.*t8.*t34.*t191.*3.354896486533935e-22;
t5434 = t2.*t3.*t4.*t34.*t191.*1.994589265414034e-22;
t5435 = t2.*t7.*t8.*t34.*t191.*1.994589265414034e-22;
t5436 = t4.*t6.*t7.*t34.*t191.*1.994589265414034e-22;
t5439 = t2.*t4.*t34.*t191.*1.677448243266967e-22;
t5440 = t2.*t4.*t34.*t191.*3.354896486533935e-22;
t5441 = t4.*t34.*t191.*1.145918371200067e-21;
t5445 = t4.*t8.*t17.*t34.*t190.*t191.*8.273795699471084e-23;
t5449 = t4.*t8.*t22.*t34.*t190.*t191.*8.273795699471084e-23;
t5450 = t2.*t8.*t34.*t191.*6.919527317055843e-22;
t5451 = t2.*t8.*t34.*t191.*1.383905463411169e-21;
t5452 = t4.*t6.*t34.*t191.*6.919527317055843e-22;
t5453 = t4.*t6.*t34.*t191.*1.383905463411169e-21;
t5455 = t2.*t3.*t4.*t34.*t191.*9.972946327070171e-23;
t5456 = t2.*t7.*t8.*t34.*t191.*9.972946327070171e-23;
t5457 = t4.*t6.*t7.*t34.*t191.*9.972946327070171e-23;
t5467 = t2.*t4.*t7.*t34.*t191.*4.113872056481154e-22;
t5468 = t2.*t4.*t7.*t34.*t191.*8.227744112962308e-22;
t5469 = t3.*t4.*t6.*t34.*t191.*4.113872056481154e-22;
t5470 = t3.*t4.*t6.*t34.*t191.*8.227744112962308e-22;
t5471 = t4.*t34.*t191.*3.831990505276246e-22;
t5472 = t6.*t7.*t8.*t34.*t191.*4.113872056481154e-22;
t5473 = t6.*t7.*t8.*t34.*t191.*8.227744112962308e-22;
t5474 = t3.*t4.*t34.*t191.*6.812837568642129e-22;
t5475 = t7.*t8.*t34.*t191.*6.812837568642129e-22;
t5476 = t3.*t4.*t34.*t191.*6.812837590836777e-22;
t5477 = t3.*t4.*t34.*t191.*6.598181727587879e-22;
t5478 = t7.*t8.*t34.*t191.*6.598181727587879e-22;
t5489 = t5.*t34.*t190.*t191.*4.649659540105436e-23;
t5490 = t9.*t34.*t190.*t191.*2.527195615990709e-23;
t5493 = t19.*t34.*t190.*t191.*2.295061777172614e-22;
t5494 = t5.*t9.*t34.*t190.*t191.*3.491627384523043e-22;
t5497 = t6.*t34.*t191.*1.287153880979138e-21;
t5499 = t34.*t191.*6.27710454902646e-22;
t5501 = t5.*t18.*t34.*t190.*t191.*8.504783013603662e-23;
t5508 = t5.*t17.*t34.*t190.*t191.*2.245376163391997e-22;
t5510 = t6.*t34.*t191.*5.325743171835082e-21;
t5512 = t2.*t34.*t191.*2.196885984950864e-20;
t5516 = t18.*t19.*t34.*t190.*t191.*8.69297658713101e-23;
t5517 = t5.*t9.*t18.*t34.*t190.*t191.*1.32251930673679e-22;
t5521 = t2.*t34.*t191.*5.309550668069175e-21;
t5532 = t17.*t19.*t34.*t190.*t191.*4.590123554345229e-22;
t5535 = t5.*t9.*t17.*t34.*t190.*t191.*6.983254769046087e-22;
t5540 = t9.*t18.*t34.*t190.*t191.*4.62254282524179e-23;
t5547 = t9.*t17.*t34.*t190.*t191.*1.220412967321392e-22;
t5557 = t4.*t8.*t9.*t34.*t190.*t191.*3.337482108041939e-29;
t5558 = t18.*t34.*t190.*t191.*3.130253519639126e-23;
t5574 = t4.*t5.*t8.*t34.*t190.*t191.*4.376679479718804e-29;
t5578 = t17.*t34.*t190.*t191.*5.551521213260268e-22;
t5579 = t17.*t18.*t34.*t190.*t191.*8.26428684556577e-23;
t5582 = t4.*t8.*t9.*t17.*t34.*t190.*t191.*8.811397961779761e-29;
t5586 = t4.*t5.*t8.*t17.*t34.*t190.*t191.*1.155501764459885e-28;
t5590 = t220+t222+t254+t279;
t5593 = t4.*t8.*t34.*t190.*t191.*7.733879758902498e-23;
t5596 = t4.*t8.*t17.*t34.*t190.*t191.*2.041847420845766e-22;
t5604 = t4.*t5.*t34.*t190.*t191.*1.257741436603469e-21;
t5607 = t4.*t9.*t34.*t190.*t191.*6.836110509205297e-22;
t5612 = t4.*t34.*t190.*t191.*9.925409351190054e-22;
t5629 = t8.*t34.*t190.*t191.*1.276705177306726e-21;
t5634 = t219+t285+t376+t818;
t5635 = t34.*t190.*t191.*8.524037848249721e-21;
t5688 = t226+t241+t248+t256+t727;
t5741 = t237+t247+t332+t355+t1058;
t5743 = t245+t259+t308+t366+t1062;
t5779 = t264+t395+t443+t855+t864;
t5780 = t307+t329+t398+t791+t1063;
t5782 = t223+t242+t269+t293+t296+t404;
t5826 = t288+t354+t401+t419+t857+t904;
t5886 = t247+t286+t312+t332+t360+t793+t997;
t5887 = t238+t272+t321+t334+t367+t788+t1062;
t5894 = t261+t289+t389+t421+t426+t851+t862;
t103 = t30+t31;
t199 = t4.*t196;
t200 = t8.*t196;
t201 = t4.*t197;
t202 = t8.*t197;
t204 = t196.*(3.0./5.0e+2);
t205 = t197.*(3.0./5.0e+2);
t616 = (t5.*t594)./2.0;
t619 = (t9.*t600)./2.0;
t622 = (t4.*t9.*t594)./2.0;
t624 = (t4.*t5.*t600)./2.0;
t627 = t196.*8.112963841460668e+31;
t628 = t197.*8.112963841460668e+31;
t630 = t196.*5.110348748545983e-1;
t631 = t197.*5.110348748545983e-1;
t635 = t32.*t197;
t636 = t33.*t197;
t637 = -t634;
t639 = t196.*3.06620924912759e-3;
t641 = t25.*t198.*3.563742084504373e+31;
t642 = t26.*t198.*3.563742084504373e+31;
t648 = -t644;
t649 = t196.*2.659783725725934e-6;
t650 = t197.*2.659783725725934e-6;
t651 = t5.*t644;
t652 = t9.*t644;
t653 = t196.*8.01825475553694e-7;
t654 = t197.*8.01825475553694e-7;
t657 = t196.*4.36041e-5;
t658 = t197.*4.36041e-5;
t678 = t196.*4.35810366141993e-7;
t679 = t197.*4.35810366141993e-7;
t684 = t73.*t197;
t710 = t5.*t196.*(-8.01825475553694e-7);
t712 = -t681;
t741 = t118.*t196;
t742 = t115.*t197;
t743 = t116.*t197;
t754 = t121.*t197;
t760 = t196.*1.308123e-7;
t767 = t9.*t75.*t196;
t773 = t104.*t196;
t777 = t106.*t196;
t778 = t107.*t196;
t779 = t104.*t197;
t781 = t5.*t9.*t197.*1.639136489385872e-6;
t783 = t109.*t196;
t784 = t106.*t197;
t790 = t19.*t197.*1.246862701090643e-6;
t792 = t24.*t197.*1.246862701090643e-6;
t794 = t19.*t196.*8.195682446929358e-7;
t796 = t114.*t196;
t798 = t111.*t197;
t800 = t113.*t197;
t801 = t116.*t196;
t817 = t5.*t9.*t196.*(-1.246862701090643e-6);
t831 = t9.*t196.*(-4.35810366141993e-7);
t832 = t5.*t197.*(-4.35810366141993e-7);
t863 = t133.*t196;
t868 = t135.*t196;
t869 = t132.*t197;
t870 = t133.*t197;
t872 = t134.*t197;
t878 = t136.*t197;
t881 = t5.*t196.*1.573278338878372e-13;
t889 = t9.*t197.*1.573278338878372e-13;
t890 = t142.*t197;
t925 = t147.*t197;
t929 = t9.*t197.*(-3.146556677756745e-13);
t954 = t143.*t197;
t955 = t145.*t197;
t973 = t196.*2.332787412311698e-6;
t975 = t19.*t23.*t196.*(-8.195682446929358e-7);
t1009 = t9.*t196.*2.063152639848858e-13;
t1010 = t5.*t197.*2.063152639848858e-13;
t1011 = t151.*t197;
t1018 = t155.*t196;
t1022 = t152.*t197;
t1046 = t9.*t18.*t197.*6.293113355513489e-13;
t1076 = t5.*t197.*(-4.126305279697715e-13);
t1082 = t162.*t197;
t1107 = t18.*t140.*t196;
t1120 = t18.*t196.*2.951182896698924e-7;
t1122 = t23.*t196.*2.951182896698924e-7;
t1136 = t168.*t196;
t1146 = t9.*t153.*t196;
t1148 = t169.*t197;
t1184 = t5.*t18.*t196.*(-3.146556677756745e-13);
t1227 = t18.*t154.*t196;
t1228 = t5.*t18.*t197.*8.252610559395431e-13;
t1265 = t179.*t196;
t1267 = t180.*t196;
t1268 = t181.*t196;
t1269 = t179.*t197;
t1270 = t182.*t196;
t1271 = t180.*t197;
t1277 = t9.*t18.*t196.*(-4.126305279697715e-13);
t1334 = -t1299;
t1422 = -t1399;
t1430 = t4.*t1398;
t1432 = t8.*t1398;
t1439 = t18.*t197.*1.458290424491263e-6;
t1442 = -t1435;
t1450 = t8.*t1435;
t1452 = t5.*t1447;
t1455 = t9.*t1447;
t1458 = (t91.*t196)./9.007199254740992e+15;
t1459 = (t91.*t197)./9.007199254740992e+15;
t1466 = t196.*(t29-t30).*(-1.110223024625157e-16);
t1467 = t197.*(t29-t30).*(-1.110223024625157e-16);
t1468 = t617+5.994209437267293e+31;
t1474 = (t196.*(t29-t30))./9.007199254740992e+15;
t1480 = t196.*4.146007461420734e+31;
t1492 = t197.*8.851959439560906e-2;
t1498 = t196.*2.228321578664739e-5;
t1499 = t196.*4.097607815548108e-7;
t1506 = t196.*1.35924224341665e-6;
t1508 = -t1496;
t1511 = -t1497;
t1524 = t196.*2.227142959217101e-7;
t1530 = -t1514;
t1534 = -t1517;
t1536 = -t1519;
t1537 = -t1518;
t1538 = -t1520;
t1539 = t194.*t260;
t1543 = t195.*t260;
C_dq = ft_6({dq1,dq2,dq3,dq4,dq5,dq6,t1003,t1004,t1006,t1008,t1009,t101,t1010,t1012,t1013,t1015,t1016,t102,t1023,t1024,t1025,t1026,t1027,t1028,t1030,t1032,t1033,t1034,t1038,t1039,t1040,t1041,t1042,t1043,t1044,t1045,t1046,t1047,t1048,t1049,t1050,t1051,t1054,t1055,t1056,t1057,t1059,t1061,t1064,t1065,t1066,t1068,t1069,t1070,t1071,t1073,t1076,t1078,t1080,t1081,t1083,t1084,t1085,t1091,t1092,t1093,t1094,t1095,t1097,t1098,t1099,t110,t1100,t1101,t1102,t1105,t1106,t1107,t1108,t1109,t111,t1111,t1113,t1115,t1116,t1119,t112,t1120,t1122,t1123,t1125,t1126,t1127,t1128,t1129,t113,t1130,t1131,t1132,t1133,t1134,t1138,t1139,t114,t1140,t1141,t1144,t1146,t1148,t115,t1150,t1151,t1152,t1153,t1155,t1158,t1159,t116,t1161,t1162,t1163,t1166,t1167,t1169,t1170,t1171,t1173,t1174,t1175,t1176,t1177,t1178,t1179,t1180,t1181,t1182,t1183,t1184,t1185,t1186,t1187,t1188,t1189,t1190,t1191,t1192,t1193,t1195,t1196,t1197,t1198,t1199,t120,t1203,t1204,t1205,t1206,t1207,t1208,t121,t1210,t1214,t1215,t1216,t1219,t1221,t1222,t1223,t1224,t1225,t1226,t1227,t1228,t1229,t1230,t1232,t1233,t1236,t124,t1240,t1242,t1244,t1245,t125,t1250,t1251,t1253,t1254,t1256,t1257,t1258,t1259,t126,t1260,t1261,t1262,t1263,t1264,t1265,t1266,t1267,t1268,t1269,t1271,t1272,t1273,t1274,t1276,t1277,t1278,t1279,t128,t1280,t1282,t1284,t1285,t1286,t1287,t1288,t129,t1290,t1293,t1294,t1295,t1296,t1297,t1298,t130,t1300,t1301,t1302,t1304,t1306,t1307,t1308,t1309,t131,t1312,t1313,t1315,t1316,t1319,t132,t1320,t1321,t1322,t1323,t1324,t1325,t1326,t1328,t1329,t133,t1330,t1331,t1332,t1333,t1334,t1335,t1337,t1338,t1339,t134,t1340,t1341,t1342,t1343,t1344,t1345,t1346,t1347,t1348,t1351,t1352,t1353,t1354,t1355,t1356,t1358,t136,t1360,t1362,t1364,t1365,t1366,t1367,t1368,t1369,t1370,t1371,t1372,t1373,t1374,t1375,t1377,t1378,t1379,t1380,t1382,t1383,t1384,t1385,t1386,t1387,t1388,t1389,t139,t1391,t1392,t1393,t1394,t1397,t1398,t140,t1401,t1402,t1403,t1404,t1405,t1406,t1407,t1408,t1409,t141,t1410,t1411,t1413,t1414,t1415,t1416,t1417,t1418,t1419,t142,t1421,t1422,t1423,t1424,t1426,t1427,t1428,t1429,t143,t1430,t1431,t1432,t1433,t1434,t1436,t1439,t144,t1440,t1442,t1443,t1444,t1445,t1447,t1448,t1449,t145,t1451,t1452,t1453,t1454,t1455,t1456,t1457,t1458,t1459,t1460,t1461,t1463,t1464,t1467,t1468,t1469,t147,t1470,t1471,t1472,t1473,t1474,t1475,t1476,t1478,t1479,t148,t1480,t1481,t1482,t1483,t1485,t1486,t1487,t1488,t1489,t1492,t1494,t1496,t1498,t1499,t15,t150,t1501,t1503,t1505,t1506,t1508,t151,t1511,t1513,t1514,t1515,t1517,t1520,t1521,t1522,t1523,t1524,t1527,t1528,t1529,t153,t1530,t1531,t1532,t1533,t1534,t1535,t1536,t1537,t1538,t1539,t154,t1541,t1542,t1545,t1548,t1549,t1550,t1555,t1556,t1558,t156,t1560,t1561,t1562,t1566,t1567,t1568,t1569,t157,t1570,t1571,t158,t1580,t1587,t1589,t1591,t1593,t1595,t1596,t1597,t1598,t1599,t16,t1605,t1606,t161,t1610,t1611,t1612,t1619,t1620,t1621,t1622,t1623,t1625,t163,t1631,t1632,t1633,t1635,t1636,t1637,t1638,t1639,t1641,t1643,t1644,t1645,t165,t1650,t1651,t1652,t1653,t1657,t1658,t1659,t166,t1660,t1661,t1662,t1663,t1666,t1669,t1672,t1676,t1681,t1682,t1683,t1687,t1689,t1692,t1695,t1696,t1698,t17,t170,t1702,t1703,t1704,t1709,t171,t1711,t1712,t1713,t1716,t1720,t1722,t1726,t1728,t1729,t173,t1731,t1733,t1734,t1735,t1736,t1737,t1738,t1740,t1744,t1745,t1746,t1749,t175,t1752,t1755,t1756,t1757,t1758,t1760,t1761,t1764,t1767,t1769,t177,t1771,t1772,t1774,t1776,t1779,t1784,t1785,t1786,t1787,t1788,t1789,t1793,t1795,t1797,t1798,t1799,t18,t1800,t1801,t1803,t1804,t1807,t1808,t1809,t1810,t1811,t1812,t1814,t1816,t1817,t1820,t1826,t1827,t1829,t183,t1830,t1831,t1832,t1833,t1834,t1835,t1836,t1838,t1847,t1849,t185,t1850,t1851,t1855,t1857,t1858,t1859,t186,t1866,t1867,t1871,t1872,t1873,t1881,t1882,t1888,t1889,t1896,t19,t190,t1903,t1907,t1908,t191,t1910,t1911,t1912,t1913,t1914,t1915,t1916,t1920,t1925,t1926,t193,t1930,t1935,t1936,t1937,t1938,t1939,t194,t1943,t1944,t1946,t195,t1950,t1955,t196,t1961,t1964,t1965,t1966,t1967,t1968,t1969,t197,t1970,t1972,t1976,t1977,t1978,t1979,t1981,t1984,t1988,t199,t1992,t1994,t1995,t1996,t1997,t1998,t1999,t2,t20,t200,t2000,t2001,t2002,t2003,t2004,t2005,t2006,t201,t2014,t2017,t2019,t202,t2020,t2023,t2024,t2028,t2029,t2033,t2036,t2037,t2038,t204,t2042,t205,t2052,t2053,t2056,t2058,t2059,t206,t2060,t2062,t2065,t2066,t2067,t2068,t2069,t207,t2070,t2072,t2073,t2074,t2079,t2081,t2082,t2083,t2084,t2085,t2086,t2087,t2093,t2094,t2096,t2097,t2098,t21,t2100,t2103,t2104,t2105,t2106,t2108,t2109,t2110,t2111,t2113,t2114,t2115,t2116,t2117,t2118,t2121,t2122,t2126,t2128,t2129,t2130,t2131,t2132,t2133,t2136,t2142,t2144,t2148,t2149,t215,t2154,t2156,t2157,t2158,t2171,t2172,t2175,t2176,t2179,t2180,t2182,t2189,t2194,t2196,t22,t2204,t2208,t2212,t2214,t2217,t2218,t2219,t2220,t2221,t2223,t2225,t2227,t2228,t2229,t2236,t2239,t224,t2244,t225,t2251,t2254,t2256,t2257,t2264,t2265,t2266,t2267,t2269,t227,t2270,t2274,t2276,t2277,t2279,t228,t2280,t2281,t2282,t2285,t2291,t2294,t23,t230,t2302,t2304,t2305,t2306,t231,t2316,t2317,t2318,t2321,t2322,t2323,t2324,t233,t2333,t2336,t2339,t234,t2340,t2344,t2348,t235,t2350,t2357,t2358,t2359,t236,t2361,t2362,t2363,t2364,t2365,t2366,t2369,t2371,t2372,t2373,t2375,t2376,t2377,t2378,t2379,t2384,t2385,t2387,t2388,t2389,t239,t2391,t2394,t24,t240,t2400,t2401,t2402,t2403,t2405,t2406,t2407,t2410,t2417,t2418,t2419,t2421,t2422,t2428,t2429,t243,t2430,t2431,t2434,t2435,t2437,t2438,t2439,t244,t2440,t2441,t2442,t2443,t2444,t2447,t2449,t2450,t2452,t2453,t2454,t2455,t2456,t2457,t2458,t2460,t2466,t2467,t2468,t2470,t2472,t2474,t2477,t2481,t2483,t2484,t2485,t2486,t2487,t2489,t249,t2492,t2495,t2497,t2498,t2499,t25,t2500,t2501,t2502,t2503,t2504,t2505,t2506,t2513,t2518,t2521,t2527,t2533,t2535,t2536,t2537,t2538,t2540,t2543,t2544,t2545,t2546,t2549,t2551,t2552,t2553,t2554,t2555,t2557,t2558,t2559,t2560,t2561,t2562,t2565,t257,t2572,t2573,t2574,t2575,t2576,t2577,t2578,t2579,t258,t2583,t2584,t2590,t2591,t2592,t2593,t2595,t2596,t2597,t26,t2602,t2603,t2604,t2605,t2609,t2610,t2611,t2615,t2617,t2627,t263,t2652,t2655,t2656,t266,t2673,t2675,t2676,t2685,t2687,t270,t2705,t2706,t2707,t2708,t2716,t2719,t273,t274,t2749,t275,t2751,t2752,t276,t2764,t277,t278,t280,t2804,t284,t2854,t287,t2886,t29,t290,t291,t292,t2939,t294,t297,t299,t2997,t3,t30,t300,t302,t303,t304,t305,t3058,t306,t309,t310,t311,t313,t314,t3142,t315,t3158,t316,t318,t319,t3191,t320,t3208,t3211,t3212,t3218,t3219,t322,t3225,t3228,t3230,t3231,t324,t3243,t3244,t325,t3251,t3252,t3255,t3257,t3258,t3259,t3261,t3273,t3274,t3275,t3279,t328,t3282,t3286,t3288,t3289,t3290,t3294,t3295,t3309,t3314,t3317,t3319,t3320,t3321,t3326,t3327,t3328,t3329,t333,t3330,t3331,t3333,t3334,t3335,t3343,t336,t3363,t3364,t3365,t3367,t3368,t3369,t337,t3370,t3371,t3372,t3373,t3374,t3375,t3376,t3378,t3379,t3380,t3381,t3382,t3389,t3390,t3391,t3392,t3393,t3394,t3395,t3397,t34,t340,t3400,t3401,t3402,t3403,t3409,t3416,t3417,t3418,t3419,t3420,t3426,t3430,t3432,t3434,t3435,t3437,t3438,t3439,t344,t3440,t3442,t3443,t3444,t3445,t3446,t3447,t3449,t3450,t3452,t3453,t3454,t3455,t3456,t3459,t346,t3462,t3463,t3466,t3468,t3469,t347,t3470,t3472,t3473,t3475,t3477,t3479,t348,t3481,t3483,t3486,t3489,t349,t3492,t350,t3500,t3501,t3506,t3507,t3509,t3514,t3515,t3516,t3517,t3519,t352,t3520,t3521,t3522,t3523,t3524,t353,t3530,t3532,t3533,t3534,t3535,t3538,t3539,t3541,t3544,t3546,t3548,t3549,t3553,t3556,t356,t3560,t3568,t3569,t357,t3572,t3573,t3574,t3575,t3576,t3578,t3579,t358,t3581,t3582,t3583,t3584,t3585,t359,t3590,t3596,t3597,t3601,t3602,t3604,t3607,t3609,t361,t3613,t3616,t3617,t3618,t362,t3622,t3629,t3630,t3637,t3638,t3639,t3641,t3643,t3646,t3647,t3649,t365,t3650,t3652,t3653,t3654,t3659,t3660,t3662,t3663,t3668,t3676,t368,t3680,t3682,t3686,t369,t3691,t3695,t3697,t3701,t3709,t371,t3714,t3716,t3717,t372,t3722,t3726,t3729,t373,t3730,t3736,t3737,t3738,t374,t3743,t3744,t3747,t3748,t3750,t3751,t3756,t377,t3774,t378,t3789,t379,t3798,t380,t3815,t382,t3822,t3824,t3825,t3834,t3835,t3839,t384,t3846,t3847,t3852,t386,t387,t388,t3889,t3892,t3898,t3899,t391,t3915,t392,t395,t3950,t3951,t3958,t3959,t396,t4,t400,t4001,t4002,t4004,t4007,t401,t402,t4028,t4029,t403,t4030,t4031,t4032,t4033,t4039,t4040,t4041,t4042,t4043,t4044,t4045,t4051,t4052,t4058,t406,t409,t410,t4105,t411,t4113,t4114,t4117,t4118,t412,t4123,t413,t414,t4143,t4144,t4145,t415,t4150,t4152,t4153,t4155,t416,t4160,t4164,t4165,t417,t4170,t4174,t4177,t4178,t4179,t418,t4180,t4181,t4182,t4183,t4184,t4185,t4186,t4187,t4188,t4189,t4190,t4191,t4192,t4193,t4194,t4196,t4197,t420,t4200,t4203,t4204,t4205,t4206,t4207,t4208,t4209,t4211,t4212,t4213,t4214,t4216,t422,t4221,t4228,t4229,t423,t4230,t4231,t4232,t4233,t4235,t4236,t4237,t4239,t424,t4240,t4242,t4243,t4246,t4249,t425,t4255,t4256,t4257,t4258,t4259,t4260,t4261,t4262,t4265,t4266,t4268,t427,t4271,t4272,t4275,t4277,t4278,t4279,t428,t4283,t4284,t4287,t4288,t4289,t429,t4290,t4292,t4293,t4294,t4295,t4296,t4297,t4298,t4299,t4300,t4301,t4304,t4308,t4309,t431,t4310,t4311,t4313,t4315,t4316,t4317,t4319,t432,t4320,t4321,t4323,t4325,t4326,t4328,t433,t4330,t4333,t4334,t4335,t4336,t4337,t4338,t4339,t434,t4341,t4342,t4343,t4344,t4345,t4346,t4347,t435,t4351,t4353,t4355,t436,t4361,t4365,t4367,t4369,t437,t4370,t4371,t4372,t4375,t4377,t4379,t438,t4382,t4385,t4387,t439,t4390,t4391,t4392,t4394,t4395,t4396,t4397,t44,t440,t4401,t4402,t4403,t4404,t4405,t4406,t4407,t4408,t441,t4410,t4411,t4412,t4413,t4417,t4419,t442,t4420,t4421,t4422,t4425,t4426,t4428,t4429,t4431,t4432,t4435,t4436,t444,t4440,t4442,t4443,t4444,t4445,t4446,t4448,t4449,t445,t4450,t4452,t4453,t4455,t4457,t4459,t4462,t4464,t4469,t4473,t4478,t4479,t448,t4480,t4481,t4483,t4484,t4485,t4486,t4488,t449,t4491,t4492,t4493,t4495,t4498,t45,t450,t4501,t4502,t4504,t4506,t4508,t4509,t4513,t4516,t4517,t4519,t452,t4520,t4522,t4524,t4525,t453,t4530,t4532,t4533,t454,t4540,t4542,t4543,t4547,t4548,t4549,t4551,t4554,t4555,t4557,t4558,t4559,t4561,t4562,t4563,t4566,t4567,t4568,t4569,t457,t4570,t4571,t4572,t4574,t4575,t4577,t4579,t458,t4581,t4582,t4583,t4584,t4588,t4589,t459,t4590,t4591,t4595,t4596,t46,t460,t4600,t4601,t4605,t4606,t4607,t461,t4611,t4614,t4616,t4617,t462,t4621,t4622,t4625,t4626,t4628,t4629,t463,t4630,t4632,t4633,t4634,t4636,t4637,t4638,t4639,t464,t4640,t4641,t4642,t4643,t4644,t4645,t4646,t4647,t4649,t465,t4650,t4651,t4652,t4653,t4656,t4657,t4658,t466,t4660,t4661,t4662,t4663,t4666,t4667,t4669,t4672,t4673,t4674,t4675,t468,t4688,t469,t4691,t4692,t4693,t4694,t4695,t4696,t4697,t47,t470,t4707,t4708,t4709,t471,t4711,t4713,t4716,t472,t4722,t4723,t4724,t4725,t4726,t4727,t4728,t4731,t4732,t4733,t4734,t4737,t4740,t4741,t4742,t4745,t4747,t4748,t4749,t475,t4752,t4753,t4754,t4755,t4756,t4758,t4759,t4760,t4761,t4763,t4766,t4769,t477,t4770,t4777,t4778,t4782,t4783,t4785,t4786,t4788,t4789,t479,t4790,t4794,t4795,t4796,t4797,t4798,t4799,t480,t4800,t4801,t4803,t4804,t4805,t4807,t4808,t481,t4811,t4813,t4814,t4815,t4818,t482,t4820,t4824,t4825,t4827,t4828,t483,t4830,t4832,t4833,t4834,t4835,t4837,t4839,t484,t4841,t4842,t4845,t4846,t4849,t485,t4852,t486,t4861,t4862,t4864,t4865,t4866,t4867,t4871,t4872,t4873,t4876,t4877,t4878,t4879,t488,t4882,t4883,t4884,t4886,t4887,t489,t4895,t4897,t4899,t4900,t4908,t4909,t491,t4910,t4911,t4913,t4915,t4916,t4919,t492,t4920,t4923,t4924,t4925,t4927,t4928,t493,t4930,t4933,t4934,t4937,t4938,t494,t4941,t4942,t4943,t4944,t4945,t4946,t4948,t4951,t4955,t4956,t4957,t496,t4962,t4964,t4969,t497,t4970,t4973,t4974,t4976,t498,t4980,t4981,t4982,t4983,t4986,t4987,t4988,t499,t4991,t4993,t4996,t4998,t4999,t5,t50,t500,t5000,t5001,t5004,t5006,t5008,t501,t5019,t502,t5021,t5022,t5023,t5026,t5027,t5029,t503,t5034,t5035,t5036,t5038,t504,t5045,t5046,t505,t5051,t5052,t5053,t506,t5060,t5062,t5063,t5064,t5065,t5066,t5069,t507,t5071,t5072,t5073,t5078,t508,t5080,t5082,t5083,t5084,t5085,t509,t5091,t5093,t5095,t5096,t5097,t5098,t5099,t510,t5100,t5102,t5107,t511,t5111,t5112,t5113,t5114,t5116,t5119,t512,t5120,t5122,t5127,t513,t5130,t5139,t514,t5142,t5147,t5149,t5150,t5151,t5154,t5158,t516,t5165,t517,t5171,t5172,t5176,t5179,t518,t5180,t5181,t5183,t5184,t5185,t5186,t5187,t5192,t5193,t5199,t520,t5200,t5203,t5204,t5205,t5208,t521,t5215,t5216,t5217,t522,t5222,t5223,t5224,t5227,t523,t5236,t5237,t5238,t5239,t524,t5240,t5244,t5245,t525,t5250,t5252,t5258,t526,t5267,t527,t5270,t5271,t5279,t528,t5280,t5281,t5285,t529,t5293,t5294,t53,t530,t5305,t531,t5318,t5319,t532,t5321,t5324,t5325,t5327,t5328,t533,t5331,t5332,t534,t535,t5353,t5355,t5356,t5358,t536,t5361,t5362,t5364,t5368,t537,t5372,t5373,t5376,t5378,t538,t5387,t5389,t539,t5390,t5391,t5392,t5393,t5394,t540,t5402,t5404,t5409,t5416,t5420,t5424,t5429,t543,t5430,t5434,t5435,t5436,t5439,t544,t5440,t5441,t5445,t5449,t545,t5450,t5451,t5452,t5453,t5455,t5456,t5457,t546,t5467,t5468,t5469,t547,t5470,t5471,t5472,t5473,t5474,t5475,t5476,t5477,t5478,t548,t5489,t549,t5490,t5493,t5494,t5497,t5499,t5501,t5508,t551,t5510,t5512,t5516,t5517,t552,t5521,t553,t5532,t5535,t554,t5540,t5547,t555,t5557,t5558,t556,t557,t5574,t5578,t5579,t558,t5582,t5586,t559,t5590,t5593,t5596,t560,t5604,t5607,t561,t5612,t562,t5629,t563,t5634,t5635,t564,t567,t568,t5688,t569,t57,t570,t571,t572,t573,t574,t5741,t5743,t576,t577,t5777,t5779,t578,t5780,t5782,t579,t58,t580,t581,t582,t5826,t583,t584,t586,t587,t5886,t5887,t589,t5894,t59,t590,t591,t592,t593,t594,t595,t596,t597,t6,t60,t600,t602,t603,t604,t605,t609,t610,t611,t612,t613,t614,t615,t616,t618,t619,t622,t623,t624,t625,t626,t627,t628,t629,t63,t630,t631,t633,t634,t635,t636,t637,t638,t639,t640,t641,t642,t643,t648,t649,t650,t653,t654,t655,t656,t657,t658,t660,t662,t663,t664,t665,t667,t668,t673,t674,t675,t676,t678,t679,t681,t682,t683,t684,t685,t686,t687,t688,t689,t693,t694,t695,t696,t697,t698,t7,t700,t702,t703,t704,t705,t706,t71,t710,t711,t712,t713,t715,t716,t72,t724,t728,t73,t731,t733,t734,t735,t736,t74,t741,t742,t743,t744,t746,t747,t748,t749,t75,t750,t751,t752,t754,t755,t756,t757,t758,t759,t76,t760,t762,t763,t764,t765,t766,t767,t768,t769,t77,t772,t773,t774,t775,t776,t777,t778,t779,t780,t781,t782,t784,t785,t786,t790,t792,t794,t795,t796,t798,t8,t80,t801,t804,t805,t806,t808,t81,t814,t815,t817,t82,t820,t822,t825,t827,t83,t831,t832,t833,t834,t835,t836,t837,t838,t84,t840,t841,t842,t843,t846,t86,t863,t868,t869,t870,t874,t878,t880,t881,t882,t884,t885,t888,t889,t891,t892,t895,t897,t899,t9,t90,t900,t903,t906,t91,t911,t921,t922,t923,t925,t926,t927,t929,t934,t935,t936,t937,t940,t941,t942,t946,t949,t95,t950,t954,t955,t956,t957,t958,t961,t962,t964,t965,t966,t968,t969,t97,t970,t971,t972,t973,t975,t977,t979,t982,t983,t984,t986,t987,t988,t989,t99,t993,t994,t995,t999});
end
function C_dq = ft_6(ct)
dq1 = ct{1};
dq2 = ct{2};
dq3 = ct{3};
dq4 = ct{4};
dq5 = ct{5};
dq6 = ct{6};
t1003 = ct{7};
t1004 = ct{8};
t1006 = ct{9};
t1008 = ct{10};
t1009 = ct{11};
t101 = ct{12};
t1010 = ct{13};
t1012 = ct{14};
t1013 = ct{15};
t1015 = ct{16};
t1016 = ct{17};
t102 = ct{18};
t1023 = ct{19};
t1024 = ct{20};
t1025 = ct{21};
t1026 = ct{22};
t1027 = ct{23};
t1028 = ct{24};
t1030 = ct{25};
t1032 = ct{26};
t1033 = ct{27};
t1034 = ct{28};
t1038 = ct{29};
t1039 = ct{30};
t1040 = ct{31};
t1041 = ct{32};
t1042 = ct{33};
t1043 = ct{34};
t1044 = ct{35};
t1045 = ct{36};
t1046 = ct{37};
t1047 = ct{38};
t1048 = ct{39};
t1049 = ct{40};
t1050 = ct{41};
t1051 = ct{42};
t1054 = ct{43};
t1055 = ct{44};
t1056 = ct{45};
t1057 = ct{46};
t1059 = ct{47};
t1061 = ct{48};
t1064 = ct{49};
t1065 = ct{50};
t1066 = ct{51};
t1068 = ct{52};
t1069 = ct{53};
t1070 = ct{54};
t1071 = ct{55};
t1073 = ct{56};
t1076 = ct{57};
t1078 = ct{58};
t1080 = ct{59};
t1081 = ct{60};
t1083 = ct{61};
t1084 = ct{62};
t1085 = ct{63};
t1091 = ct{64};
t1092 = ct{65};
t1093 = ct{66};
t1094 = ct{67};
t1095 = ct{68};
t1097 = ct{69};
t1098 = ct{70};
t1099 = ct{71};
t110 = ct{72};
t1100 = ct{73};
t1101 = ct{74};
t1102 = ct{75};
t1105 = ct{76};
t1106 = ct{77};
t1107 = ct{78};
t1108 = ct{79};
t1109 = ct{80};
t111 = ct{81};
t1111 = ct{82};
t1113 = ct{83};
t1115 = ct{84};
t1116 = ct{85};
t1119 = ct{86};
t112 = ct{87};
t1120 = ct{88};
t1122 = ct{89};
t1123 = ct{90};
t1125 = ct{91};
t1126 = ct{92};
t1127 = ct{93};
t1128 = ct{94};
t1129 = ct{95};
t113 = ct{96};
t1130 = ct{97};
t1131 = ct{98};
t1132 = ct{99};
t1133 = ct{100};
t1134 = ct{101};
t1138 = ct{102};
t1139 = ct{103};
t114 = ct{104};
t1140 = ct{105};
t1141 = ct{106};
t1144 = ct{107};
t1146 = ct{108};
t1148 = ct{109};
t115 = ct{110};
t1150 = ct{111};
t1151 = ct{112};
t1152 = ct{113};
t1153 = ct{114};
t1155 = ct{115};
t1158 = ct{116};
t1159 = ct{117};
t116 = ct{118};
t1161 = ct{119};
t1162 = ct{120};
t1163 = ct{121};
t1166 = ct{122};
t1167 = ct{123};
t1169 = ct{124};
t1170 = ct{125};
t1171 = ct{126};
t1173 = ct{127};
t1174 = ct{128};
t1175 = ct{129};
t1176 = ct{130};
t1177 = ct{131};
t1178 = ct{132};
t1179 = ct{133};
t1180 = ct{134};
t1181 = ct{135};
t1182 = ct{136};
t1183 = ct{137};
t1184 = ct{138};
t1185 = ct{139};
t1186 = ct{140};
t1187 = ct{141};
t1188 = ct{142};
t1189 = ct{143};
t1190 = ct{144};
t1191 = ct{145};
t1192 = ct{146};
t1193 = ct{147};
t1195 = ct{148};
t1196 = ct{149};
t1197 = ct{150};
t1198 = ct{151};
t1199 = ct{152};
t120 = ct{153};
t1203 = ct{154};
t1204 = ct{155};
t1205 = ct{156};
t1206 = ct{157};
t1207 = ct{158};
t1208 = ct{159};
t121 = ct{160};
t1210 = ct{161};
t1214 = ct{162};
t1215 = ct{163};
t1216 = ct{164};
t1219 = ct{165};
t1221 = ct{166};
t1222 = ct{167};
t1223 = ct{168};
t1224 = ct{169};
t1225 = ct{170};
t1226 = ct{171};
t1227 = ct{172};
t1228 = ct{173};
t1229 = ct{174};
t1230 = ct{175};
t1232 = ct{176};
t1233 = ct{177};
t1236 = ct{178};
t124 = ct{179};
t1240 = ct{180};
t1242 = ct{181};
t1244 = ct{182};
t1245 = ct{183};
t125 = ct{184};
t1250 = ct{185};
t1251 = ct{186};
t1253 = ct{187};
t1254 = ct{188};
t1256 = ct{189};
t1257 = ct{190};
t1258 = ct{191};
t1259 = ct{192};
t126 = ct{193};
t1260 = ct{194};
t1261 = ct{195};
t1262 = ct{196};
t1263 = ct{197};
t1264 = ct{198};
t1265 = ct{199};
t1266 = ct{200};
t1267 = ct{201};
t1268 = ct{202};
t1269 = ct{203};
t1271 = ct{204};
t1272 = ct{205};
t1273 = ct{206};
t1274 = ct{207};
t1276 = ct{208};
t1277 = ct{209};
t1278 = ct{210};
t1279 = ct{211};
t128 = ct{212};
t1280 = ct{213};
t1282 = ct{214};
t1284 = ct{215};
t1285 = ct{216};
t1286 = ct{217};
t1287 = ct{218};
t1288 = ct{219};
t129 = ct{220};
t1290 = ct{221};
t1293 = ct{222};
t1294 = ct{223};
t1295 = ct{224};
t1296 = ct{225};
t1297 = ct{226};
t1298 = ct{227};
t130 = ct{228};
t1300 = ct{229};
t1301 = ct{230};
t1302 = ct{231};
t1304 = ct{232};
t1306 = ct{233};
t1307 = ct{234};
t1308 = ct{235};
t1309 = ct{236};
t131 = ct{237};
t1312 = ct{238};
t1313 = ct{239};
t1315 = ct{240};
t1316 = ct{241};
t1319 = ct{242};
t132 = ct{243};
t1320 = ct{244};
t1321 = ct{245};
t1322 = ct{246};
t1323 = ct{247};
t1324 = ct{248};
t1325 = ct{249};
t1326 = ct{250};
t1328 = ct{251};
t1329 = ct{252};
t133 = ct{253};
t1330 = ct{254};
t1331 = ct{255};
t1332 = ct{256};
t1333 = ct{257};
t1334 = ct{258};
t1335 = ct{259};
t1337 = ct{260};
t1338 = ct{261};
t1339 = ct{262};
t134 = ct{263};
t1340 = ct{264};
t1341 = ct{265};
t1342 = ct{266};
t1343 = ct{267};
t1344 = ct{268};
t1345 = ct{269};
t1346 = ct{270};
t1347 = ct{271};
t1348 = ct{272};
t1351 = ct{273};
t1352 = ct{274};
t1353 = ct{275};
t1354 = ct{276};
t1355 = ct{277};
t1356 = ct{278};
t1358 = ct{279};
t136 = ct{280};
t1360 = ct{281};
t1362 = ct{282};
t1364 = ct{283};
t1365 = ct{284};
t1366 = ct{285};
t1367 = ct{286};
t1368 = ct{287};
t1369 = ct{288};
t1370 = ct{289};
t1371 = ct{290};
t1372 = ct{291};
t1373 = ct{292};
t1374 = ct{293};
t1375 = ct{294};
t1377 = ct{295};
t1378 = ct{296};
t1379 = ct{297};
t1380 = ct{298};
t1382 = ct{299};
t1383 = ct{300};
t1384 = ct{301};
t1385 = ct{302};
t1386 = ct{303};
t1387 = ct{304};
t1388 = ct{305};
t1389 = ct{306};
t139 = ct{307};
t1391 = ct{308};
t1392 = ct{309};
t1393 = ct{310};
t1394 = ct{311};
t1397 = ct{312};
t1398 = ct{313};
t140 = ct{314};
t1401 = ct{315};
t1402 = ct{316};
t1403 = ct{317};
t1404 = ct{318};
t1405 = ct{319};
t1406 = ct{320};
t1407 = ct{321};
t1408 = ct{322};
t1409 = ct{323};
t141 = ct{324};
t1410 = ct{325};
t1411 = ct{326};
t1413 = ct{327};
t1414 = ct{328};
t1415 = ct{329};
t1416 = ct{330};
t1417 = ct{331};
t1418 = ct{332};
t1419 = ct{333};
t142 = ct{334};
t1421 = ct{335};
t1422 = ct{336};
t1423 = ct{337};
t1424 = ct{338};
t1426 = ct{339};
t1427 = ct{340};
t1428 = ct{341};
t1429 = ct{342};
t143 = ct{343};
t1430 = ct{344};
t1431 = ct{345};
t1432 = ct{346};
t1433 = ct{347};
t1434 = ct{348};
t1436 = ct{349};
t1439 = ct{350};
t144 = ct{351};
t1440 = ct{352};
t1442 = ct{353};
t1443 = ct{354};
t1444 = ct{355};
t1445 = ct{356};
t1447 = ct{357};
t1448 = ct{358};
t1449 = ct{359};
t145 = ct{360};
t1451 = ct{361};
t1452 = ct{362};
t1453 = ct{363};
t1454 = ct{364};
t1455 = ct{365};
t1456 = ct{366};
t1457 = ct{367};
t1458 = ct{368};
t1459 = ct{369};
t1460 = ct{370};
t1461 = ct{371};
t1463 = ct{372};
t1464 = ct{373};
t1467 = ct{374};
t1468 = ct{375};
t1469 = ct{376};
t147 = ct{377};
t1470 = ct{378};
t1471 = ct{379};
t1472 = ct{380};
t1473 = ct{381};
t1474 = ct{382};
t1475 = ct{383};
t1476 = ct{384};
t1478 = ct{385};
t1479 = ct{386};
t148 = ct{387};
t1480 = ct{388};
t1481 = ct{389};
t1482 = ct{390};
t1483 = ct{391};
t1485 = ct{392};
t1486 = ct{393};
t1487 = ct{394};
t1488 = ct{395};
t1489 = ct{396};
t1492 = ct{397};
t1494 = ct{398};
t1496 = ct{399};
t1498 = ct{400};
t1499 = ct{401};
t15 = ct{402};
t150 = ct{403};
t1501 = ct{404};
t1503 = ct{405};
t1505 = ct{406};
t1506 = ct{407};
t1508 = ct{408};
t151 = ct{409};
t1511 = ct{410};
t1513 = ct{411};
t1514 = ct{412};
t1515 = ct{413};
t1517 = ct{414};
t1520 = ct{415};
t1521 = ct{416};
t1522 = ct{417};
t1523 = ct{418};
t1524 = ct{419};
t1527 = ct{420};
t1528 = ct{421};
t1529 = ct{422};
t153 = ct{423};
t1530 = ct{424};
t1531 = ct{425};
t1532 = ct{426};
t1533 = ct{427};
t1534 = ct{428};
t1535 = ct{429};
t1536 = ct{430};
t1537 = ct{431};
t1538 = ct{432};
t1539 = ct{433};
t154 = ct{434};
t1541 = ct{435};
t1542 = ct{436};
t1545 = ct{437};
t1548 = ct{438};
t1549 = ct{439};
t1550 = ct{440};
t1555 = ct{441};
t1556 = ct{442};
t1558 = ct{443};
t156 = ct{444};
t1560 = ct{445};
t1561 = ct{446};
t1562 = ct{447};
t1566 = ct{448};
t1567 = ct{449};
t1568 = ct{450};
t1569 = ct{451};
t157 = ct{452};
t1570 = ct{453};
t1571 = ct{454};
t158 = ct{455};
t1580 = ct{456};
t1587 = ct{457};
t1589 = ct{458};
t1591 = ct{459};
t1593 = ct{460};
t1595 = ct{461};
t1596 = ct{462};
t1597 = ct{463};
t1598 = ct{464};
t1599 = ct{465};
t16 = ct{466};
t1605 = ct{467};
t1606 = ct{468};
t161 = ct{469};
t1610 = ct{470};
t1611 = ct{471};
t1612 = ct{472};
t1619 = ct{473};
t1620 = ct{474};
t1621 = ct{475};
t1622 = ct{476};
t1623 = ct{477};
t1625 = ct{478};
t163 = ct{479};
t1631 = ct{480};
t1632 = ct{481};
t1633 = ct{482};
t1635 = ct{483};
t1636 = ct{484};
t1637 = ct{485};
t1638 = ct{486};
t1639 = ct{487};
t1641 = ct{488};
t1643 = ct{489};
t1644 = ct{490};
t1645 = ct{491};
t165 = ct{492};
t1650 = ct{493};
t1651 = ct{494};
t1652 = ct{495};
t1653 = ct{496};
